simulink library "CryoDetLibCMB"  (R2016b)
settings: Solver=VariableStepAuto  StartTime=0.0  StopTime=10.0  RelTol=1e-3
undefined symbols (not defined in the file): A, B, C, D, Fadc, Fclk, PCIN, xlipgetpartsetting
libraries: xbsIndex_r4 x640, CryoDetLibCMB x81, CryoDetLib x2, simulink x1
(part 2 of 12)

== system CryoDetLibCMB/DAC subSum10_DSP48 ==
  note: Final adder stages
      | divide by 8
      | and reduce to 16 bits
      | add registers to aid timing
  valid : Inport
  In1 : Inport  Port=2
  In2 : Inport  Port=3
  In3 : Inport  Port=4
  In4 : Inport  Port=5
  In5 : Inport  Port=6
  In6 : Inport  Port=7
  In7 : Inport  Port=8
  In8 : Inport  Port=9
  In9 : Inport  Port=10
  In10 : Inport  Port=11
  In11 : Inport  Port=12
  In12 : Inport  Port=13
  In13 : Inport  Port=14
  In14 : Inport  Port=15
  In15 : Inport  Port=16
  In16 : Inport  Port=17
  ch : Inport  Port=18
  r_tone_scale_sel : Inport  Port=19
  Convert1 : xbsIndex_r4/Convert  gui_display_data_type=Fixed-point  arith_type="Signed  (2's comp)"  n_bits=18  bin_pt=17  float_type=Single  exp_bits=8  fraction_bits=24  quantization=Truncate  overflow=Wrap  en=off  latency=0  pipeline=off  dbl_ovrd=off  block_type=convert
  Convert{2..3,5..6} (4 alike) : xbsIndex_r4/Convert  gui_display_data_type=Fixed-point  arith_type="Signed  (2's comp)"  n_bits=19  bin_pt=17  float_type=Single  exp_bits=8  fraction_bits=24  quantization=Truncate  overflow=Wrap  en=off  latency=0  pipeline=off  dbl_ovrd=off  block_type=convert
  Convert4 : xbsIndex_r4/Convert  gui_display_data_type=Fixed-point  arith_type="Signed  (2's comp)"  n_bits=18  bin_pt=17  float_type=Single  exp_bits=8  fraction_bits=24  quantization=Truncate  overflow=Wrap  en=off  latency=0  pipeline=off  dbl_ovrd=off  block_type=convert
  "DSP48 Macro 3.0 " : xbsIndex_r4/DSP48 Macro 3.0   dsptype=Target XtremeDSP Slice: DSP48E2  instruction_list=(A+D)+C  AvailableInstructions=|  show_filtered=off  pipeline_options=Expert  dspimage=?  tier_1=off  tier_2=off  tier_3=off  tier_4=off  tier_5=off  tier_6=off  dreg_1=off  dreg_2=on  dreg_3=on  areg_1=off  areg_2=on  areg_3=on  areg_4=on  breg_1=off  breg_2=off  breg_3=off  breg_4=off  mreg_5=on  concatreg_3=off  concatreg_4=off  concatreg_5=off  creg_1=off  creg_2=on  creg_3=on  creg_4=on  creg_5=on  preg_6=on  cinreg_1=off  cinreg_2=off  cinreg_3=off  cinreg_4=off  cinreg_5=off  opreg_1=off  opreg_2=off  opreg_3=off  opreg_4=off  opreg_5=off  output_properties=Full_Precision  p_width=19  p_binarywidth=15  has_acout=off  has_bcout=off  has_pcout=off  has_carryout=off  has_carrycascout=off  has_ce=off  has_d_ce=off  has_a_ce=off  has_b_ce=off  has_concat_ce=off  has_c_ce=off  has_m_ce=off  has_p_ce=off  has_sel_ce=off  has_sclr=off  has_d_sclr=off  has_a_sclr=off  has_b_sclr=off  has_concat_sclr=off  has_c_sclr=off  has_m_sclr=off  has_p_sclr=off  has_sel_sclr=off  use_dsp48=on  simulation_type=fast_sim  simulation_model=sysgen:xbip_dsp48_macro_v3_0  gui_behaviour=Sysgen  instruction1='#'  ip_name=DSP48 Macro  ip_version=3.0  dsptool_ready=true  ipcore_usecache=true  ipcore_useipmodelcache=true  wrapper_available=true  port_translation_map={ 'ce' => 'en', 'sclr' => 'rst'}  ipcore_latency_function='has_combinational'  structural_sim=false  ipcore_verbose=false  ipcore_port_config={ 'carryin' => { 'arith' => 'ufix', 'binpt' => 0.00000000000, 'width' => 1.00000000000}, 'carrycascin' => { 'arith' => 'ufix', 'binpt' => 0.00000000000, 'width' => 1.00000000000}, 'carrycascout' => { 'arith' => 'ufix', 'binpt' => 0.00000000000, 'width' => 1.00000000000}, 'carryout' => { 'arith' => 'ufix', 'binpt' => 0.00000000000, 'width' => 1.00000000000}}  ipcore_xco_need_fpga_part=true  block_type=xbip_dsp48_macro_v3_0
      | #
      | (A+D)
      | (A+D)*B
      | (A+D)*B+C
      | (A+D)*B+C+C
      | (A+D)*B+C+C+CARRYIN
      | (A+D)*B+C+CARRYIN
      | (A+D)*B+C+P
      | (A+D)*B+C+P+CARRYIN
      | (A+D)*B+C+P>>17
      | (A+D)*B+C+P>>17+CARRYIN
      | (A+D)*B+C+PCIN
      | (A+D)*B+C+PCIN+CARRYIN
      | (A+D)*B+C+PCIN>>17
      | (A+D)*B+C+PCIN>>17+CARRYIN
      | (A+D)*B+C-C
      | (A+D)*B+C-P
      | (A+D)*B+C-P>>17
      | (A+D)*B+C-PCIN
      | (A+D)*B+C-PCIN>>17
      | (A+D)*B+CARRYIN
      | (A+D)*B+P
      | (A+D)*B+P+C
      | (A+D)*B+P+C+CARRYIN
      | (A+D)*B+P+CARRYIN
      | (A+D)*B+P+P
      | (A+D)*B+P+P+CARRYIN
      | (A+D)*B+P+P>>17
      | (A+D)*B+P+P>>17+CARRYIN
      | (A+D)*B+P+PCIN
      | (A+D)*B+P+PCIN+CARRYIN
      | (A+D)*B+P+PCIN>>17
      | (A+D)*B+P+PCIN>>17+CARRYIN
      | (A+D)*B+P-C
      | (A+D)*B+P-P
      | (A+D)*B+P-P>>17
      | (A+D)*B+P-PCIN
      | (A+D)*B+P-PCIN>>17
      | (A+D)*B+P>>17
      | (A+D)*B+P>>17+C
      | (A+D)*B+P>>17+C+CARRYIN
      | (A+D)*B+P>>17+CARRYIN
      | (A+D)*B+P>>17+P
      | (A+D)*B+P>>17+P+CARRYIN
      | (A+D)*B+PCIN
      | (A+D)*B+PCIN+C
      | (A+D)*B+PCIN+C+CARRYIN
      | (A+D)*B+PCIN+CARRYIN
      | (A+D)*B+PCIN+P
      | (A+D)*B+PCIN+P+CARRYIN
      | (A+D)*B+PCIN>>17
      | (A+D)*B+PCIN>>17+C
      | (A+D)*B+PCIN>>17+C+CARRYIN
      | (A+D)*B+PCIN>>17+CARRYIN
      | (A+D)*B+PCIN>>17+P
      | (A+D)*B+PCIN>>17+P+CARRYIN
      | (A+D)*B-C
      | (A+D)*B-P
      | (A+D)*B-P>>17
      | (A+D)*B-PCIN
      | (A+D)*B-PCIN>>17
      | (A+D)+C
      | (A+D)+C+C
      | (A+D)+C+C+CARRYIN
      | (A+D)+C+CARRYIN
      | (A+D)+C+P
      | (A+D)+C+P+CARRYIN
      | (A+D)+C+P>>17
      | (A+D)+C+P>>17+CARRYIN
      | (A+D)+C+PCIN
      | (A+D)+C+PCIN+CARRYIN
      | (A+D)+C+PCIN>>17
      | (A+D)+C+PCIN>>17+CARRYIN
      | (A+D)+C-C
      | (A+D)+C-P
      | (A+D)+C-P>>17
      | (A+D)+C-PCIN
      | (A+D)+C-PCIN>>17
      | (A+D)+CARRYIN
      | (A+D)+P
      | (A+D)+P+C
      | (A+D)+P+C+CARRYIN
      | (A+D)+P+CARRYIN
      | (A+D)+P+P
      | (A+D)+P+P+CARRYIN
      | (A+D)+P+P>>17
      | (A+D)+P+P>>17+CARRYIN
      | (A+D)+P+PCIN
      | (A+D)+P+PCIN+CARRYIN
      | (A+D)+P+PCIN>>17
      | (A+D)+P+PCIN>>17+CARRYIN
      | (A+D)+P-C
      | (A+D)+P-P
      | (A+D)+P-P>>17
      | (A+D)+P-PCIN
      | (A+D)+P-PCIN>>17
      | (A+D)+P>>17
      | (A+D)+P>>17+C
      | (A+D)+P>>17+C+CARRYIN
      | (A+D)+P>>17+CARRYIN
      | (A+D)+P>>17+P
      | (A+D)+P>>17+P+CARRYIN
      | (A+D)+PCIN
      | (A+D)+PCIN+C
      | (A+D)+PCIN+C+CARRYIN
      | (A+D)+PCIN+CARRYIN
      | (A+D)+PCIN+P
      | (A+D)+PCIN+P+CARRYIN
      | (A+D)+PCIN>>17
      | (A+D)+PCIN>>17+C
      | (A+D)+PCIN>>17+C+CARRYIN
      | (A+D)+PCIN>>17+CARRYIN
      | (A+D)+PCIN>>17+P
      | (A+D)+PCIN>>17+P+CARRYIN
      | (A+D)-C
      | (A+D)-P
      | (A+D)-P>>17
      | (A+D)-PCIN
      | (A+D)-PCIN>>17
      | (D+A)
      | (D+A)*B
      | (D+A)*B+C
      | (D+A)*B+C+C
      | (D+A)*B+C+C+CARRYIN
      | (D+A)*B+C+CARRYIN
      | (D+A)*B+C+P
      | (D+A)*B+C+P+CARRYIN
      | (D+A)*B+C+P>>17
      | (D+A)*B+C+P>>17+CARRYIN
      | (D+A)*B+C+PCIN
      | (D+A)*B+C+PCIN+CARRYIN
      | (D+A)*B+C+PCIN>>17
      | (D+A)*B+C+PCIN>>17+CARRYIN
      | (D+A)*B+C-C
      | (D+A)*B+C-P
      | (D+A)*B+C-P>>17
      | (D+A)*B+C-PCIN
      | (D+A)*B+C-PCIN>>17
      | (D+A)*B+CARRYIN
      | (D+A)*B+P
      | (D+A)*B+P+C
      | (D+A)*B+P+C+CARRYIN
      | (D+A)*B+P+CARRYIN
      | (D+A)*B+P+P
      | (D+A)*B+P+P+CARRYIN
      | (D+A)*B+P+P>>17
      | (D+A)*B+P+P>>17+CARRYIN
      | (D+A)*B+P+PCIN
      | (D+A)*B+P+PCIN+CARRYIN
      | (D+A)*B+P+PCIN>>17
      | (D+A)*B+P+PCIN>>17+CARRYIN
      | (D+A)*B+P-C
      | (D+A)*B+P-P
      | (D+A)*B+P-P>>17
      | (D+A)*B+P-PCIN
      | (D+A)*B+P-PCIN>>17
      | (D+A)*B+P>>17
      | (D+A)*B+P>>17+C
      | (D+A)*B+P>>17+C+CARRYIN
      | (D+A)*B+P>>17+CARRYIN
      | (D+A)*B+P>>17+P
      | (D+A)*B+P>>17+P+CARRYIN
      | (D+A)*B+PCIN
      | (D+A)*B+PCIN+C
      | (D+A)*B+PCIN+C+CARRYIN
      | (D+A)*B+PCIN+CARRYIN
      | (D+A)*B+PCIN+P
      | (D+A)*B+PCIN+P+CARRYIN
      | (D+A)*B+PCIN>>17
      | (D+A)*B+PCIN>>17+C
      | (D+A)*B+PCIN>>17+C+CARRYIN
      | (D+A)*B+PCIN>>17+CARRYIN
      | (D+A)*B+PCIN>>17+P
      | (D+A)*B+PCIN>>17+P+CARRYIN
      | (D+A)*B-C
      | (D+A)*B-P
      | (D+A)*B-P>>17
      | (D+A)*B-PCIN
      | (D+A)*B-PCIN>>17
      | (D+A)+C
      | (D+A)+C+C
      | (D+A)+C+C+CARRYIN
      | (D+A)+C+CARRYIN
      | (D+A)+C+P
      | (D+A)+C+P+CARRYIN
      | (D+A)+C+P>>17
      | (D+A)+C+P>>17+CARRYIN
      | (D+A)+C+PCIN
      | (D+A)+C+PCIN+CARRYIN
      | (D+A)+C+PCIN>>17
      | (D+A)+C+PCIN>>17+CARRYIN
      | (D+A)+C-C
      | (D+A)+C-P
      | (D+A)+C-P>>17
      | (D+A)+C-PCIN
      | (D+A)+C-PCIN>>17
      | (D+A)+CARRYIN
      | (D+A)+P
      | (D+A)+P+C
      | (D+A)+P+C+CARRYIN
      | (D+A)+P+CARRYIN
      | (D+A)+P+P
      | (D+A)+P+P+CARRYIN
      | (D+A)+P+P>>17
      | (D+A)+P+P>>17+CARRYIN
      | (D+A)+P+PCIN
      | (D+A)+P+PCIN+CARRYIN
      | (D+A)+P+PCIN>>17
      | (D+A)+P+PCIN>>17+CARRYIN
      | (D+A)+P-C
      | (D+A)+P-P
      | (D+A)+P-P>>17
      | (D+A)+P-PCIN
      | (D+A)+P-PCIN>>17
      | (D+A)+P>>17
      | (D+A)+P>>17+C
      | (D+A)+P>>17+C+CARRYIN
      | (D+A)+P>>17+CARRYIN
      | (D+A)+P>>17+P
      | (D+A)+P>>17+P+CARRYIN
      | (D+A)+PCIN
      | (D+A)+PCIN+C
      | (D+A)+PCIN+C+CARRYIN
      | (D+A)+PCIN+CARRYIN
      | (D+A)+PCIN+P
      | (D+A)+PCIN+P+CARRYIN
      | (D+A)+PCIN>>17
      | (D+A)+PCIN>>17+C
      | (D+A)+PCIN>>17+C+CARRYIN
      | (D+A)+PCIN>>17+CARRYIN
      | (D+A)+PCIN>>17+P
      | (D+A)+PCIN>>17+P+CARRYIN
      | (D+A)-C
      | (D+A)-P
      | (D+A)-P>>17
      | (D+A)-PCIN
      | (D+A)-PCIN>>17
      | (D-A)
      | (D-A)*B
      | (D-A)*B+C
      | (D-A)*B+C+C
      | (D-A)*B+C+C+CARRYIN
      | (D-A)*B+C+CARRYIN
      | (D-A)*B+C+P
      | (D-A)*B+C+P+CARRYIN
      | (D-A)*B+C+P>>17
      | (D-A)*B+C+P>>17+CARRYIN
      | (D-A)*B+C+PCIN
      | (D-A)*B+C+PCIN+CARRYIN
      | (D-A)*B+C+PCIN>>17
      | (D-A)*B+C+PCIN>>17+CARRYIN
      | (D-A)*B+C-C
      | (D-A)*B+C-P
      | (D-A)*B+C-P>>17
      | (D-A)*B+C-PCIN
      | (D-A)*B+C-PCIN>>17
      | (D-A)*B+CARRYIN
      | (D-A)*B+P
      | (D-A)*B+P+C
      | (D-A)*B+P+C+CARRYIN
      | (D-A)*B+P+CARRYIN
      | (D-A)*B+P+P
      | (D-A)*B+P+P+CARRYIN
      | (D-A)*B+P+P>>17
      | (D-A)*B+P+P>>17+CARRYIN
      | (D-A)*B+P+PCIN
      | (D-A)*B+P+PCIN+CARRYIN
      | (D-A)*B+P+PCIN>>17
      | (D-A)*B+P+PCIN>>17+CARRYIN
      | (D-A)*B+P-C
      | (D-A)*B+P-P
      | (D-A)*B+P-P>>17
      | (D-A)*B+P-PCIN
      | (D-A)*B+P-PCIN>>17
      | (D-A)*B+P>>17
      | (D-A)*B+P>>17+C
      | (D-A)*B+P>>17+C+CARRYIN
      | (D-A)*B+P>>17+CARRYIN
      | (D-A)*B+P>>17+P
      | (D-A)*B+P>>17+P+CARRYIN
      | (D-A)*B+PCIN
      | (D-A)*B+PCIN+C
      | (D-A)*B+PCIN+C+CARRYIN
      | (D-A)*B+PCIN+CARRYIN
      | (D-A)*B+PCIN+P
      | (D-A)*B+PCIN+P+CARRYIN
      | (D-A)*B+PCIN>>17
      | (D-A)*B+PCIN>>17+C
      | (D-A)*B+PCIN>>17+C+CARRYIN
      | (D-A)*B+PCIN>>17+CARRYIN
      | (D-A)*B+PCIN>>17+P
      | (D-A)*B+PCIN>>17+P+CARRYIN
      | (D-A)*B-C
      | (D-A)*B-P
      | (D-A)*B-P>>17
      | (D-A)*B-PCIN
      | (D-A)*B-PCIN>>17
      | (D-A)+C
      | (D-A)+C+C
      | (D-A)+C+C+CARRYIN
      | (D-A)+C+CARRYIN
      | (D-A)+C+P
      | (D-A)+C+P+CARRYIN
      | (D-A)+C+P>>17
      | (D-A)+C+P>>17+CARRYIN
      | (D-A)+C+PCIN
      | (D-A)+C+PCIN+CARRYIN
      | (D-A)+C+PCIN>>17
      | (D-A)+C+PCIN>>17+CARRYIN
      | (D-A)+C-C
      | (D-A)+C-P
      | (D-A)+C-P>>17
      | (D-A)+C-PCIN
      | (D-A)+C-PCIN>>17
      | (D-A)+CARRYIN
      | (D-A)+P
      | (D-A)+P+C
      | (D-A)+P+C+CARRYIN
      | (D-A)+P+CARRYIN
      | (D-A)+P+P
      | (D-A)+P+P+CARRYIN
      | (D-A)+P+P>>17
      | (D-A)+P+P>>17+CARRYIN
      | (D-A)+P+PCIN
      | (D-A)+P+PCIN+CARRYIN
      | (D-A)+P+PCIN>>17
      | (D-A)+P+PCIN>>17+CARRYIN
      | (D-A)+P-C
      | (D-A)+P-P
      | (D-A)+P-P>>17
      | (D-A)+P-PCIN
      | (D-A)+P-PCIN>>17
      | (D-A)+P>>17
      | (D-A)+P>>17+C
      | (D-A)+P>>17+C+CARRYIN
      | (D-A)+P>>17+CARRYIN
      | (D-A)+P>>17+P
      | (D-A)+P>>17+P+CARRYIN
      | (D-A)+PCIN
      | (D-A)+PCIN+C
      | (D-A)+PCIN+C+CARRYIN
      | (D-A)+PCIN+CARRYIN
      | (D-A)+PCIN+P
      | (D-A)+PCIN+P+CARRYIN
      | (D-A)+PCIN>>17
      | (D-A)+PCIN>>17+C
      | (D-A)+PCIN>>17+C+CARRYIN
      | (D-A)+PCIN>>17+CARRYIN
      | (D-A)+PCIN>>17+P
      | (D-A)+PCIN>>17+P+CARRYIN
      | (D-A)-C
      | (D-A)-P
      | (D-A)-P>>17
      | (D-A)-PCIN
      | (D-A)-PCIN>>17
      | -((A+D))
      | -((A+D)*B)
      | -((A+D)*B+C)
      | -((A+D)*B+C+CARRYIN)
      | -((A+D)*B+CARRYIN)
      | -((A+D)*B+P)
      | -((A+D)*B+P+CARRYIN)
      | -((A+D)+C)
      | -((A+D)+C+CARRYIN)
      | -((A+D)+CARRYIN)
      | -((A+D)+P)
      | -((A+D)+P+CARRYIN)
      | -((D+A))
      | -((D+A)*B)
      | -((D+A)*B+C)
      | -((D+A)*B+C+CARRYIN)
      | -((D+A)*B+CARRYIN)
      | -((D+A)*B+P)
      | -((D+A)*B+P+CARRYIN)
      | -((D+A)+C)
      | -((D+A)+C+CARRYIN)
      | -((D+A)+CARRYIN)
      | -((D+A)+P)
      | -((D+A)+P+CARRYIN)
      | -((D-A))
      | -((D-A)*B)
      | -((D-A)*B+C)
      | -((D-A)*B+C+CARRYIN)
      | -((D-A)*B+CARRYIN)
      | -((D-A)*B+P)
      | -((D-A)*B+P+CARRYIN)
      | -((D-A)+C)
      | -((D-A)+C+CARRYIN)
      | -((D-A)+CARRYIN)
      | -((D-A)+P)
      | -((D-A)+P+CARRYIN)
      | -(A)
      | -(A*B)
      | -(A*B+C)
      | -(A*B+C+CARRYIN)
      | -(A*B+CARRYIN)
      | -(A*B+P)
      | -(A*B+P+CARRYIN)
      | -(A+C)
      | -(A+C+CARRYIN)
      | -(A+CARRYIN)
      | -(A+D)
      | -(A+D)*B
      | -(A+D)*B-C
      | -(A+D)*B-C-CARRYIN
      | -(A+D)*B-CARRYIN
      | -(A+D)*B-P
      | -(A+D)*B-P-CARRYIN
      | -(A+D)-C
      | -(A+D)-C-CARRYIN
      | -(A+D)-CARRYIN
      | -(A+D)-P
      | -(A+D)-P-CARRYIN
      | -(A+P)
      | -(A+P+CARRYIN)
      | -(B*(A+D))
      | -(B*(A+D)+C)
      | -(B*(A+D)+C+CARRYIN)
      | -(B*(A+D)+CARRYIN)
      | -(B*(A+D)+P)
      | -(B*(A+D)+P+CARRYIN)
      | -(B*(D+A))
      | -(B*(D+A)+C)
      | -(B*(D+A)+C+CARRYIN)
      | -(B*(D+A)+CARRYIN)
      | -(B*(D+A)+P)
      | -(B*(D+A)+P+CARRYIN)
      | -(B*(D-A))
      | -(B*(D-A)+C)
      | -(B*(D-A)+C+CARRYIN)
      | -(B*(D-A)+CARRYIN)
      | -(B*(D-A)+P)
      | -(B*(D-A)+P+CARRYIN)
      | -(B*A)
      | -(B*A+C)
      | -(B*A+C+CARRYIN)
      | -(B*A+CARRYIN)
      | -(B*A+P)
      | -(B*A+P+CARRYIN)
      | -(B*D)
      | -(B*D+C)
      | -(B*D+C+CARRYIN)
      | -(B*D+CARRYIN)
      | -(B*D+P)
      | -(B*D+P+CARRYIN)
      | -(C)
      | -(C+(A+D))
      | -(C+(A+D)*B)
      | -(C+(A+D)*B+CARRYIN)
      | -(C+(A+D)+CARRYIN)
      | -(C+(D+A))
      | -(C+(D+A)*B)
      | -(C+(D+A)*B+CARRYIN)
      | -(C+(D+A)+CARRYIN)
      | -(C+(D-A))
      | -(C+(D-A)*B)
      | -(C+(D-A)*B+CARRYIN)
      | -(C+(D-A)+CARRYIN)
      | -(C+A)
      | -(C+A*B)
      | -(C+A*B+CARRYIN)
      | -(C+A+CARRYIN)
      | -(C+B*(A+D))
      | -(C+B*(A+D)+CARRYIN)
      | -(C+B*(D+A))
      | -(C+B*(D+A)+CARRYIN)
      | -(C+B*(D-A))
      | -(C+B*(D-A)+CARRYIN)
      | -(C+B*A)
      | -(C+B*A+CARRYIN)
      | -(C+B*D)
      | -(C+B*D+CARRYIN)
      | -(C+C)
      | -(C+C+CARRYCASCIN)
      | -(C+C+CARRYIN)
      | -(C+C+P)
      | -(C+C+P+CARRYIN)
      | -(C+CARRYCASCIN)
      | -(C+CARRYIN)
      | -(C+D)
      | -(C+D*B)
      | -(C+D*B+CARRYIN)
      | -(C+D+CARRYIN)
      | -(C+P)
      | -(C+P+C)
      | -(C+P+C+CARRYIN)
      | -(C+P+CARRYCASCIN)
      | -(C+P+CARRYIN)
      | -(C+P+P)
      | -(C+P+P+CARRYIN)
      | -(CARRYIN)
      | -(D)
      | -(D*B)
      | -(D*B+C)
      | -(D*B+C+CARRYIN)
      | -(D*B+CARRYIN)
      | -(D*B+P)
      | -(D*B+P+CARRYIN)
      | -(D+A)
      | -(D+A)*B
      | -(D+A)*B-C
      | -(D+A)*B-C-CARRYIN
      | -(D+A)*B-CARRYIN
      | -(D+A)*B-P
      | -(D+A)*B-P-CARRYIN
      | -(D+A)-C
      | -(D+A)-C-CARRYIN
      | -(D+A)-CARRYIN
      | -(D+A)-P
      | -(D+A)-P-CARRYIN
      | -(D+C)
      | -(D+C+CARRYIN)
      | -(D+CARRYIN)
      | -(D+P)
      | -(D+P+CARRYIN)
      | -(D-A)
      | -(D-A)*B
      | -(D-A)*B-C
      | -(D-A)*B-C-CARRYIN
      | -(D-A)*B-CARRYIN
      | -(D-A)*B-P
      | -(D-A)*B-P-CARRYIN
      | -(D-A)-C
      | -(D-A)-C-CARRYIN
      | -(D-A)-CARRYIN
      | -(D-A)-P
      | -(D-A)-P-CARRYIN
      | -(P)
      | -(P+(A+D))
      | -(P+(A+D)*B)
      | -(P+(A+D)*B+CARRYIN)
      | -(P+(A+D)+CARRYIN)
      | -(P+(D+A))
      | -(P+(D+A)*B)
      | -(P+(D+A)*B+CARRYIN)
      | -(P+(D+A)+CARRYIN)
      | -(P+(D-A))
      | -(P+(D-A)*B)
      | -(P+(D-A)*B+CARRYIN)
      | -(P+(D-A)+CARRYIN)
      | -(P+A)
      | -(P+A*B)
      | -(P+A*B+CARRYIN)
      | -(P+A+CARRYIN)
      | -(P+B*(A+D))
      | -(P+B*(A+D)+CARRYIN)
      | -(P+B*(D+A))
      | -(P+B*(D+A)+CARRYIN)
      | -(P+B*(D-A))
      | -(P+B*(D-A)+CARRYIN)
      | -(P+B*A)
      | -(P+B*A+CARRYIN)
      | -(P+B*D)
      | -(P+B*D+CARRYIN)
      | -(P+C)
      | -(P+C+C)
      | -(P+C+C+CARRYIN)
      | -(P+C+CARRYCASCIN)
      | -(P+C+CARRYIN)
      | -(P+C+P)
      | -(P+C+P+CARRYIN)
      | -(P+CARRYCASCIN)
      | -(P+CARRYIN)
      | -(P+D)
      | -(P+D*B)
      | -(P+D*B+CARRYIN)
      | -(P+D+CARRYIN)
      | -(P+P)
      | -(P+P+C)
      | -(P+P+C+CARRYIN)
      | -(P+P+CARRYCASCIN)
      | -(P+P+CARRYIN)
      | -A
      | -A*B
      | -A*B-C
      | -A*B-C-CARRYIN
      | -A*B-CARRYIN
      | -A*B-P
      | -A*B-P-CARRYIN
      | -A-C
      | -A-C-CARRYIN
      | -A-CARRYIN
      | -A-P
      | -A-P-CARRYIN
      | -B*(A+D)
      | -B*(A+D)-C
      | -B*(A+D)-C-CARRYIN
      | -B*(A+D)-CARRYIN
      | -B*(A+D)-P
      | -B*(A+D)-P-CARRYIN
      | -B*(D+A)
      | -B*(D+A)-C
      | -B*(D+A)-C-CARRYIN
      | -B*(D+A)-CARRYIN
      | -B*(D+A)-P
      | -B*(D+A)-P-CARRYIN
      | -B*(D-A)
      | -B*(D-A)-C
      | -B*(D-A)-C-CARRYIN
      | -B*(D-A)-CARRYIN
      | -B*(D-A)-P
      | -B*(D-A)-P-CARRYIN
      | -B*A
      | -B*A-C
      | -B*A-C-CARRYIN
      | -B*A-CARRYIN
      | -B*A-P
      | -B*A-P-CARRYIN
      | -B*D
      | -B*D-C
      | -B*D-C-CARRYIN
      | -B*D-CARRYIN
      | -B*D-P
      | -B*D-P-CARRYIN
      | -C
      | -C+(A+D)
      | -C+(A+D)*B
      | -C+(A+D)*B+C
      | -C+(A+D)*B+P
      | -C+(A+D)+C
      | -C+(A+D)+P
      | -C+(D+A)
      | -C+(D+A)*B
      | -C+(D+A)*B+C
      | -C+(D+A)*B+P
      | -C+(D+A)+C
      | -C+(D+A)+P
      | -C+(D-A)
      | -C+(D-A)*B
      | -C+(D-A)*B+C
      | -C+(D-A)*B+P
      | -C+(D-A)+C
      | -C+(D-A)+P
      | -C+A
      | -C+A*B
      | -C+A*B+C
      | -C+A*B+P
      | -C+A+C
      | -C+A+P
      | -C+B*(A+D)
      | -C+B*(A+D)+C
      | -C+B*(A+D)+P
      | -C+B*(D+A)
      | -C+B*(D+A)+C
      | -C+B*(D+A)+P
      | -C+B*(D-A)
      | -C+B*(D-A)+C
      | -C+B*(D-A)+P
      | -C+B*A
      | -C+B*A+C
      | -C+B*A+P
      | -C+B*D
      | -C+B*D+C
      | -C+B*D+P
      | -C+C
      | -C+C+(A+D)
      | -C+C+(A+D)*B
      | -C+C+(D+A)
      | -C+C+(D+A)*B
      | -C+C+(D-A)
      | -C+C+(D-A)*B
      | -C+C+A
      | -C+C+A*B
      | -C+C+B*(A+D)
      | -C+C+B*(D+A)
      | -C+C+B*(D-A)
      | -C+C+B*A
      | -C+C+B*D
      | -C+C+C
      | -C+C+C+P
      | -C+C+D
      | -C+C+D*B
      | -C+C+P
      | -C+C+P+C
      | -C+C+P+P
      | -C+D
      | -C+D*B
      | -C+D*B+C
      | -C+D*B+P
      | -C+D+C
      | -C+D+P
      | -C+P
      | -C+P+(A+D)
      | -C+P+(A+D)*B
      | -C+P+(D+A)
      | -C+P+(D+A)*B
      | -C+P+(D-A)
      | -C+P+(D-A)*B
      | -C+P+A
      | -C+P+A*B
      | -C+P+B*(A+D)
      | -C+P+B*(D+A)
      | -C+P+B*(D-A)
      | -C+P+B*A
      | -C+P+B*D
      | -C+P+C
      | -C+P+C+C
      | -C+P+C+P
      | -C+P+D
      | -C+P+D*B
      | -C+P+P
      | -C+P+P+C
      | -C-((A+D))
      | -C-((A+D)*B)
      | -C-((D+A))
      | -C-((D+A)*B)
      | -C-((D-A))
      | -C-((D-A)*B)
      | -C-(A)
      | -C-(A*B)
      | -C-(A+D)
      | -C-(A+D)*B
      | -C-(A+D)*B-CARRYIN
      | -C-(A+D)-CARRYIN
      | -C-(B*(A+D))
      | -C-(B*(D+A))
      | -C-(B*(D-A))
      | -C-(B*A)
      | -C-(B*D)
      | -C-(D)
      | -C-(D*B)
      | -C-(D+A)
      | -C-(D+A)*B
      | -C-(D+A)*B-CARRYIN
      | -C-(D+A)-CARRYIN
      | -C-(D-A)
      | -C-(D-A)*B
      | -C-(D-A)*B-CARRYIN
      | -C-(D-A)-CARRYIN
      | -C-A
      | -C-A*B
      | -C-A*B-CARRYIN
      | -C-A-CARRYIN
      | -C-B*(A+D)
      | -C-B*(A+D)-CARRYIN
      | -C-B*(D+A)
      | -C-B*(D+A)-CARRYIN
      | -C-B*(D-A)
      | -C-B*(D-A)-CARRYIN
      | -C-B*A
      | -C-B*A-CARRYIN
      | -C-B*D
      | -C-B*D-CARRYIN
      | -C-C
      | -C-C-CARRYCASCIN
      | -C-C-CARRYIN
      | -C-C-P
      | -C-C-P-CARRYIN
      | -C-CARRYCASCIN
      | -C-CARRYIN
      | -C-D
      | -C-D*B
      | -C-D*B-CARRYIN
      | -C-D-CARRYIN
      | -C-P
      | -C-P-C
      | -C-P-C-CARRYIN
      | -C-P-CARRYCASCIN
      | -C-P-CARRYIN
      | -C-P-P
      | -C-P-P-CARRYIN
      | -C-P-P>>17
      | -C-P-PCIN
      | -C-P-PCIN>>17
      | -C-P>>17
      | -C-PCIN
      | -C-PCIN>>17
      | -CARRYIN
      | -D
      | -D*B
      | -D*B-C
      | -D*B-C-CARRYIN
      | -D*B-CARRYIN
      | -D*B-P
      | -D*B-P-CARRYIN
      | -D-C
      | -D-C-CARRYIN
      | -D-CARRYIN
      | -D-P
      | -D-P-CARRYIN
      | -P
      | -P+(A+D)
      | -P+(A+D)*B
      | -P+(A+D)*B+C
      | -P+(A+D)*B+P
      | -P+(A+D)+C
      | -P+(A+D)+P
      | -P+(D+A)
      | -P+(D+A)*B
      | -P+(D+A)*B+C
      | -P+(D+A)*B+P
      | -P+(D+A)+C
      | -P+(D+A)+P
      | -P+(D-A)
      | -P+(D-A)*B
      | -P+(D-A)*B+C
      | -P+(D-A)*B+P
      | -P+(D-A)+C
      | -P+(D-A)+P
      | -P+A
      | -P+A*B
      | -P+A*B+C
      | -P+A*B+P
      | -P+A+C
      | -P+A+P
      | -P+B*(A+D)
      | -P+B*(A+D)+C
      | -P+B*(A+D)+P
      | -P+B*(D+A)
      | -P+B*(D+A)+C
      | -P+B*(D+A)+P
      | -P+B*(D-A)
      | -P+B*(D-A)+C
      | -P+B*(D-A)+P
      | -P+B*A
      | -P+B*A+C
      | -P+B*A+P
      | -P+B*D
      | -P+B*D+C
      | -P+B*D+P
      | -P+C
      | -P+C+(A+D)
      | -P+C+(A+D)*B
      | -P+C+(D+A)
      | -P+C+(D+A)*B
      | -P+C+(D-A)
      | -P+C+(D-A)*B
      | -P+C+A
      | -P+C+A*B
      | -P+C+B*(A+D)
      | -P+C+B*(D+A)
      | -P+C+B*(D-A)
      | -P+C+B*A
      | -P+C+B*D
      | -P+C+C
      | -P+C+C+P
      | -P+C+D
      | -P+C+D*B
      | -P+C+P
      | -P+C+P+C
      | -P+C+P+P
      | -P+D
      | -P+D*B
      | -P+D*B+C
      | -P+D*B+P
      | -P+D+C
      | -P+D+P
      | -P+P
      | -P+P+(A+D)
      | -P+P+(A+D)*B
      | -P+P+(D+A)
      | -P+P+(D+A)*B
      | -P+P+(D-A)
      | -P+P+(D-A)*B
      | -P+P+A
      | -P+P+A*B
      | -P+P+B*(A+D)
      | -P+P+B*(D+A)
      | -P+P+B*(D-A)
      | -P+P+B*A
      | -P+P+B*D
      | -P+P+C
      | -P+P+C+C
      | -P+P+C+P
      | -P+P+D
      | -P+P+D*B
      | -P+P+P
      | -P+P+P+C
      | -P-((A+D))
      | -P-((A+D)*B)
      | -P-((D+A))
      | -P-((D+A)*B)
      | -P-((D-A))
      | -P-((D-A)*B)
      | -P-(A)
      | -P-(A*B)
      | -P-(A+D)
      | -P-(A+D)*B
      | -P-(A+D)*B-CARRYIN
      | -P-(A+D)-CARRYIN
      | -P-(B*(A+D))
      | -P-(B*(D+A))
      | -P-(B*(D-A))
      | -P-(B*A)
      | -P-(B*D)
      | -P-(D)
      | -P-(D*B)
      | -P-(D+A)
      | -P-(D+A)*B
      | -P-(D+A)*B-CARRYIN
      | -P-(D+A)-CARRYIN
      | -P-(D-A)
      | -P-(D-A)*B
      | -P-(D-A)*B-CARRYIN
      | -P-(D-A)-CARRYIN
      | -P-A
      | -P-A*B
      | -P-A*B-CARRYIN
      | -P-A-CARRYIN
      | -P-B*(A+D)
      | -P-B*(A+D)-CARRYIN
      | -P-B*(D+A)
      | -P-B*(D+A)-CARRYIN
      | -P-B*(D-A)
      | -P-B*(D-A)-CARRYIN
      | -P-B*A
      | -P-B*A-CARRYIN
      | -P-B*D
      | -P-B*D-CARRYIN
      | -P-C
      | -P-C-C
      | -P-C-C-CARRYIN
      | -P-C-CARRYCASCIN
      | -P-C-CARRYIN
      | -P-C-P
      | -P-C-P-CARRYIN
      | -P-C-P>>17
      | -P-C-PCIN
      | -P-C-PCIN>>17
      | -P-CARRYCASCIN
      | -P-CARRYIN
      | -P-D
      | -P-D*B
      | -P-D*B-CARRYIN
      | -P-D-CARRYIN
      | -P-P
      | -P-P-C
      | -P-P-C-CARRYIN
      | -P-P-CARRYCASCIN
      | -P-P-CARRYIN
      | -P-P-P
      | -P-P-P>>17
      | -P-P-PCIN
      | -P-P-PCIN>>17
      | -P-P>>17
      | -P-PCIN
      | -P-PCIN>>17
      | -P>>17
      | -P>>17+(A+D)
      | -P>>17+(A+D)*B
      | -P>>17+(A+D)*B+C
      | -P>>17+(A+D)*B+P
      | -P>>17+(A+D)+C
      | -P>>17+(A+D)+P
      | -P>>17+(D+A)
      | -P>>17+(D+A)*B
      | -P>>17+(D+A)*B+C
      | -P>>17+(D+A)*B+P
      | -P>>17+(D+A)+C
      | -P>>17+(D+A)+P
      | -P>>17+(D-A)
      | -P>>17+(D-A)*B
      | -P>>17+(D-A)*B+C
      | -P>>17+(D-A)*B+P
      | -P>>17+(D-A)+C
      | -P>>17+(D-A)+P
      | -P>>17+A
      | -P>>17+A*B
      | -P>>17+A*B+C
      | -P>>17+A*B+P
      | -P>>17+A+C
      | -P>>17+A+P
      | -P>>17+B*(A+D)
      | -P>>17+B*(A+D)+C
      | -P>>17+B*(A+D)+P
      | -P>>17+B*(D+A)
      | -P>>17+B*(D+A)+C
      | -P>>17+B*(D+A)+P
      | -P>>17+B*(D-A)
      | -P>>17+B*(D-A)+C
      | -P>>17+B*(D-A)+P
      | -P>>17+B*A
      | -P>>17+B*A+C
      | -P>>17+B*A+P
      | -P>>17+B*D
      | -P>>17+B*D+C
      | -P>>17+B*D+P
      | -P>>17+C
      | -P>>17+C+(A+D)
      | -P>>17+C+(A+D)*B
      | -P>>17+C+(D+A)
      | -P>>17+C+(D+A)*B
      | -P>>17+C+(D-A)
      | -P>>17+C+(D-A)*B
      | -P>>17+C+A
      | -P>>17+C+A*B
      | -P>>17+C+B*(A+D)
      | -P>>17+C+B*(D+A)
      | -P>>17+C+B*(D-A)
      | -P>>17+C+B*A
      | -P>>17+C+B*D
      | -P>>17+C+C
      | -P>>17+C+C+P
      | -P>>17+C+D
      | -P>>17+C+D*B
      | -P>>17+C+P
      | -P>>17+C+P+C
      | -P>>17+C+P+P
      | -P>>17+D
      | -P>>17+D*B
      | -P>>17+D*B+C
      | -P>>17+D*B+P
      | -P>>17+D+C
      | -P>>17+D+P
      | -P>>17+P
      | -P>>17+P+(A+D)
      | -P>>17+P+(A+D)*B
      | -P>>17+P+(D+A)
      | -P>>17+P+(D+A)*B
      | -P>>17+P+(D-A)
      | -P>>17+P+(D-A)*B
      | -P>>17+P+A
      | -P>>17+P+A*B
      | -P>>17+P+B*(A+D)
      | -P>>17+P+B*(D+A)
      | -P>>17+P+B*(D-A)
      | -P>>17+P+B*A
      | -P>>17+P+B*D
      | -P>>17+P+C
      | -P>>17+P+C+C
      | -P>>17+P+C+P
      | -P>>17+P+D
      | -P>>17+P+D*B
      | -P>>17+P+P
      | -P>>17+P+P+C
      | -P>>17-((A+D))
      | -P>>17-((A+D)*B)
      | -P>>17-((D+A))
      | -P>>17-((D+A)*B)
      | -P>>17-((D-A))
      | -P>>17-((D-A)*B)
      | -P>>17-(A)
      | -P>>17-(A*B)
      | -P>>17-(B*(A+D))
      | -P>>17-(B*(D+A))
      | -P>>17-(B*(D-A))
      | -P>>17-(B*A)
      | -P>>17-(B*D)
      | -P>>17-(D)
      | -P>>17-(D*B)
      | -PCIN
      | -PCIN+(A+D)
      | -PCIN+(A+D)*B
      | -PCIN+(A+D)*B+C
      | -PCIN+(A+D)*B+P
      | -PCIN+(A+D)+C
      | -PCIN+(A+D)+P
      | -PCIN+(D+A)
      | -PCIN+(D+A)*B
      | -PCIN+(D+A)*B+C
      | -PCIN+(D+A)*B+P
      | -PCIN+(D+A)+C
      | -PCIN+(D+A)+P
      | -PCIN+(D-A)
      | -PCIN+(D-A)*B
      | -PCIN+(D-A)*B+C
      | -PCIN+(D-A)*B+P
      | -PCIN+(D-A)+C
      | -PCIN+(D-A)+P
      | -PCIN+A
      | -PCIN+A*B
      | -PCIN+A*B+C
      | -PCIN+A*B+P
      | -PCIN+A+C
      | -PCIN+A+P
      | -PCIN+B*(A+D)
      | -PCIN+B*(A+D)+C
      | -PCIN+B*(A+D)+P
      | -PCIN+B*(D+A)
      | -PCIN+B*(D+A)+C
      | -PCIN+B*(D+A)+P
      | -PCIN+B*(D-A)
      | -PCIN+B*(D-A)+C
      | -PCIN+B*(D-A)+P
      | -PCIN+B*A
      | -PCIN+B*A+C
      | -PCIN+B*A+P
      | -PCIN+B*D
      | -PCIN+B*D+C
      | -PCIN+B*D+P
      | -PCIN+C
      | -PCIN+C+(A+D)
      | -PCIN+C+(A+D)*B
      | -PCIN+C+(D+A)
      | -PCIN+C+(D+A)*B
      | -PCIN+C+(D-A)
      | -PCIN+C+(D-A)*B
      | -PCIN+C+A
      | -PCIN+C+A*B
      | -PCIN+C+B*(A+D)
      | -PCIN+C+B*(D+A)
      | -PCIN+C+B*(D-A)
      | -PCIN+C+B*A
      | -PCIN+C+B*D
      | -PCIN+C+C
      | -PCIN+C+C+P
      | -PCIN+C+D
      | -PCIN+C+D*B
      | -PCIN+C+P
      | -PCIN+C+P+C
      | -PCIN+C+P+P
      | -PCIN+D
      | -PCIN+D*B
      | -PCIN+D*B+C
      | -PCIN+D*B+P
      | -PCIN+D+C
      | -PCIN+D+P
      | -PCIN+P
      | -PCIN+P+(A+D)
      | -PCIN+P+(A+D)*B
      | -PCIN+P+(D+A)
      | -PCIN+P+(D+A)*B
      | -PCIN+P+(D-A)
      | -PCIN+P+(D-A)*B
      | -PCIN+P+A
      | -PCIN+P+A*B
      | -PCIN+P+B*(A+D)
      | -PCIN+P+B*(D+A)
      | -PCIN+P+B*(D-A)
      | -PCIN+P+B*A
      | -PCIN+P+B*D
      | -PCIN+P+C
      | -PCIN+P+C+C
      | -PCIN+P+C+P
      | -PCIN+P+D
      | -PCIN+P+D*B
      | -PCIN+P+P
      | -PCIN+P+P+C
      | -PCIN-((A+D))
      | -PCIN-((A+D)*B)
      | -PCIN-((D+A))
      | -PCIN-((D+A)*B)
      | -PCIN-((D-A))
      | -PCIN-((D-A)*B)
      | -PCIN-(A)
      | -PCIN-(A*B)
      | -PCIN-(B*(A+D))
      | -PCIN-(B*(D+A))
      | -PCIN-(B*(D-A))
      | -PCIN-(B*A)
      | -PCIN-(B*D)
      | -PCIN-(D)
      | -PCIN-(D*B)
      | -PCIN>>17
      | -PCIN>>17+(A+D)
      | -PCIN>>17+(A+D)*B
      | -PCIN>>17+(A+D)*B+C
      | -PCIN>>17+(A+D)*B+P
      | -PCIN>>17+(A+D)+C
      | -PCIN>>17+(A+D)+P
      | -PCIN>>17+(D+A)
      | -PCIN>>17+(D+A)*B
      | -PCIN>>17+(D+A)*B+C
      | -PCIN>>17+(D+A)*B+P
      | -PCIN>>17+(D+A)+C
      | -PCIN>>17+(D+A)+P
      | -PCIN>>17+(D-A)
      | -PCIN>>17+(D-A)*B
      | -PCIN>>17+(D-A)*B+C
      | -PCIN>>17+(D-A)*B+P
      | -PCIN>>17+(D-A)+C
      | -PCIN>>17+(D-A)+P
      | -PCIN>>17+A
      | -PCIN>>17+A*B
      | -PCIN>>17+A*B+C
      | -PCIN>>17+A*B+P
      | -PCIN>>17+A+C
      | -PCIN>>17+A+P
      | -PCIN>>17+B*(A+D)
      | -PCIN>>17+B*(A+D)+C
      | -PCIN>>17+B*(A+D)+P
      | -PCIN>>17+B*(D+A)
      | -PCIN>>17+B*(D+A)+C
      | -PCIN>>17+B*(D+A)+P
      | -PCIN>>17+B*(D-A)
      | -PCIN>>17+B*(D-A)+C
      | -PCIN>>17+B*(D-A)+P
      | -PCIN>>17+B*A
      | -PCIN>>17+B*A+C
      | -PCIN>>17+B*A+P
      | -PCIN>>17+B*D
      | -PCIN>>17+B*D+C
      | -PCIN>>17+B*D+P
      | -PCIN>>17+C
      | -PCIN>>17+C+(A+D)
      | -PCIN>>17+C+(A+D)*B
      | -PCIN>>17+C+(D+A)
      | -PCIN>>17+C+(D+A)*B
      | -PCIN>>17+C+(D-A)
      | -PCIN>>17+C+(D-A)*B
      | -PCIN>>17+C+A
      | -PCIN>>17+C+A*B
      | -PCIN>>17+C+B*(A+D)
      | -PCIN>>17+C+B*(D+A)
      | -PCIN>>17+C+B*(D-A)
      | -PCIN>>17+C+B*A
      | -PCIN>>17+C+B*D
      | -PCIN>>17+C+C
      | -PCIN>>17+C+C+P
      | -PCIN>>17+C+D
      | -PCIN>>17+C+D*B
      | -PCIN>>17+C+P
      | -PCIN>>17+C+P+C
      | -PCIN>>17+C+P+P
      | -PCIN>>17+D
      | -PCIN>>17+D*B
      | -PCIN>>17+D*B+C
      | -PCIN>>17+D*B+P
      | -PCIN>>17+D+C
      | -PCIN>>17+D+P
      | -PCIN>>17+P
      | -PCIN>>17+P+(A+D)
      | -PCIN>>17+P+(A+D)*B
      | -PCIN>>17+P+(D+A)
      | -PCIN>>17+P+(D+A)*B
      | -PCIN>>17+P+(D-A)
      | -PCIN>>17+P+(D-A)*B
      | -PCIN>>17+P+A
      | -PCIN>>17+P+A*B
      | -PCIN>>17+P+B*(A+D)
      | -PCIN>>17+P+B*(D+A)
      | -PCIN>>17+P+B*(D-A)
      | -PCIN>>17+P+B*A
      | -PCIN>>17+P+B*D
      | -PCIN>>17+P+C
      | -PCIN>>17+P+C+C
      | -PCIN>>17+P+C+P
      | -PCIN>>17+P+D
      | -PCIN>>17+P+D*B
      | -PCIN>>17+P+P
      | -PCIN>>17+P+P+C
      | -PCIN>>17-((A+D))
      | -PCIN>>17-((A+D)*B)
      | -PCIN>>17-((D+A))
      | -PCIN>>17-((D+A)*B)
      | -PCIN>>17-((D-A))
      | -PCIN>>17-((D-A)*B)
      | -PCIN>>17-(A)
      | -PCIN>>17-(A*B)
      | -PCIN>>17-(B*(A+D))
      | -PCIN>>17-(B*(D+A))
      | -PCIN>>17-(B*(D-A))
      | -PCIN>>17-(B*A)
      | -PCIN>>17-(B*D)
      | -PCIN>>17-(D)
      | -PCIN>>17-(D*B)
      | 0
      | A
      | A*B
      | A*B+C
      | A*B+C+C
      | A*B+C+C+CARRYIN
      | A*B+C+CARRYIN
      | A*B+C+P
      | A*B+C+P+CARRYIN
      | A*B+C+P>>17
      | A*B+C+P>>17+CARRYIN
      | A*B+C+PCIN
      | A*B+C+PCIN+CARRYIN
      | A*B+C+PCIN>>17
      | A*B+C+PCIN>>17+CARRYIN
      | A*B+C-C
      | A*B+C-P
      | A*B+C-P>>17
      | A*B+C-PCIN
      | A*B+C-PCIN>>17
      | A*B+CARRYIN
      | A*B+P
      | A*B+P+C
      | A*B+P+C+CARRYIN
      | A*B+P+CARRYIN
      | A*B+P+P
      | A*B+P+P+CARRYIN
      | A*B+P+P>>17
      | A*B+P+P>>17+CARRYIN
      | A*B+P+PCIN
      | A*B+P+PCIN+CARRYIN
      | A*B+P+PCIN>>17
      | A*B+P+PCIN>>17+CARRYIN
      | A*B+P-C
      | A*B+P-P
      | A*B+P-P>>17
      | A*B+P-PCIN
      | A*B+P-PCIN>>17
      | A*B+P>>17
      | A*B+P>>17+C
      | A*B+P>>17+C+CARRYIN
      | A*B+P>>17+CARRYIN
      | A*B+P>>17+P
      | A*B+P>>17+P+CARRYIN
      | A*B+PCIN
      | A*B+PCIN+C
      | A*B+PCIN+C+CARRYIN
      | A*B+PCIN+CARRYIN
      | A*B+PCIN+P
      | A*B+PCIN+P+CARRYIN
      | A*B+PCIN>>17
      | A*B+PCIN>>17+C
      | A*B+PCIN>>17+C+CARRYIN
      | A*B+PCIN>>17+CARRYIN
      | A*B+PCIN>>17+P
      | A*B+PCIN>>17+P+CARRYIN
      | A*B-C
      | A*B-P
      | A*B-P>>17
      | A*B-PCIN
      | A*B-PCIN>>17
      | A+C
      | A+C+C
      | A+C+C+CARRYIN
      | A+C+CARRYIN
      | A+C+P
      | A+C+P+CARRYIN
      | A+C+P>>17
      | A+C+P>>17+CARRYIN
      | A+C+PCIN
      | A+C+PCIN+CARRYIN
      | A+C+PCIN>>17
      | A+C+PCIN>>17+CARRYIN
      | A+C-C
      | A+C-P
      | A+C-P>>17
      | A+C-PCIN
      | A+C-PCIN>>17
      | A+CARRYIN
      | A+P
      | A+P+C
      | A+P+C+CARRYIN
      | A+P+CARRYIN
      | A+P+P
      | A+P+P+CARRYIN
      | A+P+P>>17
      | A+P+P>>17+CARRYIN
      | A+P+PCIN
      | A+P+PCIN+CARRYIN
      | A+P+PCIN>>17
      | A+P+PCIN>>17+CARRYIN
      | A+P-C
      | A+P-P
      | A+P-P>>17
      | A+P-PCIN
      | A+P-PCIN>>17
      | A+P>>17
      | A+P>>17+C
      | A+P>>17+C+CARRYIN
      | A+P>>17+CARRYIN
      | A+P>>17+P
      | A+P>>17+P+CARRYIN
      | A+PCIN
      | A+PCIN+C
      | A+PCIN+C+CARRYIN
      | A+PCIN+CARRYIN
      | A+PCIN+P
      | A+PCIN+P+CARRYIN
      | A+PCIN>>17
      | A+PCIN>>17+C
      | A+PCIN>>17+C+CARRYIN
      | A+PCIN>>17+CARRYIN
      | A+PCIN>>17+P
      | A+PCIN>>17+P+CARRYIN
      | A-C
      | A-P
      | A-P>>17
      | A-PCIN
      | A-PCIN>>17
      | B*(A+D)
      | B*(A+D)+C
      | B*(A+D)+C+C
      | B*(A+D)+C+C+CARRYIN
      | B*(A+D)+C+CARRYIN
      | B*(A+D)+C+P
      | B*(A+D)+C+P+CARRYIN
      | B*(A+D)+C+P>>17
      | B*(A+D)+C+P>>17+CARRYIN
      | B*(A+D)+C+PCIN
      | B*(A+D)+C+PCIN+CARRYIN
      | B*(A+D)+C+PCIN>>17
      | B*(A+D)+C+PCIN>>17+CARRYIN
      | B*(A+D)+C-C
      | B*(A+D)+C-P
      | B*(A+D)+C-P>>17
      | B*(A+D)+C-PCIN
      | B*(A+D)+C-PCIN>>17
      | B*(A+D)+CARRYIN
      | B*(A+D)+P
      | B*(A+D)+P+C
      | B*(A+D)+P+C+CARRYIN
      | B*(A+D)+P+CARRYIN
      | B*(A+D)+P+P
      | B*(A+D)+P+P+CARRYIN
      | B*(A+D)+P+P>>17
      | B*(A+D)+P+P>>17+CARRYIN
      | B*(A+D)+P+PCIN
      | B*(A+D)+P+PCIN+CARRYIN
      | B*(A+D)+P+PCIN>>17
      | B*(A+D)+P+PCIN>>17+CARRYIN
      | B*(A+D)+P-C
      | B*(A+D)+P-P
      | B*(A+D)+P-P>>17
      | B*(A+D)+P-PCIN
      | B*(A+D)+P-PCIN>>17
      | B*(A+D)+P>>17
      | B*(A+D)+P>>17+C
      | B*(A+D)+P>>17+C+CARRYIN
      | B*(A+D)+P>>17+CARRYIN
      | B*(A+D)+P>>17+P
      | B*(A+D)+P>>17+P+CARRYIN
      | B*(A+D)+PCIN
      | B*(A+D)+PCIN+C
      | B*(A+D)+PCIN+C+CARRYIN
      | B*(A+D)+PCIN+CARRYIN
      | B*(A+D)+PCIN+P
      | B*(A+D)+PCIN+P+CARRYIN
      | B*(A+D)+PCIN>>17
      | B*(A+D)+PCIN>>17+C
      | B*(A+D)+PCIN>>17+C+CARRYIN
      | B*(A+D)+PCIN>>17+CARRYIN
      | B*(A+D)+PCIN>>17+P
      | B*(A+D)+PCIN>>17+P+CARRYIN
      | B*(A+D)-C
      | B*(A+D)-P
      | B*(A+D)-P>>17
      | B*(A+D)-PCIN
      | B*(A+D)-PCIN>>17
      | B*(D+A)
      | B*(D+A)+C
      | B*(D+A)+C+C
      | B*(D+A)+C+C+CARRYIN
      | B*(D+A)+C+CARRYIN
      | B*(D+A)+C+P
      | B*(D+A)+C+P+CARRYIN
      | B*(D+A)+C+P>>17
      | B*(D+A)+C+P>>17+CARRYIN
      | B*(D+A)+C+PCIN
      | B*(D+A)+C+PCIN+CARRYIN
      | B*(D+A)+C+PCIN>>17
      | B*(D+A)+C+PCIN>>17+CARRYIN
      | B*(D+A)+C-C
      | B*(D+A)+C-P
      | B*(D+A)+C-P>>17
      | B*(D+A)+C-PCIN
      | B*(D+A)+C-PCIN>>17
      | B*(D+A)+CARRYIN
      | B*(D+A)+P
      | B*(D+A)+P+C
      | B*(D+A)+P+C+CARRYIN
      | B*(D+A)+P+CARRYIN
      | B*(D+A)+P+P
      | B*(D+A)+P+P+CARRYIN
      | B*(D+A)+P+P>>17
      | B*(D+A)+P+P>>17+CARRYIN
      | B*(D+A)+P+PCIN
      | B*(D+A)+P+PCIN+CARRYIN
      | B*(D+A)+P+PCIN>>17
      | B*(D+A)+P+PCIN>>17+CARRYIN
      | B*(D+A)+P-C
      | B*(D+A)+P-P
      | B*(D+A)+P-P>>17
      | B*(D+A)+P-PCIN
      | B*(D+A)+P-PCIN>>17
      | B*(D+A)+P>>17
      | B*(D+A)+P>>17+C
      | B*(D+A)+P>>17+C+CARRYIN
      | B*(D+A)+P>>17+CARRYIN
      | B*(D+A)+P>>17+P
      | B*(D+A)+P>>17+P+CARRYIN
      | B*(D+A)+PCIN
      | B*(D+A)+PCIN+C
      | B*(D+A)+PCIN+C+CARRYIN
      | B*(D+A)+PCIN+CARRYIN
      | B*(D+A)+PCIN+P
      | B*(D+A)+PCIN+P+CARRYIN
      | B*(D+A)+PCIN>>17
      | B*(D+A)+PCIN>>17+C
      | B*(D+A)+PCIN>>17+C+CARRYIN
      | B*(D+A)+PCIN>>17+CARRYIN
      | B*(D+A)+PCIN>>17+P
      | B*(D+A)+PCIN>>17+P+CARRYIN
      | B*(D+A)-C
      | B*(D+A)-P
      | B*(D+A)-P>>17
      | B*(D+A)-PCIN
      | B*(D+A)-PCIN>>17
      | B*(D-A)
      | B*(D-A)+C
      | B*(D-A)+C+C
      | B*(D-A)+C+C+CARRYIN
      | B*(D-A)+C+CARRYIN
      | B*(D-A)+C+P
      | B*(D-A)+C+P+CARRYIN
      | B*(D-A)+C+P>>17
      | B*(D-A)+C+P>>17+CARRYIN
      | B*(D-A)+C+PCIN
      | B*(D-A)+C+PCIN+CARRYIN
      | B*(D-A)+C+PCIN>>17
      | B*(D-A)+C+PCIN>>17+CARRYIN
      | B*(D-A)+C-C
      | B*(D-A)+C-P
      | B*(D-A)+C-P>>17
      | B*(D-A)+C-PCIN
      | B*(D-A)+C-PCIN>>17
      | B*(D-A)+CARRYIN
      | B*(D-A)+P
      | B*(D-A)+P+C
      | B*(D-A)+P+C+CARRYIN
      | B*(D-A)+P+CARRYIN
      | B*(D-A)+P+P
      | B*(D-A)+P+P+CARRYIN
      | B*(D-A)+P+P>>17
      | B*(D-A)+P+P>>17+CARRYIN
      | B*(D-A)+P+PCIN
      | B*(D-A)+P+PCIN+CARRYIN
      | B*(D-A)+P+PCIN>>17
      | B*(D-A)+P+PCIN>>17+CARRYIN
      | B*(D-A)+P-C
      | B*(D-A)+P-P
      | B*(D-A)+P-P>>17
      | B*(D-A)+P-PCIN
      | B*(D-A)+P-PCIN>>17
      | B*(D-A)+P>>17
      | B*(D-A)+P>>17+C
      | B*(D-A)+P>>17+C+CARRYIN
      | B*(D-A)+P>>17+CARRYIN
      | B*(D-A)+P>>17+P
      | B*(D-A)+P>>17+P+CARRYIN
      | B*(D-A)+PCIN
      | B*(D-A)+PCIN+C
      | B*(D-A)+PCIN+C+CARRYIN
      | B*(D-A)+PCIN+CARRYIN
      | B*(D-A)+PCIN+P
      | B*(D-A)+PCIN+P+CARRYIN
      | B*(D-A)+PCIN>>17
      | B*(D-A)+PCIN>>17+C
      | B*(D-A)+PCIN>>17+C+CARRYIN
      | B*(D-A)+PCIN>>17+CARRYIN
      | B*(D-A)+PCIN>>17+P
      | B*(D-A)+PCIN>>17+P+CARRYIN
      | B*(D-A)-C
      | B*(D-A)-P
      | B*(D-A)-P>>17
      | B*(D-A)-PCIN
      | B*(D-A)-PCIN>>17
      | B*A
      | B*A+C
      | B*A+C+C
      | B*A+C+C+CARRYIN
      | B*A+C+CARRYIN
      | B*A+C+P
      | B*A+C+P+CARRYIN
      | B*A+C+P>>17
      | B*A+C+P>>17+CARRYIN
      | B*A+C+PCIN
      | B*A+C+PCIN+CARRYIN
      | B*A+C+PCIN>>17
      | B*A+C+PCIN>>17+CARRYIN
      | B*A+C-C
      | B*A+C-P
      | B*A+C-P>>17
      | B*A+C-PCIN
      | B*A+C-PCIN>>17
      | B*A+CARRYIN
      | B*A+P
      | B*A+P+C
      | B*A+P+C+CARRYIN
      | B*A+P+CARRYIN
      | B*A+P+P
      | B*A+P+P+CARRYIN
      | B*A+P+P>>17
      | B*A+P+P>>17+CARRYIN
      | B*A+P+PCIN
      | B*A+P+PCIN+CARRYIN
      | B*A+P+PCIN>>17
      | B*A+P+PCIN>>17+CARRYIN
      | B*A+P-C
      | B*A+P-P
      | B*A+P-P>>17
      | B*A+P-PCIN
      | B*A+P-PCIN>>17
      | B*A+P>>17
      | B*A+P>>17+C
      | B*A+P>>17+C+CARRYIN
      | B*A+P>>17+CARRYIN
      | B*A+P>>17+P
      | B*A+P>>17+P+CARRYIN
      | B*A+PCIN
      | B*A+PCIN+C
      | B*A+PCIN+C+CARRYIN
      | B*A+PCIN+CARRYIN
      | B*A+PCIN+P
      | B*A+PCIN+P+CARRYIN
      | B*A+PCIN>>17
      | B*A+PCIN>>17+C
      | B*A+PCIN>>17+C+CARRYIN
      | B*A+PCIN>>17+CARRYIN
      | B*A+PCIN>>17+P
      | B*A+PCIN>>17+P+CARRYIN
      | B*A-C
      | B*A-P
      | B*A-P>>17
      | B*A-PCIN
      | B*A-PCIN>>17
      | B*D
      | B*D+C
      | B*D+C+C
      | B*D+C+C+CARRYIN
      | B*D+C+CARRYIN
      | B*D+C+P
      | B*D+C+P+CARRYIN
      | B*D+C+P>>17
      | B*D+C+P>>17+CARRYIN
      | B*D+C+PCIN
      | B*D+C+PCIN+CARRYIN
      | B*D+C+PCIN>>17
      | B*D+C+PCIN>>17+CARRYIN
      | B*D+C-C
      | B*D+C-P
      | B*D+C-P>>17
      | B*D+C-PCIN
      | B*D+C-PCIN>>17
      | B*D+CARRYIN
      | B*D+P
      | B*D+P+C
      | B*D+P+C+CARRYIN
      | B*D+P+CARRYIN
      | B*D+P+P
      | B*D+P+P+CARRYIN
      | B*D+P+P>>17
      | B*D+P+P>>17+CARRYIN
      | B*D+P+PCIN
      | B*D+P+PCIN+CARRYIN
      | B*D+P+PCIN>>17
      | B*D+P+PCIN>>17+CARRYIN
      | B*D+P-C
      | B*D+P-P
      | B*D+P-P>>17
      | B*D+P-PCIN
      | B*D+P-PCIN>>17
      | B*D+P>>17
      | B*D+P>>17+C
      | B*D+P>>17+C+CARRYIN
      | B*D+P>>17+CARRYIN
      | B*D+P>>17+P
      | B*D+P>>17+P+CARRYIN
      | B*D+PCIN
      | B*D+PCIN+C
      | B*D+PCIN+C+CARRYIN
      | B*D+PCIN+CARRYIN
      | B*D+PCIN+P
      | B*D+PCIN+P+CARRYIN
      | B*D+PCIN>>17
      | B*D+PCIN>>17+C
      | B*D+PCIN>>17+C+CARRYIN
      | B*D+PCIN>>17+CARRYIN
      | B*D+PCIN>>17+P
      | B*D+PCIN>>17+P+CARRYIN
      | B*D-C
      | B*D-P
      | B*D-P>>17
      | B*D-PCIN
      | B*D-PCIN>>17
      | C
      | C+(A+D)
      | C+(A+D)*B
      | C+(A+D)*B+C
      | C+(A+D)*B+C+CARRYIN
      | C+(A+D)*B+CARRYIN
      | C+(A+D)*B+P
      | C+(A+D)*B+P+CARRYIN
      | C+(A+D)*B+P>>17
      | C+(A+D)*B+P>>17+CARRYIN
      | C+(A+D)*B+PCIN
      | C+(A+D)*B+PCIN+CARRYIN
      | C+(A+D)*B+PCIN>>17
      | C+(A+D)*B+PCIN>>17+CARRYIN
      | C+(A+D)*B-C
      | C+(A+D)*B-P
      | C+(A+D)*B-P>>17
      | C+(A+D)*B-PCIN
      | C+(A+D)*B-PCIN>>17
      | C+(A+D)+C
      | C+(A+D)+C+CARRYIN
      | C+(A+D)+CARRYIN
      | C+(A+D)+P
      | C+(A+D)+P+CARRYIN
      | C+(A+D)+P>>17
      | C+(A+D)+P>>17+CARRYIN
      | C+(A+D)+PCIN
      | C+(A+D)+PCIN+CARRYIN
      | C+(A+D)+PCIN>>17
      | C+(A+D)+PCIN>>17+CARRYIN
      | C+(A+D)-C
      | C+(A+D)-P
      | C+(A+D)-P>>17
      | C+(A+D)-PCIN
      | C+(A+D)-PCIN>>17
      | C+(D+A)
      | C+(D+A)*B
      | C+(D+A)*B+C
      | C+(D+A)*B+C+CARRYIN
      | C+(D+A)*B+CARRYIN
      | C+(D+A)*B+P
      | C+(D+A)*B+P+CARRYIN
      | C+(D+A)*B+P>>17
      | C+(D+A)*B+P>>17+CARRYIN
      | C+(D+A)*B+PCIN
      | C+(D+A)*B+PCIN+CARRYIN
      | C+(D+A)*B+PCIN>>17
      | C+(D+A)*B+PCIN>>17+CARRYIN
      | C+(D+A)*B-C
      | C+(D+A)*B-P
      | C+(D+A)*B-P>>17
      | C+(D+A)*B-PCIN
      | C+(D+A)*B-PCIN>>17
      | C+(D+A)+C
      | C+(D+A)+C+CARRYIN
      | C+(D+A)+CARRYIN
      | C+(D+A)+P
      | C+(D+A)+P+CARRYIN
      | C+(D+A)+P>>17
      | C+(D+A)+P>>17+CARRYIN
      | C+(D+A)+PCIN
      | C+(D+A)+PCIN+CARRYIN
      | C+(D+A)+PCIN>>17
      | C+(D+A)+PCIN>>17+CARRYIN
      | C+(D+A)-C
      | C+(D+A)-P
      | C+(D+A)-P>>17
      | C+(D+A)-PCIN
      | C+(D+A)-PCIN>>17
      | C+(D-A)
      | C+(D-A)*B
      | C+(D-A)*B+C
      | C+(D-A)*B+C+CARRYIN
      | C+(D-A)*B+CARRYIN
      | C+(D-A)*B+P
      | C+(D-A)*B+P+CARRYIN
      | C+(D-A)*B+P>>17
      | C+(D-A)*B+P>>17+CARRYIN
      | C+(D-A)*B+PCIN
      | C+(D-A)*B+PCIN+CARRYIN
      | C+(D-A)*B+PCIN>>17
      | C+(D-A)*B+PCIN>>17+CARRYIN
      | C+(D-A)*B-C
      | C+(D-A)*B-P
      | C+(D-A)*B-P>>17
      | C+(D-A)*B-PCIN
      | C+(D-A)*B-PCIN>>17
      | C+(D-A)+C
      | C+(D-A)+C+CARRYIN
      | C+(D-A)+CARRYIN
      | C+(D-A)+P
      | C+(D-A)+P+CARRYIN
      | C+(D-A)+P>>17
      | C+(D-A)+P>>17+CARRYIN
      | C+(D-A)+PCIN
      | C+(D-A)+PCIN+CARRYIN
      | C+(D-A)+PCIN>>17
      | C+(D-A)+PCIN>>17+CARRYIN
      | C+(D-A)-C
      | C+(D-A)-P
      | C+(D-A)-P>>17
      | C+(D-A)-PCIN
      | C+(D-A)-PCIN>>17
      | C+A
      | C+A*B
      | C+A*B+C
      | C+A*B+C+CARRYIN
      | C+A*B+CARRYIN
      | C+A*B+P
      | C+A*B+P+CARRYIN
      | C+A*B+P>>17
      | C+A*B+P>>17+CARRYIN
      | C+A*B+PCIN
      | C+A*B+PCIN+CARRYIN
      | C+A*B+PCIN>>17
      | C+A*B+PCIN>>17+CARRYIN
      | C+A*B-C
      | C+A*B-P
      | C+A*B-P>>17
      | C+A*B-PCIN
      | C+A*B-PCIN>>17
      | C+A+C
      | C+A+C+CARRYIN
      | C+A+CARRYIN
      | C+A+P
      | C+A+P+CARRYIN
      | C+A+P>>17
      | C+A+P>>17+CARRYIN
      | C+A+PCIN
      | C+A+PCIN+CARRYIN
      | C+A+PCIN>>17
      | C+A+PCIN>>17+CARRYIN
      | C+A-C
      | C+A-P
      | C+A-P>>17
      | C+A-PCIN
      | C+A-PCIN>>17
      | C+B*(A+D)
      | C+B*(A+D)+C
      | C+B*(A+D)+C+CARRYIN
      | C+B*(A+D)+CARRYIN
      | C+B*(A+D)+P
      | C+B*(A+D)+P+CARRYIN
      | C+B*(A+D)+P>>17
      | C+B*(A+D)+P>>17+CARRYIN
      | C+B*(A+D)+PCIN
      | C+B*(A+D)+PCIN+CARRYIN
      | C+B*(A+D)+PCIN>>17
      | C+B*(A+D)+PCIN>>17+CARRYIN
      | C+B*(A+D)-C
      | C+B*(A+D)-P
      | C+B*(A+D)-P>>17
      | C+B*(A+D)-PCIN
      | C+B*(A+D)-PCIN>>17
      | C+B*(D+A)
      | C+B*(D+A)+C
      | C+B*(D+A)+C+CARRYIN
      | C+B*(D+A)+CARRYIN
      | C+B*(D+A)+P
      | C+B*(D+A)+P+CARRYIN
      | C+B*(D+A)+P>>17
      | C+B*(D+A)+P>>17+CARRYIN
      | C+B*(D+A)+PCIN
      | C+B*(D+A)+PCIN+CARRYIN
      | C+B*(D+A)+PCIN>>17
      | C+B*(D+A)+PCIN>>17+CARRYIN
      | C+B*(D+A)-C
      | C+B*(D+A)-P
      | C+B*(D+A)-P>>17
      | C+B*(D+A)-PCIN
      | C+B*(D+A)-PCIN>>17
      | C+B*(D-A)
      | C+B*(D-A)+C
      | C+B*(D-A)+C+CARRYIN
      | C+B*(D-A)+CARRYIN
      | C+B*(D-A)+P
      | C+B*(D-A)+P+CARRYIN
      | C+B*(D-A)+P>>17
      | C+B*(D-A)+P>>17+CARRYIN
      | C+B*(D-A)+PCIN
      | C+B*(D-A)+PCIN+CARRYIN
      | C+B*(D-A)+PCIN>>17
      | C+B*(D-A)+PCIN>>17+CARRYIN
      | C+B*(D-A)-C
      | C+B*(D-A)-P
      | C+B*(D-A)-P>>17
      | C+B*(D-A)-PCIN
      | C+B*(D-A)-PCIN>>17
      | C+B*A
      | C+B*A+C
      | C+B*A+C+CARRYIN
      | C+B*A+CARRYIN
      | C+B*A+P
      | C+B*A+P+CARRYIN
      | C+B*A+P>>17
      | C+B*A+P>>17+CARRYIN
      | C+B*A+PCIN
      | C+B*A+PCIN+CARRYIN
      | C+B*A+PCIN>>17
      | C+B*A+PCIN>>17+CARRYIN
      | C+B*A-C
      | C+B*A-P
      | C+B*A-P>>17
      | C+B*A-PCIN
      | C+B*A-PCIN>>17
      | C+B*D
      | C+B*D+C
      | C+B*D+C+CARRYIN
      | C+B*D+CARRYIN
      | C+B*D+P
      | C+B*D+P+CARRYIN
      | C+B*D+P>>17
      | C+B*D+P>>17+CARRYIN
      | C+B*D+PCIN
      | C+B*D+PCIN+CARRYIN
      | C+B*D+PCIN>>17
      | C+B*D+PCIN>>17+CARRYIN
      | C+B*D-C
      | C+B*D-P
      | C+B*D-P>>17
      | C+B*D-PCIN
      | C+B*D-PCIN>>17
      | C+C
      | C+C+(A+D)
      | C+C+(A+D)*B
      | C+C+(A+D)*B+CARRYIN
      | C+C+(A+D)+CARRYIN
      | C+C+(D+A)
      | C+C+(D+A)*B
      | C+C+(D+A)*B+CARRYIN
      | C+C+(D+A)+CARRYIN
      | C+C+(D-A)
      | C+C+(D-A)*B
      | C+C+(D-A)*B+CARRYIN
      | C+C+(D-A)+CARRYIN
      | C+C+A
      | C+C+A*B
      | C+C+A*B+CARRYIN
      | C+C+A+CARRYIN
      | C+C+B*(A+D)
      | C+C+B*(A+D)+CARRYIN
      | C+C+B*(D+A)
      | C+C+B*(D+A)+CARRYIN
      | C+C+B*(D-A)
      | C+C+B*(D-A)+CARRYIN
      | C+C+B*A
      | C+C+B*A+CARRYIN
      | C+C+B*D
      | C+C+B*D+CARRYIN
      | C+C+C
      | C+C+C+CARRYIN
      | C+C+C+P
      | C+C+C+P+CARRYIN
      | C+C+CARRYCASCIN
      | C+C+CARRYIN
      | C+C+D
      | C+C+D*B
      | C+C+D*B+CARRYIN
      | C+C+D+CARRYIN
      | C+C+P
      | C+C+P+C
      | C+C+P+C+CARRYIN
      | C+C+P+CARRYIN
      | C+C+P+P
      | C+C+P+P+CARRYIN
      | C+C+P+P>>17
      | C+C+P+P>>17+CARRYIN
      | C+C+P+PCIN
      | C+C+P+PCIN+CARRYIN
      | C+C+P+PCIN>>17
      | C+C+P+PCIN>>17+CARRYIN
      | C+C+P-C
      | C+C+P-P
      | C+C+P-P>>17
      | C+C+P-PCIN
      | C+C+P-PCIN>>17
      | C+C+P>>17
      | C+C+P>>17+CARRYIN
      | C+C+P>>17+P
      | C+C+P>>17+P+CARRYIN
      | C+C+PCIN
      | C+C+PCIN+CARRYIN
      | C+C+PCIN+P
      | C+C+PCIN+P+CARRYIN
      | C+C+PCIN>>17
      | C+C+PCIN>>17+CARRYIN
      | C+C+PCIN>>17+P
      | C+C+PCIN>>17+P+CARRYIN
      | C+C-C
      | C+C-P
      | C+C-P>>17
      | C+C-PCIN
      | C+C-PCIN>>17
      | C+CARRYCASCIN
      | C+CARRYIN
      | C+D
      | C+D*B
      | C+D*B+C
      | C+D*B+C+CARRYIN
      | C+D*B+CARRYIN
      | C+D*B+P
      | C+D*B+P+CARRYIN
      | C+D*B+P>>17
      | C+D*B+P>>17+CARRYIN
      | C+D*B+PCIN
      | C+D*B+PCIN+CARRYIN
      | C+D*B+PCIN>>17
      | C+D*B+PCIN>>17+CARRYIN
      | C+D*B-C
      | C+D*B-P
      | C+D*B-P>>17
      | C+D*B-PCIN
      | C+D*B-PCIN>>17
      | C+D+C
      | C+D+C+CARRYIN
      | C+D+CARRYIN
      | C+D+P
      | C+D+P+CARRYIN
      | C+D+P>>17
      | C+D+P>>17+CARRYIN
      | C+D+PCIN
      | C+D+PCIN+CARRYIN
      | C+D+PCIN>>17
      | C+D+PCIN>>17+CARRYIN
      | C+D-C
      | C+D-P
      | C+D-P>>17
      | C+D-PCIN
      | C+D-PCIN>>17
      | C+P
      | C+P+(A+D)
      | C+P+(A+D)*B
      | C+P+(A+D)*B+CARRYIN
      | C+P+(A+D)+CARRYIN
      | C+P+(D+A)
      | C+P+(D+A)*B
      | C+P+(D+A)*B+CARRYIN
      | C+P+(D+A)+CARRYIN
      | C+P+(D-A)
      | C+P+(D-A)*B
      | C+P+(D-A)*B+CARRYIN
      | C+P+(D-A)+CARRYIN
      | C+P+A
      | C+P+A*B
      | C+P+A*B+CARRYIN
      | C+P+A+CARRYIN
      | C+P+B*(A+D)
      | C+P+B*(A+D)+CARRYIN
      | C+P+B*(D+A)
      | C+P+B*(D+A)+CARRYIN
      | C+P+B*(D-A)
      | C+P+B*(D-A)+CARRYIN
      | C+P+B*A
      | C+P+B*A+CARRYIN
      | C+P+B*D
      | C+P+B*D+CARRYIN
      | C+P+C
      | C+P+C+C
      | C+P+C+C+CARRYIN
      | C+P+C+CARRYIN
      | C+P+C+P
      | C+P+C+P+CARRYIN
      | C+P+C+P>>17
      | C+P+C+P>>17+CARRYIN
      | C+P+C+PCIN
      | C+P+C+PCIN+CARRYIN
      | C+P+C+PCIN>>17
      | C+P+C+PCIN>>17+CARRYIN
      | C+P+C-C
      | C+P+C-P
      | C+P+C-P>>17
      | C+P+C-PCIN
      | C+P+C-PCIN>>17
      | C+P+CARRYCASCIN
      | C+P+CARRYIN
      | C+P+D
      | C+P+D*B
      | C+P+D*B+CARRYIN
      | C+P+D+CARRYIN
      | C+P+P
      | C+P+P+C
      | C+P+P+C+CARRYIN
      | C+P+P+CARRYIN
      | C+P+P+P
      | C+P+P+P+CARRYIN
      | C+P+P+P>>17
      | C+P+P+P>>17+CARRYIN
      | C+P+P+PCIN
      | C+P+P+PCIN+CARRYIN
      | C+P+P+PCIN>>17
      | C+P+P+PCIN>>17+CARRYIN
      | C+P+P-C
      | C+P+P-P
      | C+P+P-P>>17
      | C+P+P-PCIN
      | C+P+P-PCIN>>17
      | C+P+P>>17
      | C+P+P>>17+C
      | C+P+P>>17+C+CARRYIN
      | C+P+P>>17+CARRYIN
      | C+P+P>>17+P
      | C+P+P>>17+P+CARRYIN
      | C+P+PCIN
      | C+P+PCIN+C
      | C+P+PCIN+C+CARRYIN
      | C+P+PCIN+CARRYIN
      | C+P+PCIN+P
      | C+P+PCIN+P+CARRYIN
      | C+P+PCIN>>17
      | C+P+PCIN>>17+C
      | C+P+PCIN>>17+C+CARRYIN
      | C+P+PCIN>>17+CARRYIN
      | C+P+PCIN>>17+P
      | C+P+PCIN>>17+P+CARRYIN
      | C+P-C
      | C+P-P
      | C+P-P>>17
      | C+P-PCIN
      | C+P-PCIN>>17
      | C+P>>17
      | C+P>>17+(A+D)
      | C+P>>17+(A+D)*B
      | C+P>>17+(A+D)*B+CARRYIN
      | C+P>>17+(A+D)+CARRYIN
      | C+P>>17+(D+A)
      | C+P>>17+(D+A)*B
      | C+P>>17+(D+A)*B+CARRYIN
      | C+P>>17+(D+A)+CARRYIN
      | C+P>>17+(D-A)
      | C+P>>17+(D-A)*B
      | C+P>>17+(D-A)*B+CARRYIN
      | C+P>>17+(D-A)+CARRYIN
      | C+P>>17+A
      | C+P>>17+A*B
      | C+P>>17+A*B+CARRYIN
      | C+P>>17+A+CARRYIN
      | C+P>>17+B*(A+D)
      | C+P>>17+B*(A+D)+CARRYIN
      | C+P>>17+B*(D+A)
      | C+P>>17+B*(D+A)+CARRYIN
      | C+P>>17+B*(D-A)
      | C+P>>17+B*(D-A)+CARRYIN
      | C+P>>17+B*A
      | C+P>>17+B*A+CARRYIN
      | C+P>>17+B*D
      | C+P>>17+B*D+CARRYIN
      | C+P>>17+C
      | C+P>>17+C+CARRYIN
      | C+P>>17+C+P
      | C+P>>17+C+P+CARRYIN
      | C+P>>17+CARRYIN
      | C+P>>17+D
      | C+P>>17+D*B
      | C+P>>17+D*B+CARRYIN
      | C+P>>17+D+CARRYIN
      | C+P>>17+P
      | C+P>>17+P+C
      | C+P>>17+P+C+CARRYIN
      | C+P>>17+P+CARRYIN
      | C+P>>17+P+P
      | C+P>>17+P+P+CARRYIN
      | C+PCIN
      | C+PCIN+(A+D)
      | C+PCIN+(A+D)*B
      | C+PCIN+(A+D)*B+CARRYIN
      | C+PCIN+(A+D)+CARRYIN
      | C+PCIN+(D+A)
      | C+PCIN+(D+A)*B
      | C+PCIN+(D+A)*B+CARRYIN
      | C+PCIN+(D+A)+CARRYIN
      | C+PCIN+(D-A)
      | C+PCIN+(D-A)*B
      | C+PCIN+(D-A)*B+CARRYIN
      | C+PCIN+(D-A)+CARRYIN
      | C+PCIN+A
      | C+PCIN+A*B
      | C+PCIN+A*B+CARRYIN
      | C+PCIN+A+CARRYIN
      | C+PCIN+B*(A+D)
      | C+PCIN+B*(A+D)+CARRYIN
      | C+PCIN+B*(D+A)
      | C+PCIN+B*(D+A)+CARRYIN
      | C+PCIN+B*(D-A)
      | C+PCIN+B*(D-A)+CARRYIN
      | C+PCIN+B*A
      | C+PCIN+B*A+CARRYIN
      | C+PCIN+B*D
      | C+PCIN+B*D+CARRYIN
      | C+PCIN+C
      | C+PCIN+C+CARRYIN
      | C+PCIN+C+P
      | C+PCIN+C+P+CARRYIN
      | C+PCIN+CARRYIN
      | C+PCIN+D
      | C+PCIN+D*B
      | C+PCIN+D*B+CARRYIN
      | C+PCIN+D+CARRYIN
      | C+PCIN+P
      | C+PCIN+P+C
      | C+PCIN+P+C+CARRYIN
      | C+PCIN+P+CARRYIN
      | C+PCIN+P+P
      | C+PCIN+P+P+CARRYIN
      | C+PCIN>>17
      | C+PCIN>>17+(A+D)
      | C+PCIN>>17+(A+D)*B
      | C+PCIN>>17+(A+D)*B+CARRYIN
      | C+PCIN>>17+(A+D)+CARRYIN
      | C+PCIN>>17+(D+A)
      | C+PCIN>>17+(D+A)*B
      | C+PCIN>>17+(D+A)*B+CARRYIN
      | C+PCIN>>17+(D+A)+CARRYIN
      | C+PCIN>>17+(D-A)
      | C+PCIN>>17+(D-A)*B
      | C+PCIN>>17+(D-A)*B+CARRYIN
      | C+PCIN>>17+(D-A)+CARRYIN
      | C+PCIN>>17+A
      | C+PCIN>>17+A*B
      | C+PCIN>>17+A*B+CARRYIN
      | C+PCIN>>17+A+CARRYIN
      | C+PCIN>>17+B*(A+D)
      | C+PCIN>>17+B*(A+D)+CARRYIN
      | C+PCIN>>17+B*(D+A)
      | C+PCIN>>17+B*(D+A)+CARRYIN
      | C+PCIN>>17+B*(D-A)
      | C+PCIN>>17+B*(D-A)+CARRYIN
      | C+PCIN>>17+B*A
      | C+PCIN>>17+B*A+CARRYIN
      | C+PCIN>>17+B*D
      | C+PCIN>>17+B*D+CARRYIN
      | C+PCIN>>17+C
      | C+PCIN>>17+C+CARRYIN
      | C+PCIN>>17+C+P
      | C+PCIN>>17+C+P+CARRYIN
      | C+PCIN>>17+CARRYIN
      | C+PCIN>>17+D
      | C+PCIN>>17+D*B
      | C+PCIN>>17+D*B+CARRYIN
      | C+PCIN>>17+D+CARRYIN
      | C+PCIN>>17+P
      | C+PCIN>>17+P+C
      | C+PCIN>>17+P+C+CARRYIN
      | C+PCIN>>17+P+CARRYIN
      | C+PCIN>>17+P+P
      | C+PCIN>>17+P+P+CARRYIN
      | C-((A+D))
      | C-((A+D)*B)
      | C-((A+D)*B+C)
      | C-((A+D)*B+C+CARRYIN)
      | C-((A+D)*B+CARRYIN)
      | C-((A+D)*B+P)
      | C-((A+D)*B+P+CARRYIN)
      | C-((A+D)+C)
      | C-((A+D)+C+CARRYIN)
      | C-((A+D)+CARRYIN)
      | C-((A+D)+P)
      | C-((A+D)+P+CARRYIN)
      | C-((D+A))
      | C-((D+A)*B)
      | C-((D+A)*B+C)
      | C-((D+A)*B+C+CARRYIN)
      | C-((D+A)*B+CARRYIN)
      | C-((D+A)*B+P)
      | C-((D+A)*B+P+CARRYIN)
      | C-((D+A)+C)
      | C-((D+A)+C+CARRYIN)
      | C-((D+A)+CARRYIN)
      | C-((D+A)+P)
      | C-((D+A)+P+CARRYIN)
      | C-((D-A))
      | C-((D-A)*B)
      | C-((D-A)*B+C)
      | C-((D-A)*B+C+CARRYIN)
      | C-((D-A)*B+CARRYIN)
      | C-((D-A)*B+P)
      | C-((D-A)*B+P+CARRYIN)
      | C-((D-A)+C)
      | C-((D-A)+C+CARRYIN)
      | C-((D-A)+CARRYIN)
      | C-((D-A)+P)
      | C-((D-A)+P+CARRYIN)
      | C-(A)
      | C-(A*B)
      | C-(A*B+C)
      | C-(A*B+C+CARRYIN)
      | C-(A*B+CARRYIN)
      | C-(A*B+P)
      | C-(A*B+P+CARRYIN)
      | C-(A+C)
      | C-(A+C+CARRYIN)
      | C-(A+CARRYIN)
      | C-(A+D)
      | C-(A+D)*B
      | C-(A+D)*B-C
      | C-(A+D)*B-C-CARRYIN
      | C-(A+D)*B-CARRYIN
      | C-(A+D)*B-P
      | C-(A+D)*B-P-CARRYIN
      | C-(A+D)-C
      | C-(A+D)-C-CARRYIN
      | C-(A+D)-CARRYIN
      | C-(A+D)-P
      | C-(A+D)-P-CARRYIN
      | C-(A+P)
      | C-(A+P+CARRYIN)
      | C-(B*(A+D))
      | C-(B*(A+D)+C)
      | C-(B*(A+D)+C+CARRYIN)
      | C-(B*(A+D)+CARRYIN)
      | C-(B*(A+D)+P)
      | C-(B*(A+D)+P+CARRYIN)
      | C-(B*(D+A))
      | C-(B*(D+A)+C)
      | C-(B*(D+A)+C+CARRYIN)
      | C-(B*(D+A)+CARRYIN)
      | C-(B*(D+A)+P)
      | C-(B*(D+A)+P+CARRYIN)
      | C-(B*(D-A))
      | C-(B*(D-A)+C)
      | C-(B*(D-A)+C+CARRYIN)
      | C-(B*(D-A)+CARRYIN)
      | C-(B*(D-A)+P)
      | C-(B*(D-A)+P+CARRYIN)
      | C-(B*A)
      | C-(B*A+C)
      | C-(B*A+C+CARRYIN)
      | C-(B*A+CARRYIN)
      | C-(B*A+P)
      | C-(B*A+P+CARRYIN)
      | C-(B*D)
      | C-(B*D+C)
      | C-(B*D+C+CARRYIN)
      | C-(B*D+CARRYIN)
      | C-(B*D+P)
      | C-(B*D+P+CARRYIN)
      | C-(C)
      | C-(C+(A+D))
      | C-(C+(A+D)*B)
      | C-(C+(A+D)*B+CARRYIN)
      | C-(C+(A+D)+CARRYIN)
      | C-(C+(D+A))
      | C-(C+(D+A)*B)
      | C-(C+(D+A)*B+CARRYIN)
      | C-(C+(D+A)+CARRYIN)
      | C-(C+(D-A))
      | C-(C+(D-A)*B)
      | C-(C+(D-A)*B+CARRYIN)
      | C-(C+(D-A)+CARRYIN)
      | C-(C+A)
      | C-(C+A*B)
      | C-(C+A*B+CARRYIN)
      | C-(C+A+CARRYIN)
      | C-(C+B*(A+D))
      | C-(C+B*(A+D)+CARRYIN)
      | C-(C+B*(D+A))
      | C-(C+B*(D+A)+CARRYIN)
      | C-(C+B*(D-A))
      | C-(C+B*(D-A)+CARRYIN)
      | C-(C+B*A)
      | C-(C+B*A+CARRYIN)
      | C-(C+B*D)
      | C-(C+B*D+CARRYIN)
      | C-(C+C)
      | C-(C+C+CARRYIN)
      | C-(C+C+P)
      | C-(C+C+P+CARRYIN)
      | C-(C+CARRYCASCIN)
      | C-(C+CARRYIN)
      | C-(C+D)
      | C-(C+D*B)
      | C-(C+D*B+CARRYIN)
      | C-(C+D+CARRYIN)
      | C-(C+P)
      | C-(C+P+C)
      | C-(C+P+C+CARRYIN)
      | C-(C+P+CARRYIN)
      | C-(C+P+P)
      | C-(C+P+P+CARRYIN)
      | C-(CARRYCASCIN)
      | C-(CARRYIN)
      | C-(D)
      | C-(D*B)
      | C-(D*B+C)
      | C-(D*B+C+CARRYIN)
      | C-(D*B+CARRYIN)
      | C-(D*B+P)
      | C-(D*B+P+CARRYIN)
      | C-(D+A)
      | C-(D+A)*B
      | C-(D+A)*B-C
      | C-(D+A)*B-C-CARRYIN
      | C-(D+A)*B-CARRYIN
      | C-(D+A)*B-P
      | C-(D+A)*B-P-CARRYIN
      | C-(D+A)-C
      | C-(D+A)-C-CARRYIN
      | C-(D+A)-CARRYIN
      | C-(D+A)-P
      | C-(D+A)-P-CARRYIN
      | C-(D+C)
      | C-(D+C+CARRYIN)
      | C-(D+CARRYIN)
      | C-(D+P)
      | C-(D+P+CARRYIN)
      | C-(D-A)
      | C-(D-A)*B
      | C-(D-A)*B-C
      | C-(D-A)*B-C-CARRYIN
      | C-(D-A)*B-CARRYIN
      | C-(D-A)*B-P
      | C-(D-A)*B-P-CARRYIN
      | C-(D-A)-C
      | C-(D-A)-C-CARRYIN
      | C-(D-A)-CARRYIN
      | C-(D-A)-P
      | C-(D-A)-P-CARRYIN
      | C-(P)
      | C-(P+(A+D))
      | C-(P+(A+D)*B)
      | C-(P+(A+D)*B+CARRYIN)
      | C-(P+(A+D)+CARRYIN)
      | C-(P+(D+A))
      | C-(P+(D+A)*B)
      | C-(P+(D+A)*B+CARRYIN)
      | C-(P+(D+A)+CARRYIN)
      | C-(P+(D-A))
      | C-(P+(D-A)*B)
      | C-(P+(D-A)*B+CARRYIN)
      | C-(P+(D-A)+CARRYIN)
      | C-(P+A)
      | C-(P+A*B)
      | C-(P+A*B+CARRYIN)
      | C-(P+A+CARRYIN)
      | C-(P+B*(A+D))
      | C-(P+B*(A+D)+CARRYIN)
      | C-(P+B*(D+A))
      | C-(P+B*(D+A)+CARRYIN)
      | C-(P+B*(D-A))
      | C-(P+B*(D-A)+CARRYIN)
      | C-(P+B*A)
      | C-(P+B*A+CARRYIN)
      | C-(P+B*D)
      | C-(P+B*D+CARRYIN)
      | C-(P+C)
      | C-(P+C+C)
      | C-(P+C+C+CARRYIN)
      | C-(P+C+CARRYIN)
      | C-(P+C+P)
      | C-(P+C+P+CARRYIN)
      | C-(P+CARRYCASCIN)
      | C-(P+CARRYIN)
      | C-(P+D)
      | C-(P+D*B)
      | C-(P+D*B+CARRYIN)
      | C-(P+D+CARRYIN)
      | C-(P+P)
      | C-(P+P+C)
      | C-(P+P+C+CARRYIN)
      | C-(P+P+CARRYIN)
      | C-A
      | C-A*B
      | C-A*B-C
      | C-A*B-C-CARRYIN
      | C-A*B-CARRYIN
      | C-A*B-P
      | C-A*B-P-CARRYIN
      | C-A-C
      | C-A-C-CARRYIN
      | C-A-CARRYIN
      | C-A-P
      | C-A-P-CARRYIN
      | C-B*(A+D)
      | C-B*(A+D)-C
      | C-B*(A+D)-C-CARRYIN
      | C-B*(A+D)-CARRYIN
      | C-B*(A+D)-P
      | C-B*(A+D)-P-CARRYIN
      | C-B*(D+A)
      | C-B*(D+A)-C
      | C-B*(D+A)-C-CARRYIN
      | C-B*(D+A)-CARRYIN
      | C-B*(D+A)-P
      | C-B*(D+A)-P-CARRYIN
      | C-B*(D-A)
      | C-B*(D-A)-C
      | C-B*(D-A)-C-CARRYIN
      | C-B*(D-A)-CARRYIN
      | C-B*(D-A)-P
      | C-B*(D-A)-P-CARRYIN
      | C-B*A
      | C-B*A-C
      | C-B*A-C-CARRYIN
      | C-B*A-CARRYIN
      | C-B*A-P
      | C-B*A-P-CARRYIN
      | C-B*D
      | C-B*D-C
      | C-B*D-C-CARRYIN
      | C-B*D-CARRYIN
      | C-B*D-P
      | C-B*D-P-CARRYIN
      | C-C
      | C-C-(A+D)
      | C-C-(A+D)*B
      | C-C-(A+D)*B-CARRYIN
      | C-C-(A+D)-CARRYIN
      | C-C-(D+A)
      | C-C-(D+A)*B
      | C-C-(D+A)*B-CARRYIN
      | C-C-(D+A)-CARRYIN
      | C-C-(D-A)
      | C-C-(D-A)*B
      | C-C-(D-A)*B-CARRYIN
      | C-C-(D-A)-CARRYIN
      | C-C-A
      | C-C-A*B
      | C-C-A*B-CARRYIN
      | C-C-A-CARRYIN
      | C-C-B*(A+D)
      | C-C-B*(A+D)-CARRYIN
      | C-C-B*(D+A)
      | C-C-B*(D+A)-CARRYIN
      | C-C-B*(D-A)
      | C-C-B*(D-A)-CARRYIN
      | C-C-B*A
      | C-C-B*A-CARRYIN
      | C-C-B*D
      | C-C-B*D-CARRYIN
      | C-C-C
      | C-C-C-CARRYIN
      | C-C-C-P
      | C-C-C-P-CARRYIN
      | C-C-CARRYCASCIN
      | C-C-CARRYIN
      | C-C-D
      | C-C-D*B
      | C-C-D*B-CARRYIN
      | C-C-D-CARRYIN
      | C-C-P
      | C-C-P-C
      | C-C-P-C-CARRYIN
      | C-C-P-CARRYIN
      | C-C-P-P
      | C-C-P-P-CARRYIN
      | C-CARRYCASCIN
      | C-CARRYIN
      | C-D
      | C-D*B
      | C-D*B-C
      | C-D*B-C-CARRYIN
      | C-D*B-CARRYIN
      | C-D*B-P
      | C-D*B-P-CARRYIN
      | C-D-C
      | C-D-C-CARRYIN
      | C-D-CARRYIN
      | C-D-P
      | C-D-P-CARRYIN
      | C-P
      | C-P-(A+D)
      | C-P-(A+D)*B
      | C-P-(A+D)*B-CARRYIN
      | C-P-(A+D)-CARRYIN
      | C-P-(D+A)
      | C-P-(D+A)*B
      | C-P-(D+A)*B-CARRYIN
      | C-P-(D+A)-CARRYIN
      | C-P-(D-A)
      | C-P-(D-A)*B
      | C-P-(D-A)*B-CARRYIN
      | C-P-(D-A)-CARRYIN
      | C-P-A
      | C-P-A*B
      | C-P-A*B-CARRYIN
      | C-P-A-CARRYIN
      | C-P-B*(A+D)
      | C-P-B*(A+D)-CARRYIN
      | C-P-B*(D+A)
      | C-P-B*(D+A)-CARRYIN
      | C-P-B*(D-A)
      | C-P-B*(D-A)-CARRYIN
      | C-P-B*A
      | C-P-B*A-CARRYIN
      | C-P-B*D
      | C-P-B*D-CARRYIN
      | C-P-C
      | C-P-C-C
      | C-P-C-C-CARRYIN
      | C-P-C-CARRYIN
      | C-P-C-P
      | C-P-C-P-CARRYIN
      | C-P-CARRYCASCIN
      | C-P-CARRYIN
      | C-P-D
      | C-P-D*B
      | C-P-D*B-CARRYIN
      | C-P-D-CARRYIN
      | C-P-P
      | C-P-P-C
      | C-P-P-C-CARRYIN
      | C-P-P-CARRYIN
      | C-P>>17
      | C-PCIN
      | C-PCIN>>17
      | CARRYIN
      | D
      | D*B
      | D*B+C
      | D*B+C+C
      | D*B+C+C+CARRYIN
      | D*B+C+CARRYIN
      | D*B+C+P
      | D*B+C+P+CARRYIN
      | D*B+C+P>>17
      | D*B+C+P>>17+CARRYIN
      | D*B+C+PCIN
      | D*B+C+PCIN+CARRYIN
      | D*B+C+PCIN>>17
      | D*B+C+PCIN>>17+CARRYIN
      | D*B+C-C
      | D*B+C-P
      | D*B+C-P>>17
      | D*B+C-PCIN
      | D*B+C-PCIN>>17
      | D*B+CARRYIN
      | D*B+P
      | D*B+P+C
      | D*B+P+C+CARRYIN
      | D*B+P+CARRYIN
      | D*B+P+P
      | D*B+P+P+CARRYIN
      | D*B+P+P>>17
      | D*B+P+P>>17+CARRYIN
      | D*B+P+PCIN
      | D*B+P+PCIN+CARRYIN
      | D*B+P+PCIN>>17
      | D*B+P+PCIN>>17+CARRYIN
      | D*B+P-C
      | D*B+P-P
      | D*B+P-P>>17
      | D*B+P-PCIN
      | D*B+P-PCIN>>17
      | D*B+P>>17
      | D*B+P>>17+C
      | D*B+P>>17+C+CARRYIN
      | D*B+P>>17+CARRYIN
      | D*B+P>>17+P
      | D*B+P>>17+P+CARRYIN
      | D*B+PCIN
      | D*B+PCIN+C
      | D*B+PCIN+C+CARRYIN
      | D*B+PCIN+CARRYIN
      | D*B+PCIN+P
      | D*B+PCIN+P+CARRYIN
      | D*B+PCIN>>17
      | D*B+PCIN>>17+C
      | D*B+PCIN>>17+C+CARRYIN
      | D*B+PCIN>>17+CARRYIN
      | D*B+PCIN>>17+P
      | D*B+PCIN>>17+P+CARRYIN
      | D*B-C
      | D*B-P
      | D*B-P>>17
      | D*B-PCIN
      | D*B-PCIN>>17
      | D+C
      | D+C+C
      | D+C+C+CARRYIN
      | D+C+CARRYIN
      | D+C+P
      | D+C+P+CARRYIN
      | D+C+P>>17
      | D+C+P>>17+CARRYIN
      | D+C+PCIN
      | D+C+PCIN+CARRYIN
      | D+C+PCIN>>17
      | D+C+PCIN>>17+CARRYIN
      | D+C-C
      | D+C-P
      | D+C-P>>17
      | D+C-PCIN
      | D+C-PCIN>>17
      | D+CARRYIN
      | D+P
      | D+P+C
      | D+P+C+CARRYIN
      | D+P+CARRYIN
      | D+P+P
      | D+P+P+CARRYIN
      | D+P+P>>17
      | D+P+P>>17+CARRYIN
      | D+P+PCIN
      | D+P+PCIN+CARRYIN
      | D+P+PCIN>>17
      | D+P+PCIN>>17+CARRYIN
      | D+P-C
      | D+P-P
      | D+P-P>>17
      | D+P-PCIN
      | D+P-PCIN>>17
      | D+P>>17
      | D+P>>17+C
      | D+P>>17+C+CARRYIN
      | D+P>>17+CARRYIN
      | D+P>>17+P
      | D+P>>17+P+CARRYIN
      | D+PCIN
      | D+PCIN+C
      | D+PCIN+C+CARRYIN
      | D+PCIN+CARRYIN
      | D+PCIN+P
      | D+PCIN+P+CARRYIN
      | D+PCIN>>17
      | D+PCIN>>17+C
      | D+PCIN>>17+C+CARRYIN
      | D+PCIN>>17+CARRYIN
      | D+PCIN>>17+P
      | D+PCIN>>17+P+CARRYIN
      | D-C
      | D-P
      | D-P>>17
      | D-PCIN
      | D-PCIN>>17
      | P
      | P+(A+D)
      | P+(A+D)*B
      | P+(A+D)*B+C
      | P+(A+D)*B+C+CARRYIN
      | P+(A+D)*B+CARRYIN
      | P+(A+D)*B+P
      | P+(A+D)*B+P+CARRYIN
      | P+(A+D)*B+P>>17
      | P+(A+D)*B+P>>17+CARRYIN
      | P+(A+D)*B+PCIN
      | P+(A+D)*B+PCIN+CARRYIN
      | P+(A+D)*B+PCIN>>17
      | P+(A+D)*B+PCIN>>17+CARRYIN
      | P+(A+D)*B-C
      | P+(A+D)*B-P
      | P+(A+D)*B-P>>17
      | P+(A+D)*B-PCIN
      | P+(A+D)*B-PCIN>>17
      | P+(A+D)+C
      | P+(A+D)+C+CARRYIN
      | P+(A+D)+CARRYIN
      | P+(A+D)+P
      | P+(A+D)+P+CARRYIN
      | P+(A+D)+P>>17
      | P+(A+D)+P>>17+CARRYIN
      | P+(A+D)+PCIN
      | P+(A+D)+PCIN+CARRYIN
      | P+(A+D)+PCIN>>17
      | P+(A+D)+PCIN>>17+CARRYIN
      | P+(A+D)-C
      | P+(A+D)-P
      | P+(A+D)-P>>17
      | P+(A+D)-PCIN
      | P+(A+D)-PCIN>>17
      | P+(D+A)
      | P+(D+A)*B
      | P+(D+A)*B+C
      | P+(D+A)*B+C+CARRYIN
      | P+(D+A)*B+CARRYIN
      | P+(D+A)*B+P
      | P+(D+A)*B+P+CARRYIN
      | P+(D+A)*B+P>>17
      | P+(D+A)*B+P>>17+CARRYIN
      | P+(D+A)*B+PCIN
      | P+(D+A)*B+PCIN+CARRYIN
      | P+(D+A)*B+PCIN>>17
      | P+(D+A)*B+PCIN>>17+CARRYIN
      | P+(D+A)*B-C
      | P+(D+A)*B-P
      | P+(D+A)*B-P>>17
      | P+(D+A)*B-PCIN
      | P+(D+A)*B-PCIN>>17
      | P+(D+A)+C
      | P+(D+A)+C+CARRYIN
      | P+(D+A)+CARRYIN
      | P+(D+A)+P
      | P+(D+A)+P+CARRYIN
      | P+(D+A)+P>>17
      | P+(D+A)+P>>17+CARRYIN
      | P+(D+A)+PCIN
      | P+(D+A)+PCIN+CARRYIN
      | P+(D+A)+PCIN>>17
      | P+(D+A)+PCIN>>17+CARRYIN
      | P+(D+A)-C
      | P+(D+A)-P
      | P+(D+A)-P>>17
      | P+(D+A)-PCIN
      | P+(D+A)-PCIN>>17
      | P+(D-A)
      | P+(D-A)*B
      | P+(D-A)*B+C
      | P+(D-A)*B+C+CARRYIN
      | P+(D-A)*B+CARRYIN
      | P+(D-A)*B+P
      | P+(D-A)*B+P+CARRYIN
      | P+(D-A)*B+P>>17
      | P+(D-A)*B+P>>17+CARRYIN
      | P+(D-A)*B+PCIN
      | P+(D-A)*B+PCIN+CARRYIN
      | P+(D-A)*B+PCIN>>17
      | P+(D-A)*B+PCIN>>17+CARRYIN
      | P+(D-A)*B-C
      | P+(D-A)*B-P
      | P+(D-A)*B-P>>17
      | P+(D-A)*B-PCIN
      | P+(D-A)*B-PCIN>>17
      | P+(D-A)+C
      | P+(D-A)+C+CARRYIN
      | P+(D-A)+CARRYIN
      | P+(D-A)+P
      | P+(D-A)+P+CARRYIN
      | P+(D-A)+P>>17
      | P+(D-A)+P>>17+CARRYIN
      | P+(D-A)+PCIN
      | P+(D-A)+PCIN+CARRYIN
      | P+(D-A)+PCIN>>17
      | P+(D-A)+PCIN>>17+CARRYIN
      | P+(D-A)-C
      | P+(D-A)-P
      | P+(D-A)-P>>17
      | P+(D-A)-PCIN
      | P+(D-A)-PCIN>>17
      | P+A
      | P+A*B
      | P+A*B+C
      | P+A*B+C+CARRYIN
      | P+A*B+CARRYIN
      | P+A*B+P
      | P+A*B+P+CARRYIN
      | P+A*B+P>>17
      | P+A*B+P>>17+CARRYIN
      | P+A*B+PCIN
      | P+A*B+PCIN+CARRYIN
      | P+A*B+PCIN>>17
      | P+A*B+PCIN>>17+CARRYIN
      | P+A*B-C
      | P+A*B-P
      | P+A*B-P>>17
      | P+A*B-PCIN
      | P+A*B-PCIN>>17
      | P+A+C
      | P+A+C+CARRYIN
      | P+A+CARRYIN
      | P+A+P
      | P+A+P+CARRYIN
      | P+A+P>>17
      | P+A+P>>17+CARRYIN
      | P+A+PCIN
      | P+A+PCIN+CARRYIN
      | P+A+PCIN>>17
      | P+A+PCIN>>17+CARRYIN
      | P+A-C
      | P+A-P
      | P+A-P>>17
      | P+A-PCIN
      | P+A-PCIN>>17
      | P+B*(A+D)
      | P+B*(A+D)+C
      | P+B*(A+D)+C+CARRYIN
      | P+B*(A+D)+CARRYIN
      | P+B*(A+D)+P
      | P+B*(A+D)+P+CARRYIN
      | P+B*(A+D)+P>>17
      | P+B*(A+D)+P>>17+CARRYIN
      | P+B*(A+D)+PCIN
      | P+B*(A+D)+PCIN+CARRYIN
      | P+B*(A+D)+PCIN>>17
      | P+B*(A+D)+PCIN>>17+CARRYIN
      | P+B*(A+D)-C
      | P+B*(A+D)-P
      | P+B*(A+D)-P>>17
      | P+B*(A+D)-PCIN
      | P+B*(A+D)-PCIN>>17
      | P+B*(D+A)
      | P+B*(D+A)+C
      | P+B*(D+A)+C+CARRYIN
      | P+B*(D+A)+CARRYIN
      | P+B*(D+A)+P
      | P+B*(D+A)+P+CARRYIN
      | P+B*(D+A)+P>>17
      | P+B*(D+A)+P>>17+CARRYIN
      | P+B*(D+A)+PCIN
      | P+B*(D+A)+PCIN+CARRYIN
      | P+B*(D+A)+PCIN>>17
      | P+B*(D+A)+PCIN>>17+CARRYIN
      | P+B*(D+A)-C
      | P+B*(D+A)-P
      | P+B*(D+A)-P>>17
      | P+B*(D+A)-PCIN
      | P+B*(D+A)-PCIN>>17
      | P+B*(D-A)
      | P+B*(D-A)+C
      | P+B*(D-A)+C+CARRYIN
      | P+B*(D-A)+CARRYIN
      | P+B*(D-A)+P
      | P+B*(D-A)+P+CARRYIN
      | P+B*(D-A)+P>>17
      | P+B*(D-A)+P>>17+CARRYIN
      | P+B*(D-A)+PCIN
      | P+B*(D-A)+PCIN+CARRYIN
      | P+B*(D-A)+PCIN>>17
      | P+B*(D-A)+PCIN>>17+CARRYIN
      | P+B*(D-A)-C
      | P+B*(D-A)-P
      | P+B*(D-A)-P>>17
      | P+B*(D-A)-PCIN
      | P+B*(D-A)-PCIN>>17
      | P+B*A
      | P+B*A+C
      | P+B*A+C+CARRYIN
      | P+B*A+CARRYIN
      | P+B*A+P
      | P+B*A+P+CARRYIN
      | P+B*A+P>>17
      | P+B*A+P>>17+CARRYIN
      | P+B*A+PCIN
      | P+B*A+PCIN+CARRYIN
      | P+B*A+PCIN>>17
      | P+B*A+PCIN>>17+CARRYIN
      | P+B*A-C
      | P+B*A-P
      | P+B*A-P>>17
      | P+B*A-PCIN
      | P+B*A-PCIN>>17
      | P+B*D
      | P+B*D+C
      | P+B*D+C+CARRYIN
      | P+B*D+CARRYIN
      | P+B*D+P
      | P+B*D+P+CARRYIN
      | P+B*D+P>>17
      | P+B*D+P>>17+CARRYIN
      | P+B*D+PCIN
      | P+B*D+PCIN+CARRYIN
      | P+B*D+PCIN>>17
      | P+B*D+PCIN>>17+CARRYIN
      | P+B*D-C
      | P+B*D-P
      | P+B*D-P>>17
      | P+B*D-PCIN
      | P+B*D-PCIN>>17
      | P+C
      | P+C+(A+D)
      | P+C+(A+D)*B
      | P+C+(A+D)*B+CARRYIN
      | P+C+(A+D)+CARRYIN
      | P+C+(D+A)
      | P+C+(D+A)*B
      | P+C+(D+A)*B+CARRYIN
      | P+C+(D+A)+CARRYIN
      | P+C+(D-A)
      | P+C+(D-A)*B
      | P+C+(D-A)*B+CARRYIN
      | P+C+(D-A)+CARRYIN
      | P+C+A
      | P+C+A*B
      | P+C+A*B+CARRYIN
      | P+C+A+CARRYIN
      | P+C+B*(A+D)
      | P+C+B*(A+D)+CARRYIN
      | P+C+B*(D+A)
      | P+C+B*(D+A)+CARRYIN
      | P+C+B*(D-A)
      | P+C+B*(D-A)+CARRYIN
      | P+C+B*A
      | P+C+B*A+CARRYIN
      | P+C+B*D
      | P+C+B*D+CARRYIN
      | P+C+C
      | P+C+C+C
      | P+C+C+C+CARRYIN
      | P+C+C+CARRYIN
      | P+C+C+P
      | P+C+C+P+CARRYIN
      | P+C+C+P>>17
      | P+C+C+P>>17+CARRYIN
      | P+C+C+PCIN
      | P+C+C+PCIN+CARRYIN
      | P+C+C+PCIN>>17
      | P+C+C+PCIN>>17+CARRYIN
      | P+C+C-C
      | P+C+C-P
      | P+C+C-P>>17
      | P+C+C-PCIN
      | P+C+C-PCIN>>17
      | P+C+CARRYCASCIN
      | P+C+CARRYIN
      | P+C+D
      | P+C+D*B
      | P+C+D*B+CARRYIN
      | P+C+D+CARRYIN
      | P+C+P
      | P+C+P+C
      | P+C+P+C+CARRYIN
      | P+C+P+CARRYIN
      | P+C+P+P
      | P+C+P+P+CARRYIN
      | P+C+P+P>>17
      | P+C+P+P>>17+CARRYIN
      | P+C+P+PCIN
      | P+C+P+PCIN+CARRYIN
      | P+C+P+PCIN>>17
      | P+C+P+PCIN>>17+CARRYIN
      | P+C+P-C
      | P+C+P-P
      | P+C+P-P>>17
      | P+C+P-PCIN
      | P+C+P-PCIN>>17
      | P+C+P>>17
      | P+C+P>>17+C
      | P+C+P>>17+C+CARRYIN
      | P+C+P>>17+CARRYIN
      | P+C+P>>17+P
      | P+C+P>>17+P+CARRYIN
      | P+C+PCIN
      | P+C+PCIN+C
      | P+C+PCIN+C+CARRYIN
      | P+C+PCIN+CARRYIN
      | P+C+PCIN+P
      | P+C+PCIN+P+CARRYIN
      | P+C+PCIN>>17
      | P+C+PCIN>>17+C
      | P+C+PCIN>>17+C+CARRYIN
      | P+C+PCIN>>17+CARRYIN
      | P+C+PCIN>>17+P
      | P+C+PCIN>>17+P+CARRYIN
      | P+C-C
      | P+C-P
      | P+C-P>>17
      | P+C-PCIN
      | P+C-PCIN>>17
      | P+CARRYCASCIN
      | P+CARRYIN
      | P+D
      | P+D*B
      | P+D*B+C
      | P+D*B+C+CARRYIN
      | P+D*B+CARRYIN
      | P+D*B+P
      | P+D*B+P+CARRYIN
      | P+D*B+P>>17
      | P+D*B+P>>17+CARRYIN
      | P+D*B+PCIN
      | P+D*B+PCIN+CARRYIN
      | P+D*B+PCIN>>17
      | P+D*B+PCIN>>17+CARRYIN
      | P+D*B-C
      | P+D*B-P
      | P+D*B-P>>17
      | P+D*B-PCIN
      | P+D*B-PCIN>>17
      | P+D+C
      | P+D+C+CARRYIN
      | P+D+CARRYIN
      | P+D+P
      | P+D+P+CARRYIN
      | P+D+P>>17
      | P+D+P>>17+CARRYIN
      | P+D+PCIN
      | P+D+PCIN+CARRYIN
      | P+D+PCIN>>17
      | P+D+PCIN>>17+CARRYIN
      | P+D-C
      | P+D-P
      | P+D-P>>17
      | P+D-PCIN
      | P+D-PCIN>>17
      | P+P
      | P+P+(A+D)
      | P+P+(A+D)*B
      | P+P+(A+D)*B+CARRYIN
      | P+P+(A+D)+CARRYIN
      | P+P+(D+A)
      | P+P+(D+A)*B
      | P+P+(D+A)*B+CARRYIN
      | P+P+(D+A)+CARRYIN
      | P+P+(D-A)
      | P+P+(D-A)*B
      | P+P+(D-A)*B+CARRYIN
      | P+P+(D-A)+CARRYIN
      | P+P+A
      | P+P+A*B
      | P+P+A*B+CARRYIN
      | P+P+A+CARRYIN
      | P+P+B*(A+D)
      | P+P+B*(A+D)+CARRYIN
      | P+P+B*(D+A)
      | P+P+B*(D+A)+CARRYIN
      | P+P+B*(D-A)
      | P+P+B*(D-A)+CARRYIN
      | P+P+B*A
      | P+P+B*A+CARRYIN
      | P+P+B*D
      | P+P+B*D+CARRYIN
      | P+P+C
      | P+P+C+C
      | P+P+C+C+CARRYIN
      | P+P+C+CARRYIN
      | P+P+C+P
      | P+P+C+P+CARRYIN
      | P+P+C+P>>17
      | P+P+C+P>>17+CARRYIN
      | P+P+C+PCIN
      | P+P+C+PCIN+CARRYIN
      | P+P+C+PCIN>>17
      | P+P+C+PCIN>>17+CARRYIN
      | P+P+C-C
      | P+P+C-P
      | P+P+C-P>>17
      | P+P+C-PCIN
      | P+P+C-PCIN>>17
      | P+P+CARRYCASCIN
      | P+P+CARRYIN
      | P+P+D
      | P+P+D*B
      | P+P+D*B+CARRYIN
      | P+P+D+CARRYIN
      | P+P+P
      | P+P+P+C
      | P+P+P+C+CARRYIN
      | P+P+P+CARRYIN
      | P+P+P>>17
      | P+P+P>>17+C
      | P+P+P>>17+C+CARRYIN
      | P+P+P>>17+CARRYIN
      | P+P+PCIN
      | P+P+PCIN+C
      | P+P+PCIN+C+CARRYIN
      | P+P+PCIN+CARRYIN
      | P+P+PCIN>>17
      | P+P+PCIN>>17+C
      | P+P+PCIN>>17+C+CARRYIN
      | P+P+PCIN>>17+CARRYIN
      | P+P-C
      | P+P-P
      | P+P-P>>17
      | P+P-PCIN
      | P+P-PCIN>>17
      | P+P>>17
      | P+P>>17+(A+D)
      | P+P>>17+(A+D)*B
      | P+P>>17+(A+D)*B+CARRYIN
      | P+P>>17+(A+D)+CARRYIN
      | P+P>>17+(D+A)
      | P+P>>17+(D+A)*B
      | P+P>>17+(D+A)*B+CARRYIN
      | P+P>>17+(D+A)+CARRYIN
      | P+P>>17+(D-A)
      | P+P>>17+(D-A)*B
      | P+P>>17+(D-A)*B+CARRYIN
      | P+P>>17+(D-A)+CARRYIN
      | P+P>>17+A
      | P+P>>17+A*B
      | P+P>>17+A*B+CARRYIN
      | P+P>>17+A+CARRYIN
      | P+P>>17+B*(A+D)
      | P+P>>17+B*(A+D)+CARRYIN
      | P+P>>17+B*(D+A)
      | P+P>>17+B*(D+A)+CARRYIN
      | P+P>>17+B*(D-A)
      | P+P>>17+B*(D-A)+CARRYIN
      | P+P>>17+B*A
      | P+P>>17+B*A+CARRYIN
      | P+P>>17+B*D
      | P+P>>17+B*D+CARRYIN
      | P+P>>17+C
      | P+P>>17+C+C
      | P+P>>17+C+C+CARRYIN
      | P+P>>17+C+CARRYIN
      | P+P>>17+C+P
      | P+P>>17+C+P+CARRYIN
      | P+P>>17+CARRYIN
      | P+P>>17+D
      | P+P>>17+D*B
      | P+P>>17+D*B+CARRYIN
      | P+P>>17+D+CARRYIN
      | P+P>>17+P
      | P+P>>17+P+C
      | P+P>>17+P+C+CARRYIN
      | P+P>>17+P+CARRYIN
      | P+PCIN
      | P+PCIN+(A+D)
      | P+PCIN+(A+D)*B
      | P+PCIN+(A+D)*B+CARRYIN
      | P+PCIN+(A+D)+CARRYIN
      | P+PCIN+(D+A)
      | P+PCIN+(D+A)*B
      | P+PCIN+(D+A)*B+CARRYIN
      | P+PCIN+(D+A)+CARRYIN
      | P+PCIN+(D-A)
      | P+PCIN+(D-A)*B
      | P+PCIN+(D-A)*B+CARRYIN
      | P+PCIN+(D-A)+CARRYIN
      | P+PCIN+A
      | P+PCIN+A*B
      | P+PCIN+A*B+CARRYIN
      | P+PCIN+A+CARRYIN
      | P+PCIN+B*(A+D)
      | P+PCIN+B*(A+D)+CARRYIN
      | P+PCIN+B*(D+A)
      | P+PCIN+B*(D+A)+CARRYIN
      | P+PCIN+B*(D-A)
      | P+PCIN+B*(D-A)+CARRYIN
      | P+PCIN+B*A
      | P+PCIN+B*A+CARRYIN
      | P+PCIN+B*D
      | P+PCIN+B*D+CARRYIN
      | P+PCIN+C
      | P+PCIN+C+C
      | P+PCIN+C+C+CARRYIN
      | P+PCIN+C+CARRYIN
      | P+PCIN+C+P
      | P+PCIN+C+P+CARRYIN
      | P+PCIN+CARRYIN
      | P+PCIN+D
      | P+PCIN+D*B
      | P+PCIN+D*B+CARRYIN
      | P+PCIN+D+CARRYIN
      | P+PCIN+P
      | P+PCIN+P+C
      | P+PCIN+P+C+CARRYIN
      | P+PCIN+P+CARRYIN
      | P+PCIN>>17
      | P+PCIN>>17+(A+D)
      | P+PCIN>>17+(A+D)*B
      | P+PCIN>>17+(A+D)*B+CARRYIN
      | P+PCIN>>17+(A+D)+CARRYIN
      | P+PCIN>>17+(D+A)
      | P+PCIN>>17+(D+A)*B
      | P+PCIN>>17+(D+A)*B+CARRYIN
      | P+PCIN>>17+(D+A)+CARRYIN
      | P+PCIN>>17+(D-A)
      | P+PCIN>>17+(D-A)*B
      | P+PCIN>>17+(D-A)*B+CARRYIN
      | P+PCIN>>17+(D-A)+CARRYIN
      | P+PCIN>>17+A
      | P+PCIN>>17+A*B
      | P+PCIN>>17+A*B+CARRYIN
      | P+PCIN>>17+A+CARRYIN
      | P+PCIN>>17+B*(A+D)
      | P+PCIN>>17+B*(A+D)+CARRYIN
      | P+PCIN>>17+B*(D+A)
      | P+PCIN>>17+B*(D+A)+CARRYIN
      | P+PCIN>>17+B*(D-A)
      | P+PCIN>>17+B*(D-A)+CARRYIN
      | P+PCIN>>17+B*A
      | P+PCIN>>17+B*A+CARRYIN
      | P+PCIN>>17+B*D
      | P+PCIN>>17+B*D+CARRYIN
      | P+PCIN>>17+C
      | P+PCIN>>17+C+C
      | P+PCIN>>17+C+C+CARRYIN
      | P+PCIN>>17+C+CARRYIN
      | P+PCIN>>17+C+P
      | P+PCIN>>17+C+P+CARRYIN
      | P+PCIN>>17+CARRYIN
      | P+PCIN>>17+D
      | P+PCIN>>17+D*B
      | P+PCIN>>17+D*B+CARRYIN
      | P+PCIN>>17+D+CARRYIN
      | P+PCIN>>17+P
      | P+PCIN>>17+P+C
      | P+PCIN>>17+P+C+CARRYIN
      | P+PCIN>>17+P+CARRYIN
      | P-((A+D))
      | P-((A+D)*B)
      | P-((A+D)*B+C)
      | P-((A+D)*B+C+CARRYIN)
      | P-((A+D)*B+CARRYIN)
      | P-((A+D)*B+P)
      | P-((A+D)*B+P+CARRYIN)
      | P-((A+D)+C)
      | P-((A+D)+C+CARRYIN)
      | P-((A+D)+CARRYIN)
      | P-((A+D)+P)
      | P-((A+D)+P+CARRYIN)
      | P-((D+A))
      | P-((D+A)*B)
      | P-((D+A)*B+C)
      | P-((D+A)*B+C+CARRYIN)
      | P-((D+A)*B+CARRYIN)
      | P-((D+A)*B+P)
      | P-((D+A)*B+P+CARRYIN)
      | P-((D+A)+C)
      | P-((D+A)+C+CARRYIN)
      | P-((D+A)+CARRYIN)
      | P-((D+A)+P)
      | P-((D+A)+P+CARRYIN)
      | P-((D-A))
      | P-((D-A)*B)
      | P-((D-A)*B+C)
      | P-((D-A)*B+C+CARRYIN)
      | P-((D-A)*B+CARRYIN)
      | P-((D-A)*B+P)
      | P-((D-A)*B+P+CARRYIN)
      | P-((D-A)+C)
      | P-((D-A)+C+CARRYIN)
      | P-((D-A)+CARRYIN)
      | P-((D-A)+P)
      | P-((D-A)+P+CARRYIN)
      | P-(A)
      | P-(A*B)
      | P-(A*B+C)
      | P-(A*B+C+CARRYIN)
      | P-(A*B+CARRYIN)
      | P-(A*B+P)
      | P-(A*B+P+CARRYIN)
      | P-(A+C)
      | P-(A+C+CARRYIN)
      | P-(A+CARRYIN)
      | P-(A+D)
      | P-(A+D)*B
      | P-(A+D)*B-C
      | P-(A+D)*B-C-CARRYIN
      | P-(A+D)*B-CARRYIN
      | P-(A+D)*B-P
      | P-(A+D)*B-P-CARRYIN
      | P-(A+D)-C
      | P-(A+D)-C-CARRYIN
      | P-(A+D)-CARRYIN
      | P-(A+D)-P
      | P-(A+D)-P-CARRYIN
      | P-(A+P)
      | P-(A+P+CARRYIN)
      | P-(B*(A+D))
      | P-(B*(A+D)+C)
      | P-(B*(A+D)+C+CARRYIN)
      | P-(B*(A+D)+CARRYIN)
      | P-(B*(A+D)+P)
      | P-(B*(A+D)+P+CARRYIN)
      | P-(B*(D+A))
      | P-(B*(D+A)+C)
      | P-(B*(D+A)+C+CARRYIN)
      | P-(B*(D+A)+CARRYIN)
      | P-(B*(D+A)+P)
      | P-(B*(D+A)+P+CARRYIN)
      | P-(B*(D-A))
      | P-(B*(D-A)+C)
      | P-(B*(D-A)+C+CARRYIN)
      | P-(B*(D-A)+CARRYIN)
      | P-(B*(D-A)+P)
      | P-(B*(D-A)+P+CARRYIN)
      | P-(B*A)
      | P-(B*A+C)
      | P-(B*A+C+CARRYIN)
      | P-(B*A+CARRYIN)
      | P-(B*A+P)
      | P-(B*A+P+CARRYIN)
      | P-(B*D)
      | P-(B*D+C)
      | P-(B*D+C+CARRYIN)
      | P-(B*D+CARRYIN)
      | P-(B*D+P)
      | P-(B*D+P+CARRYIN)
      | P-(C)
      | P-(C+(A+D))
      | P-(C+(A+D)*B)
      | P-(C+(A+D)*B+CARRYIN)
      | P-(C+(A+D)+CARRYIN)
      | P-(C+(D+A))
      | P-(C+(D+A)*B)
      | P-(C+(D+A)*B+CARRYIN)
      | P-(C+(D+A)+CARRYIN)
      | P-(C+(D-A))
      | P-(C+(D-A)*B)
      | P-(C+(D-A)*B+CARRYIN)
      | P-(C+(D-A)+CARRYIN)
      | P-(C+A)
      | P-(C+A*B)
      | P-(C+A*B+CARRYIN)
      | P-(C+A+CARRYIN)
      | P-(C+B*(A+D))
      | P-(C+B*(A+D)+CARRYIN)
      | P-(C+B*(D+A))
      | P-(C+B*(D+A)+CARRYIN)
      | P-(C+B*(D-A))
      | P-(C+B*(D-A)+CARRYIN)
      | P-(C+B*A)
      | P-(C+B*A+CARRYIN)
      | P-(C+B*D)
      | P-(C+B*D+CARRYIN)
      | P-(C+C)
      | P-(C+C+CARRYIN)
      | P-(C+C+P)
      | P-(C+C+P+CARRYIN)
      | P-(C+CARRYCASCIN)
      | P-(C+CARRYIN)
      | P-(C+D)
      | P-(C+D*B)
      | P-(C+D*B+CARRYIN)
      | P-(C+D+CARRYIN)
      | P-(C+P)
      | P-(C+P+C)
      | P-(C+P+C+CARRYIN)
      | P-(C+P+CARRYIN)
      | P-(C+P+P)
      | P-(C+P+P+CARRYIN)
      | P-(CARRYCASCIN)
      | P-(CARRYIN)
      | P-(D)
      | P-(D*B)
      | P-(D*B+C)
      | P-(D*B+C+CARRYIN)
      | P-(D*B+CARRYIN)
      | P-(D*B+P)
      | P-(D*B+P+CARRYIN)
      | P-(D+A)
      | P-(D+A)*B
      | P-(D+A)*B-C
      | P-(D+A)*B-C-CARRYIN
      | P-(D+A)*B-CARRYIN
      | P-(D+A)*B-P
      | P-(D+A)*B-P-CARRYIN
      | P-(D+A)-C
      | P-(D+A)-C-CARRYIN
      | P-(D+A)-CARRYIN
      | P-(D+A)-P
      | P-(D+A)-P-CARRYIN
      | P-(D+C)
      | P-(D+C+CARRYIN)
      | P-(D+CARRYIN)
      | P-(D+P)
      | P-(D+P+CARRYIN)
      | P-(D-A)
      | P-(D-A)*B
      | P-(D-A)*B-C
      | P-(D-A)*B-C-CARRYIN
      | P-(D-A)*B-CARRYIN
      | P-(D-A)*B-P
      | P-(D-A)*B-P-CARRYIN
      | P-(D-A)-C
      | P-(D-A)-C-CARRYIN
      | P-(D-A)-CARRYIN
      | P-(D-A)-P
      | P-(D-A)-P-CARRYIN
      | P-(P)
      | P-(P+(A+D))
      | P-(P+(A+D)*B)
      | P-(P+(A+D)*B+CARRYIN)
      | P-(P+(A+D)+CARRYIN)
      | P-(P+(D+A))
      | P-(P+(D+A)*B)
      | P-(P+(D+A)*B+CARRYIN)
      | P-(P+(D+A)+CARRYIN)
      | P-(P+(D-A))
      | P-(P+(D-A)*B)
      | P-(P+(D-A)*B+CARRYIN)
      | P-(P+(D-A)+CARRYIN)
      | P-(P+A)
      | P-(P+A*B)
      | P-(P+A*B+CARRYIN)
      | P-(P+A+CARRYIN)
      | P-(P+B*(A+D))
      | P-(P+B*(A+D)+CARRYIN)
      | P-(P+B*(D+A))
      | P-(P+B*(D+A)+CARRYIN)
      | P-(P+B*(D-A))
      | P-(P+B*(D-A)+CARRYIN)
      | P-(P+B*A)
      | P-(P+B*A+CARRYIN)
      | P-(P+B*D)
      | P-(P+B*D+CARRYIN)
      | P-(P+C)
      | P-(P+C+C)
      | P-(P+C+C+CARRYIN)
      | P-(P+C+CARRYIN)
      | P-(P+C+P)
      | P-(P+C+P+CARRYIN)
      | P-(P+CARRYCASCIN)
      | P-(P+CARRYIN)
      | P-(P+D)
      | P-(P+D*B)
      | P-(P+D*B+CARRYIN)
      | P-(P+D+CARRYIN)
      | P-(P+P)
      | P-(P+P+C)
      | P-(P+P+C+CARRYIN)
      | P-(P+P+CARRYIN)
      | P-A
      | P-A*B
      | P-A*B-C
      | P-A*B-C-CARRYIN
      | P-A*B-CARRYIN
      | P-A*B-P
      | P-A*B-P-CARRYIN
      | P-A-C
      | P-A-C-CARRYIN
      | P-A-CARRYIN
      | P-A-P
      | P-A-P-CARRYIN
      | P-B*(A+D)
      | P-B*(A+D)-C
      | P-B*(A+D)-C-CARRYIN
      | P-B*(A+D)-CARRYIN
      | P-B*(A+D)-P
      | P-B*(A+D)-P-CARRYIN
      | P-B*(D+A)
      | P-B*(D+A)-C
      | P-B*(D+A)-C-CARRYIN
      | P-B*(D+A)-CARRYIN
      | P-B*(D+A)-P
      | P-B*(D+A)-P-CARRYIN
      | P-B*(D-A)
      | P-B*(D-A)-C
      | P-B*(D-A)-C-CARRYIN
      | P-B*(D-A)-CARRYIN
      | P-B*(D-A)-P
      | P-B*(D-A)-P-CARRYIN
      | P-B*A
      | P-B*A-C
      | P-B*A-C-CARRYIN
      | P-B*A-CARRYIN
      | P-B*A-P
      | P-B*A-P-CARRYIN
      | P-B*D
      | P-B*D-C
      | P-B*D-C-CARRYIN
      | P-B*D-CARRYIN
      | P-B*D-P
      | P-B*D-P-CARRYIN
      | P-C
      | P-C-(A+D)
      | P-C-(A+D)*B
      | P-C-(A+D)*B-CARRYIN
      | P-C-(A+D)-CARRYIN
      | P-C-(D+A)
      | P-C-(D+A)*B
      | P-C-(D+A)*B-CARRYIN
      | P-C-(D+A)-CARRYIN
      | P-C-(D-A)
      | P-C-(D-A)*B
      | P-C-(D-A)*B-CARRYIN
      | P-C-(D-A)-CARRYIN
      | P-C-A
      | P-C-A*B
      | P-C-A*B-CARRYIN
      | P-C-A-CARRYIN
      | P-C-B*(A+D)
      | P-C-B*(A+D)-CARRYIN
      | P-C-B*(D+A)
      | P-C-B*(D+A)-CARRYIN
      | P-C-B*(D-A)
      | P-C-B*(D-A)-CARRYIN
      | P-C-B*A
      | P-C-B*A-CARRYIN
      | P-C-B*D
      | P-C-B*D-CARRYIN
      | P-C-C
      | P-C-C-CARRYIN
      | P-C-C-P
      | P-C-C-P-CARRYIN
      | P-C-CARRYCASCIN
      | P-C-CARRYIN
      | P-C-D
      | P-C-D*B
      | P-C-D*B-CARRYIN
      | P-C-D-CARRYIN
      | P-C-P
      | P-C-P-C
      | P-C-P-C-CARRYIN
      | P-C-P-CARRYIN
      | P-C-P-P
      | P-C-P-P-CARRYIN
      | P-CARRYCASCIN
      | P-CARRYIN
      | P-D
      | P-D*B
      | P-D*B-C
      | P-D*B-C-CARRYIN
      | P-D*B-CARRYIN
      | P-D*B-P
      | P-D*B-P-CARRYIN
      | P-D-C
      | P-D-C-CARRYIN
      | P-D-CARRYIN
      | P-D-P
      | P-D-P-CARRYIN
      | P-P
      | P-P-(A+D)
      | P-P-(A+D)*B
      | P-P-(A+D)*B-CARRYIN
      | P-P-(A+D)-CARRYIN
      | P-P-(D+A)
      | P-P-(D+A)*B
      | P-P-(D+A)*B-CARRYIN
      | P-P-(D+A)-CARRYIN
      | P-P-(D-A)
      | P-P-(D-A)*B
      | P-P-(D-A)*B-CARRYIN
      | P-P-(D-A)-CARRYIN
      | P-P-A
      | P-P-A*B
      | P-P-A*B-CARRYIN
      | P-P-A-CARRYIN
      | P-P-B*(A+D)
      | P-P-B*(A+D)-CARRYIN
      | P-P-B*(D+A)
      | P-P-B*(D+A)-CARRYIN
      | P-P-B*(D-A)
      | P-P-B*(D-A)-CARRYIN
      | P-P-B*A
      | P-P-B*A-CARRYIN
      | P-P-B*D
      | P-P-B*D-CARRYIN
      | P-P-C
      | P-P-C-C
      | P-P-C-C-CARRYIN
      | P-P-C-CARRYIN
      | P-P-C-P
      | P-P-C-P-CARRYIN
      | P-P-CARRYCASCIN
      | P-P-CARRYIN
      | P-P-D
      | P-P-D*B
      | P-P-D*B-CARRYIN
      | P-P-D-CARRYIN
      | P-P-P
      | P-P-P-C
      | P-P-P-C-CARRYIN
      | P-P-P-CARRYIN
      | P-P>>17
      | P-PCIN
      | P-PCIN>>17
      | P>>17
      | P>>17+(A+D)
      | P>>17+(A+D)*B
      | P>>17+(A+D)*B+C
      | P>>17+(A+D)*B+C+CARRYIN
      | P>>17+(A+D)*B+CARRYIN
      | P>>17+(A+D)*B+P
      | P>>17+(A+D)*B+P+CARRYIN
      | P>>17+(A+D)+C
      | P>>17+(A+D)+C+CARRYIN
      | P>>17+(A+D)+CARRYIN
      | P>>17+(A+D)+P
      | P>>17+(A+D)+P+CARRYIN
      | P>>17+(D+A)
      | P>>17+(D+A)*B
      | P>>17+(D+A)*B+C
      | P>>17+(D+A)*B+C+CARRYIN
      | P>>17+(D+A)*B+CARRYIN
      | P>>17+(D+A)*B+P
      | P>>17+(D+A)*B+P+CARRYIN
      | P>>17+(D+A)+C
      | P>>17+(D+A)+C+CARRYIN
      | P>>17+(D+A)+CARRYIN
      | P>>17+(D+A)+P
      | P>>17+(D+A)+P+CARRYIN
      | P>>17+(D-A)
      | P>>17+(D-A)*B
      | P>>17+(D-A)*B+C
      | P>>17+(D-A)*B+C+CARRYIN
      | P>>17+(D-A)*B+CARRYIN
      | P>>17+(D-A)*B+P
      | P>>17+(D-A)*B+P+CARRYIN
      | P>>17+(D-A)+C
      | P>>17+(D-A)+C+CARRYIN
      | P>>17+(D-A)+CARRYIN
      | P>>17+(D-A)+P
      | P>>17+(D-A)+P+CARRYIN
      | P>>17+A
      | P>>17+A*B
      | P>>17+A*B+C
      | P>>17+A*B+C+CARRYIN
      | P>>17+A*B+CARRYIN
      | P>>17+A*B+P
      | P>>17+A*B+P+CARRYIN
      | P>>17+A+C
      | P>>17+A+C+CARRYIN
      | P>>17+A+CARRYIN
      | P>>17+A+P
      | P>>17+A+P+CARRYIN
      | P>>17+B*(A+D)
      | P>>17+B*(A+D)+C
      | P>>17+B*(A+D)+C+CARRYIN
      | P>>17+B*(A+D)+CARRYIN
      | P>>17+B*(A+D)+P
      | P>>17+B*(A+D)+P+CARRYIN
      | P>>17+B*(D+A)
      | P>>17+B*(D+A)+C
      | P>>17+B*(D+A)+C+CARRYIN
      | P>>17+B*(D+A)+CARRYIN
      | P>>17+B*(D+A)+P
      | P>>17+B*(D+A)+P+CARRYIN
      | P>>17+B*(D-A)
      | P>>17+B*(D-A)+C
      | P>>17+B*(D-A)+C+CARRYIN
      | P>>17+B*(D-A)+CARRYIN
      | P>>17+B*(D-A)+P
      | P>>17+B*(D-A)+P+CARRYIN
      | P>>17+B*A
      | P>>17+B*A+C
      | P>>17+B*A+C+CARRYIN
      | P>>17+B*A+CARRYIN
      | P>>17+B*A+P
      | P>>17+B*A+P+CARRYIN
      | P>>17+B*D
      | P>>17+B*D+C
      | P>>17+B*D+C+CARRYIN
      | P>>17+B*D+CARRYIN
      | P>>17+B*D+P
      | P>>17+B*D+P+CARRYIN
      | P>>17+C
      | P>>17+C+(A+D)
      | P>>17+C+(A+D)*B
      | P>>17+C+(A+D)*B+CARRYIN
      | P>>17+C+(A+D)+CARRYIN
      | P>>17+C+(D+A)
      | P>>17+C+(D+A)*B
      | P>>17+C+(D+A)*B+CARRYIN
      | P>>17+C+(D+A)+CARRYIN
      | P>>17+C+(D-A)
      | P>>17+C+(D-A)*B
      | P>>17+C+(D-A)*B+CARRYIN
      | P>>17+C+(D-A)+CARRYIN
      | P>>17+C+A
      | P>>17+C+A*B
      | P>>17+C+A*B+CARRYIN
      | P>>17+C+A+CARRYIN
      | P>>17+C+B*(A+D)
      | P>>17+C+B*(A+D)+CARRYIN
      | P>>17+C+B*(D+A)
      | P>>17+C+B*(D+A)+CARRYIN
      | P>>17+C+B*(D-A)
      | P>>17+C+B*(D-A)+CARRYIN
      | P>>17+C+B*A
      | P>>17+C+B*A+CARRYIN
      | P>>17+C+B*D
      | P>>17+C+B*D+CARRYIN
      | P>>17+C+C
      | P>>17+C+C+CARRYIN
      | P>>17+C+C+P
      | P>>17+C+C+P+CARRYIN
      | P>>17+C+CARRYIN
      | P>>17+C+D
      | P>>17+C+D*B
      | P>>17+C+D*B+CARRYIN
      | P>>17+C+D+CARRYIN
      | P>>17+C+P
      | P>>17+C+P+C
      | P>>17+C+P+C+CARRYIN
      | P>>17+C+P+CARRYIN
      | P>>17+C+P+P
      | P>>17+C+P+P+CARRYIN
      | P>>17+CARRYIN
      | P>>17+D
      | P>>17+D*B
      | P>>17+D*B+C
      | P>>17+D*B+C+CARRYIN
      | P>>17+D*B+CARRYIN
      | P>>17+D*B+P
      | P>>17+D*B+P+CARRYIN
      | P>>17+D+C
      | P>>17+D+C+CARRYIN
      | P>>17+D+CARRYIN
      | P>>17+D+P
      | P>>17+D+P+CARRYIN
      | P>>17+P
      | P>>17+P+(A+D)
      | P>>17+P+(A+D)*B
      | P>>17+P+(A+D)*B+CARRYIN
      | P>>17+P+(A+D)+CARRYIN
      | P>>17+P+(D+A)
      | P>>17+P+(D+A)*B
      | P>>17+P+(D+A)*B+CARRYIN
      | P>>17+P+(D+A)+CARRYIN
      | P>>17+P+(D-A)
      | P>>17+P+(D-A)*B
      | P>>17+P+(D-A)*B+CARRYIN
      | P>>17+P+(D-A)+CARRYIN
      | P>>17+P+A
      | P>>17+P+A*B
      | P>>17+P+A*B+CARRYIN
      | P>>17+P+A+CARRYIN
      | P>>17+P+B*(A+D)
      | P>>17+P+B*(A+D)+CARRYIN
      | P>>17+P+B*(D+A)
      | P>>17+P+B*(D+A)+CARRYIN
      | P>>17+P+B*(D-A)
      | P>>17+P+B*(D-A)+CARRYIN
      | P>>17+P+B*A
      | P>>17+P+B*A+CARRYIN
      | P>>17+P+B*D
      | P>>17+P+B*D+CARRYIN
      | P>>17+P+C
      | P>>17+P+C+C
      | P>>17+P+C+C+CARRYIN
      | P>>17+P+C+CARRYIN
      | P>>17+P+C+P
      | P>>17+P+C+P+CARRYIN
      | P>>17+P+CARRYIN
      | P>>17+P+D
      | P>>17+P+D*B
      | P>>17+P+D*B+CARRYIN
      | P>>17+P+D+CARRYIN
      | P>>17+P+P
      | P>>17+P+P+C
      | P>>17+P+P+C+CARRYIN
      | P>>17+P+P+CARRYIN
      | P>>17-((A+D))
      | P>>17-((A+D)*B)
      | P>>17-((A+D)*B+C)
      | P>>17-((A+D)*B+C+CARRYIN)
      | P>>17-((A+D)*B+CARRYIN)
      | P>>17-((A+D)*B+P)
      | P>>17-((A+D)*B+P+CARRYIN)
      | P>>17-((A+D)+C)
      | P>>17-((A+D)+C+CARRYIN)
      | P>>17-((A+D)+CARRYIN)
      | P>>17-((A+D)+P)
      | P>>17-((A+D)+P+CARRYIN)
      | P>>17-((D+A))
      | P>>17-((D+A)*B)
      | P>>17-((D+A)*B+C)
      | P>>17-((D+A)*B+C+CARRYIN)
      | P>>17-((D+A)*B+CARRYIN)
      | P>>17-((D+A)*B+P)
      | P>>17-((D+A)*B+P+CARRYIN)
      | P>>17-((D+A)+C)
      | P>>17-((D+A)+C+CARRYIN)
      | P>>17-((D+A)+CARRYIN)
      | P>>17-((D+A)+P)
      | P>>17-((D+A)+P+CARRYIN)
      | P>>17-((D-A))
      | P>>17-((D-A)*B)
      | P>>17-((D-A)*B+C)
      | P>>17-((D-A)*B+C+CARRYIN)
      | P>>17-((D-A)*B+CARRYIN)
      | P>>17-((D-A)*B+P)
      | P>>17-((D-A)*B+P+CARRYIN)
      | P>>17-((D-A)+C)
      | P>>17-((D-A)+C+CARRYIN)
      | P>>17-((D-A)+CARRYIN)
      | P>>17-((D-A)+P)
      | P>>17-((D-A)+P+CARRYIN)
      | P>>17-(A)
      | P>>17-(A*B)
      | P>>17-(A*B+C)
      | P>>17-(A*B+C+CARRYIN)
      | P>>17-(A*B+CARRYIN)
      | P>>17-(A*B+P)
      | P>>17-(A*B+P+CARRYIN)
      | P>>17-(A+C)
      | P>>17-(A+C+CARRYIN)
      | P>>17-(A+CARRYIN)
      | P>>17-(A+D)
      | P>>17-(A+D)*B
      | P>>17-(A+D)*B-C
      | P>>17-(A+D)*B-C-CARRYIN
      | P>>17-(A+D)*B-CARRYIN
      | P>>17-(A+D)*B-P
      | P>>17-(A+D)*B-P-CARRYIN
      | P>>17-(A+D)-C
      | P>>17-(A+D)-C-CARRYIN
      | P>>17-(A+D)-CARRYIN
      | P>>17-(A+D)-P
      | P>>17-(A+D)-P-CARRYIN
      | P>>17-(A+P)
      | P>>17-(A+P+CARRYIN)
      | P>>17-(B*(A+D))
      | P>>17-(B*(A+D)+C)
      | P>>17-(B*(A+D)+C+CARRYIN)
      | P>>17-(B*(A+D)+CARRYIN)
      | P>>17-(B*(A+D)+P)
      | P>>17-(B*(A+D)+P+CARRYIN)
      | P>>17-(B*(D+A))
      | P>>17-(B*(D+A)+C)
      | P>>17-(B*(D+A)+C+CARRYIN)
      | P>>17-(B*(D+A)+CARRYIN)
      | P>>17-(B*(D+A)+P)
      | P>>17-(B*(D+A)+P+CARRYIN)
      | P>>17-(B*(D-A))
      | P>>17-(B*(D-A)+C)
      | P>>17-(B*(D-A)+C+CARRYIN)
      | P>>17-(B*(D-A)+CARRYIN)
      | P>>17-(B*(D-A)+P)
      | P>>17-(B*(D-A)+P+CARRYIN)
      | P>>17-(B*A)
      | P>>17-(B*A+C)
      | P>>17-(B*A+C+CARRYIN)
      | P>>17-(B*A+CARRYIN)
      | P>>17-(B*A+P)
      | P>>17-(B*A+P+CARRYIN)
      | P>>17-(B*D)
      | P>>17-(B*D+C)
      | P>>17-(B*D+C+CARRYIN)
      | P>>17-(B*D+CARRYIN)
      | P>>17-(B*D+P)
      | P>>17-(B*D+P+CARRYIN)
      | P>>17-(C)
      | P>>17-(C+(A+D))
      | P>>17-(C+(A+D)*B)
      | P>>17-(C+(A+D)*B+CARRYIN)
      | P>>17-(C+(A+D)+CARRYIN)
      | P>>17-(C+(D+A))
      | P>>17-(C+(D+A)*B)
      | P>>17-(C+(D+A)*B+CARRYIN)
      | P>>17-(C+(D+A)+CARRYIN)
      | P>>17-(C+(D-A))
      | P>>17-(C+(D-A)*B)
      | P>>17-(C+(D-A)*B+CARRYIN)
      | P>>17-(C+(D-A)+CARRYIN)
      | P>>17-(C+A)
      | P>>17-(C+A*B)
      | P>>17-(C+A*B+CARRYIN)
      | P>>17-(C+A+CARRYIN)
      | P>>17-(C+B*(A+D))
      | P>>17-(C+B*(A+D)+CARRYIN)
      | P>>17-(C+B*(D+A))
      | P>>17-(C+B*(D+A)+CARRYIN)
      | P>>17-(C+B*(D-A))
      | P>>17-(C+B*(D-A)+CARRYIN)
      | P>>17-(C+B*A)
      | P>>17-(C+B*A+CARRYIN)
      | P>>17-(C+B*D)
      | P>>17-(C+B*D+CARRYIN)
      | P>>17-(C+C)
      | P>>17-(C+C+CARRYIN)
      | P>>17-(C+C+P)
      | P>>17-(C+C+P+CARRYIN)
      | P>>17-(C+CARRYIN)
      | P>>17-(C+D)
      | P>>17-(C+D*B)
      | P>>17-(C+D*B+CARRYIN)
      | P>>17-(C+D+CARRYIN)
      | P>>17-(C+P)
      | P>>17-(C+P+C)
      | P>>17-(C+P+C+CARRYIN)
      | P>>17-(C+P+CARRYIN)
      | P>>17-(C+P+P)
      | P>>17-(C+P+P+CARRYIN)
      | P>>17-(CARRYIN)
      | P>>17-(D)
      | P>>17-(D*B)
      | P>>17-(D*B+C)
      | P>>17-(D*B+C+CARRYIN)
      | P>>17-(D*B+CARRYIN)
      | P>>17-(D*B+P)
      | P>>17-(D*B+P+CARRYIN)
      | P>>17-(D+A)
      | P>>17-(D+A)*B
      | P>>17-(D+A)*B-C
      | P>>17-(D+A)*B-C-CARRYIN
      | P>>17-(D+A)*B-CARRYIN
      | P>>17-(D+A)*B-P
      | P>>17-(D+A)*B-P-CARRYIN
      | P>>17-(D+A)-C
      | P>>17-(D+A)-C-CARRYIN
      | P>>17-(D+A)-CARRYIN
      | P>>17-(D+A)-P
      | P>>17-(D+A)-P-CARRYIN
      | P>>17-(D+C)
      | P>>17-(D+C+CARRYIN)
      | P>>17-(D+CARRYIN)
      | P>>17-(D+P)
      | P>>17-(D+P+CARRYIN)
      | P>>17-(D-A)
      | P>>17-(D-A)*B
      | P>>17-(D-A)*B-C
      | P>>17-(D-A)*B-C-CARRYIN
      | P>>17-(D-A)*B-CARRYIN
      | P>>17-(D-A)*B-P
      | P>>17-(D-A)*B-P-CARRYIN
      | P>>17-(D-A)-C
      | P>>17-(D-A)-C-CARRYIN
      | P>>17-(D-A)-CARRYIN
      | P>>17-(D-A)-P
      | P>>17-(D-A)-P-CARRYIN
      | P>>17-(P)
      | P>>17-(P+(A+D))
      | P>>17-(P+(A+D)*B)
      | P>>17-(P+(A+D)*B+CARRYIN)
      | P>>17-(P+(A+D)+CARRYIN)
      | P>>17-(P+(D+A))
      | P>>17-(P+(D+A)*B)
      | P>>17-(P+(D+A)*B+CARRYIN)
      | P>>17-(P+(D+A)+CARRYIN)
      | P>>17-(P+(D-A))
      | P>>17-(P+(D-A)*B)
      | P>>17-(P+(D-A)*B+CARRYIN)
      | P>>17-(P+(D-A)+CARRYIN)
      | P>>17-(P+A)
      | P>>17-(P+A*B)
      | P>>17-(P+A*B+CARRYIN)
      | P>>17-(P+A+CARRYIN)
      | P>>17-(P+B*(A+D))
      | P>>17-(P+B*(A+D)+CARRYIN)
      | P>>17-(P+B*(D+A))
      | P>>17-(P+B*(D+A)+CARRYIN)
      | P>>17-(P+B*(D-A))
      | P>>17-(P+B*(D-A)+CARRYIN)
      | P>>17-(P+B*A)
      | P>>17-(P+B*A+CARRYIN)
      | P>>17-(P+B*D)
      | P>>17-(P+B*D+CARRYIN)
      | P>>17-(P+C)
      | P>>17-(P+C+C)
      | P>>17-(P+C+C+CARRYIN)
      | P>>17-(P+C+CARRYIN)
      | P>>17-(P+C+P)
      | P>>17-(P+C+P+CARRYIN)
      | P>>17-(P+CARRYIN)
      | P>>17-(P+D)
      | P>>17-(P+D*B)
      | P>>17-(P+D*B+CARRYIN)
      | P>>17-(P+D+CARRYIN)
      | P>>17-(P+P)
      | P>>17-(P+P+C)
      | P>>17-(P+P+C+CARRYIN)
      | P>>17-(P+P+CARRYIN)
      | P>>17-A
      | P>>17-A*B
      | P>>17-A*B-C
      | P>>17-A*B-C-CARRYIN
      | P>>17-A*B-CARRYIN
      | P>>17-A*B-P
      | P>>17-A*B-P-CARRYIN
      | P>>17-A-C
      | P>>17-A-C-CARRYIN
      | P>>17-A-CARRYIN
      | P>>17-A-P
      | P>>17-A-P-CARRYIN
      | P>>17-B*(A+D)
      | P>>17-B*(A+D)-C
      | P>>17-B*(A+D)-C-CARRYIN
      | P>>17-B*(A+D)-CARRYIN
      | P>>17-B*(A+D)-P
      | P>>17-B*(A+D)-P-CARRYIN
      | P>>17-B*(D+A)
      | P>>17-B*(D+A)-C
      | P>>17-B*(D+A)-C-CARRYIN
      | P>>17-B*(D+A)-CARRYIN
      | P>>17-B*(D+A)-P
      | P>>17-B*(D+A)-P-CARRYIN
      | P>>17-B*(D-A)
      | P>>17-B*(D-A)-C
      | P>>17-B*(D-A)-C-CARRYIN
      | P>>17-B*(D-A)-CARRYIN
      | P>>17-B*(D-A)-P
      | P>>17-B*(D-A)-P-CARRYIN
      | P>>17-B*A
      | P>>17-B*A-C
      | P>>17-B*A-C-CARRYIN
      | P>>17-B*A-CARRYIN
      | P>>17-B*A-P
      | P>>17-B*A-P-CARRYIN
      | P>>17-B*D
      | P>>17-B*D-C
      | P>>17-B*D-C-CARRYIN
      | P>>17-B*D-CARRYIN
      | P>>17-B*D-P
      | P>>17-B*D-P-CARRYIN
      | P>>17-C
      | P>>17-C-(A+D)
      | P>>17-C-(A+D)*B
      | P>>17-C-(A+D)*B-CARRYIN
      | P>>17-C-(A+D)-CARRYIN
      | P>>17-C-(D+A)
      | P>>17-C-(D+A)*B
      | P>>17-C-(D+A)*B-CARRYIN
      | P>>17-C-(D+A)-CARRYIN
      | P>>17-C-(D-A)
      | P>>17-C-(D-A)*B
      | P>>17-C-(D-A)*B-CARRYIN
      | P>>17-C-(D-A)-CARRYIN
      | P>>17-C-A
      | P>>17-C-A*B
      | P>>17-C-A*B-CARRYIN
      | P>>17-C-A-CARRYIN
      | P>>17-C-B*(A+D)
      | P>>17-C-B*(A+D)-CARRYIN
      | P>>17-C-B*(D+A)
      | P>>17-C-B*(D+A)-CARRYIN
      | P>>17-C-B*(D-A)
      | P>>17-C-B*(D-A)-CARRYIN
      | P>>17-C-B*A
      | P>>17-C-B*A-CARRYIN
      | P>>17-C-B*D
      | P>>17-C-B*D-CARRYIN
      | P>>17-C-C
      | P>>17-C-C-CARRYIN
      | P>>17-C-C-P
      | P>>17-C-C-P-CARRYIN
      | P>>17-C-CARRYIN
      | P>>17-C-D
      | P>>17-C-D*B
      | P>>17-C-D*B-CARRYIN
      | P>>17-C-D-CARRYIN
      | P>>17-C-P
      | P>>17-C-P-C
      | P>>17-C-P-C-CARRYIN
      | P>>17-C-P-CARRYIN
      | P>>17-C-P-P
      | P>>17-C-P-P-CARRYIN
      | P>>17-CARRYIN
      | P>>17-D
      | P>>17-D*B
      | P>>17-D*B-C
      | P>>17-D*B-C-CARRYIN
      | P>>17-D*B-CARRYIN
      | P>>17-D*B-P
      | P>>17-D*B-P-CARRYIN
      | P>>17-D-C
      | P>>17-D-C-CARRYIN
      | P>>17-D-CARRYIN
      | P>>17-D-P
      | P>>17-D-P-CARRYIN
      | P>>17-P
      | P>>17-P-(A+D)
      | P>>17-P-(A+D)*B
      | P>>17-P-(A+D)*B-CARRYIN
      | P>>17-P-(A+D)-CARRYIN
      | P>>17-P-(D+A)
      | P>>17-P-(D+A)*B
      | P>>17-P-(D+A)*B-CARRYIN
      | P>>17-P-(D+A)-CARRYIN
      | P>>17-P-(D-A)
      | P>>17-P-(D-A)*B
      | P>>17-P-(D-A)*B-CARRYIN
      | P>>17-P-(D-A)-CARRYIN
      | P>>17-P-A
      | P>>17-P-A*B
      | P>>17-P-A*B-CARRYIN
      | P>>17-P-A-CARRYIN
      | P>>17-P-B*(A+D)
      | P>>17-P-B*(A+D)-CARRYIN
      | P>>17-P-B*(D+A)
      | P>>17-P-B*(D+A)-CARRYIN
      | P>>17-P-B*(D-A)
      | P>>17-P-B*(D-A)-CARRYIN
      | P>>17-P-B*A
      | P>>17-P-B*A-CARRYIN
      | P>>17-P-B*D
      | P>>17-P-B*D-CARRYIN
      | P>>17-P-C
      | P>>17-P-C-C
      | P>>17-P-C-C-CARRYIN
      | P>>17-P-C-CARRYIN
      | P>>17-P-C-P
      | P>>17-P-C-P-CARRYIN
      | P>>17-P-CARRYIN
      | P>>17-P-D
      | P>>17-P-D*B
      | P>>17-P-D*B-CARRYIN
      | P>>17-P-D-CARRYIN
      | P>>17-P-P
      | P>>17-P-P-C
      | P>>17-P-P-C-CARRYIN
      | P>>17-P-P-CARRYIN
      | PCIN
      | PCIN+(A+D)
      | PCIN+(A+D)*B
      | PCIN+(A+D)*B+C
      | PCIN+(A+D)*B+C+CARRYIN
      | PCIN+(A+D)*B+CARRYIN
      | PCIN+(A+D)*B+P
      | PCIN+(A+D)*B+P+CARRYIN
      | PCIN+(A+D)+C
      | PCIN+(A+D)+C+CARRYIN
      | PCIN+(A+D)+CARRYIN
      | PCIN+(A+D)+P
      | PCIN+(A+D)+P+CARRYIN
      | PCIN+(D+A)
      | PCIN+(D+A)*B
      | PCIN+(D+A)*B+C
      | PCIN+(D+A)*B+C+CARRYIN
      | PCIN+(D+A)*B+CARRYIN
      | PCIN+(D+A)*B+P
      | PCIN+(D+A)*B+P+CARRYIN
      | PCIN+(D+A)+C
      | PCIN+(D+A)+C+CARRYIN
      | PCIN+(D+A)+CARRYIN
      | PCIN+(D+A)+P
      | PCIN+(D+A)+P+CARRYIN
      | PCIN+(D-A)
      | PCIN+(D-A)*B
      | PCIN+(D-A)*B+C
      | PCIN+(D-A)*B+C+CARRYIN
      | PCIN+(D-A)*B+CARRYIN
      | PCIN+(D-A)*B+P
      | PCIN+(D-A)*B+P+CARRYIN
      | PCIN+(D-A)+C
      | PCIN+(D-A)+C+CARRYIN
      | PCIN+(D-A)+CARRYIN
      | PCIN+(D-A)+P
      | PCIN+(D-A)+P+CARRYIN
      | PCIN+A
      | PCIN+A*B
      | PCIN+A*B+C
      | PCIN+A*B+C+CARRYIN
      | PCIN+A*B+CARRYIN
      | PCIN+A*B+P
      | PCIN+A*B+P+CARRYIN
      | PCIN+A+C
      | PCIN+A+C+CARRYIN
      | PCIN+A+CARRYIN
      | PCIN+A+P
      | PCIN+A+P+CARRYIN
      | PCIN+B*(A+D)
      | PCIN+B*(A+D)+C
      | PCIN+B*(A+D)+C+CARRYIN
      | PCIN+B*(A+D)+CARRYIN
      | PCIN+B*(A+D)+P
      | PCIN+B*(A+D)+P+CARRYIN
      | PCIN+B*(D+A)
      | PCIN+B*(D+A)+C
      | PCIN+B*(D+A)+C+CARRYIN
      | PCIN+B*(D+A)+CARRYIN
      | PCIN+B*(D+A)+P
      | PCIN+B*(D+A)+P+CARRYIN
      | PCIN+B*(D-A)
      | PCIN+B*(D-A)+C
      | PCIN+B*(D-A)+C+CARRYIN
      | PCIN+B*(D-A)+CARRYIN
      | PCIN+B*(D-A)+P
      | PCIN+B*(D-A)+P+CARRYIN
      | PCIN+B*A
      | PCIN+B*A+C
      | PCIN+B*A+C+CARRYIN
      | PCIN+B*A+CARRYIN
      | PCIN+B*A+P
      | PCIN+B*A+P+CARRYIN
      | PCIN+B*D
      | PCIN+B*D+C
      | PCIN+B*D+C+CARRYIN
      | PCIN+B*D+CARRYIN
      | PCIN+B*D+P
      | PCIN+B*D+P+CARRYIN
      | PCIN+C
      | PCIN+C+(A+D)
      | PCIN+C+(A+D)*B
      | PCIN+C+(A+D)*B+CARRYIN
      | PCIN+C+(A+D)+CARRYIN
      | PCIN+C+(D+A)
      | PCIN+C+(D+A)*B
      | PCIN+C+(D+A)*B+CARRYIN
      | PCIN+C+(D+A)+CARRYIN
      | PCIN+C+(D-A)
      | PCIN+C+(D-A)*B
      | PCIN+C+(D-A)*B+CARRYIN
      | PCIN+C+(D-A)+CARRYIN
      | PCIN+C+A
      | PCIN+C+A*B
      | PCIN+C+A*B+CARRYIN
      | PCIN+C+A+CARRYIN
      | PCIN+C+B*(A+D)
      | PCIN+C+B*(A+D)+CARRYIN
      | PCIN+C+B*(D+A)
      | PCIN+C+B*(D+A)+CARRYIN
      | PCIN+C+B*(D-A)
      | PCIN+C+B*(D-A)+CARRYIN
      | PCIN+C+B*A
      | PCIN+C+B*A+CARRYIN
      | PCIN+C+B*D
      | PCIN+C+B*D+CARRYIN
      | PCIN+C+C
      | PCIN+C+C+CARRYIN
      | PCIN+C+C+P
      | PCIN+C+C+P+CARRYIN
      | PCIN+C+CARRYIN
      | PCIN+C+D
      | PCIN+C+D*B
      | PCIN+C+D*B+CARRYIN
      | PCIN+C+D+CARRYIN
      | PCIN+C+P
      | PCIN+C+P+C
      | PCIN+C+P+C+CARRYIN
      | PCIN+C+P+CARRYIN
      | PCIN+C+P+P
      | PCIN+C+P+P+CARRYIN
      | PCIN+CARRYIN
      | PCIN+D
      | PCIN+D*B
      | PCIN+D*B+C
      | PCIN+D*B+C+CARRYIN
      | PCIN+D*B+CARRYIN
      | PCIN+D*B+P
      | PCIN+D*B+P+CARRYIN
      | PCIN+D+C
      | PCIN+D+C+CARRYIN
      | PCIN+D+CARRYIN
      | PCIN+D+P
      | PCIN+D+P+CARRYIN
      | PCIN+P
      | PCIN+P+(A+D)
      | PCIN+P+(A+D)*B
      | PCIN+P+(A+D)*B+CARRYIN
      | PCIN+P+(A+D)+CARRYIN
      | PCIN+P+(D+A)
      | PCIN+P+(D+A)*B
      | PCIN+P+(D+A)*B+CARRYIN
      | PCIN+P+(D+A)+CARRYIN
      | PCIN+P+(D-A)
      | PCIN+P+(D-A)*B
      | PCIN+P+(D-A)*B+CARRYIN
      | PCIN+P+(D-A)+CARRYIN
      | PCIN+P+A
      | PCIN+P+A*B
      | PCIN+P+A*B+CARRYIN
      | PCIN+P+A+CARRYIN
      | PCIN+P+B*(A+D)
      | PCIN+P+B*(A+D)+CARRYIN
      | PCIN+P+B*(D+A)
      | PCIN+P+B*(D+A)+CARRYIN
      | PCIN+P+B*(D-A)
      | PCIN+P+B*(D-A)+CARRYIN
      | PCIN+P+B*A
      | PCIN+P+B*A+CARRYIN
      | PCIN+P+B*D
      | PCIN+P+B*D+CARRYIN
      | PCIN+P+C
      | PCIN+P+C+C
      | PCIN+P+C+C+CARRYIN
      | PCIN+P+C+CARRYIN
      | PCIN+P+C+P
      | PCIN+P+C+P+CARRYIN
      | PCIN+P+CARRYIN
      | PCIN+P+D
      | PCIN+P+D*B
      | PCIN+P+D*B+CARRYIN
      | PCIN+P+D+CARRYIN
      | PCIN+P+P
      | PCIN+P+P+C
      | PCIN+P+P+C+CARRYIN
      | PCIN+P+P+CARRYIN
      | PCIN-((A+D))
      | PCIN-((A+D)*B)
      | PCIN-((A+D)*B+C)
      | PCIN-((A+D)*B+C+CARRYIN)
      | PCIN-((A+D)*B+CARRYIN)
      | PCIN-((A+D)*B+P)
      | PCIN-((A+D)*B+P+CARRYIN)
      | PCIN-((A+D)+C)
      | PCIN-((A+D)+C+CARRYIN)
      | PCIN-((A+D)+CARRYIN)
      | PCIN-((A+D)+P)
      | PCIN-((A+D)+P+CARRYIN)
      | PCIN-((D+A))
      | PCIN-((D+A)*B)
      | PCIN-((D+A)*B+C)
      | PCIN-((D+A)*B+C+CARRYIN)
      | PCIN-((D+A)*B+CARRYIN)
      | PCIN-((D+A)*B+P)
      | PCIN-((D+A)*B+P+CARRYIN)
      | PCIN-((D+A)+C)
      | PCIN-((D+A)+C+CARRYIN)
      | PCIN-((D+A)+CARRYIN)
      | PCIN-((D+A)+P)
      | PCIN-((D+A)+P+CARRYIN)
      | PCIN-((D-A))
      | PCIN-((D-A)*B)
      | PCIN-((D-A)*B+C)
      | PCIN-((D-A)*B+C+CARRYIN)
      | PCIN-((D-A)*B+CARRYIN)
      | PCIN-((D-A)*B+P)
      | PCIN-((D-A)*B+P+CARRYIN)
      | PCIN-((D-A)+C)
      | PCIN-((D-A)+C+CARRYIN)
      | PCIN-((D-A)+CARRYIN)
      | PCIN-((D-A)+P)
      | PCIN-((D-A)+P+CARRYIN)
      | PCIN-(A)
      | PCIN-(A*B)
      | PCIN-(A*B+C)
      | PCIN-(A*B+C+CARRYIN)
      | PCIN-(A*B+CARRYIN)
      | PCIN-(A*B+P)
      | PCIN-(A*B+P+CARRYIN)
      | PCIN-(A+C)
      | PCIN-(A+C+CARRYIN)
      | PCIN-(A+CARRYIN)
      | PCIN-(A+D)
      | PCIN-(A+D)*B
      | PCIN-(A+D)*B-C
      | PCIN-(A+D)*B-C-CARRYIN
      | PCIN-(A+D)*B-CARRYIN
      | PCIN-(A+D)*B-P
      | PCIN-(A+D)*B-P-CARRYIN
      | PCIN-(A+D)-C
      | PCIN-(A+D)-C-CARRYIN
      | PCIN-(A+D)-CARRYIN
      | PCIN-(A+D)-P
      | PCIN-(A+D)-P-CARRYIN
      | PCIN-(A+P)
      | PCIN-(A+P+CARRYIN)
      | PCIN-(B*(A+D))
      | PCIN-(B*(A+D)+C)
      | PCIN-(B*(A+D)+C+CARRYIN)
      | PCIN-(B*(A+D)+CARRYIN)
      | PCIN-(B*(A+D)+P)
      | PCIN-(B*(A+D)+P+CARRYIN)
      | PCIN-(B*(D+A))
      | PCIN-(B*(D+A)+C)
      | PCIN-(B*(D+A)+C+CARRYIN)
      | PCIN-(B*(D+A)+CARRYIN)
      | PCIN-(B*(D+A)+P)
      | PCIN-(B*(D+A)+P+CARRYIN)
      | PCIN-(B*(D-A))
      | PCIN-(B*(D-A)+C)
      | PCIN-(B*(D-A)+C+CARRYIN)
      | PCIN-(B*(D-A)+CARRYIN)
      | PCIN-(B*(D-A)+P)
      | PCIN-(B*(D-A)+P+CARRYIN)
      | PCIN-(B*A)
      | PCIN-(B*A+C)
      | PCIN-(B*A+C+CARRYIN)
      | PCIN-(B*A+CARRYIN)
      | PCIN-(B*A+P)
      | PCIN-(B*A+P+CARRYIN)
      | PCIN-(B*D)
      | PCIN-(B*D+C)
      | PCIN-(B*D+C+CARRYIN)
      | PCIN-(B*D+CARRYIN)
      | PCIN-(B*D+P)
      | PCIN-(B*D+P+CARRYIN)
      | PCIN-(C)
      | PCIN-(C+(A+D))
      | PCIN-(C+(A+D)*B)
      | PCIN-(C+(A+D)*B+CARRYIN)
      | PCIN-(C+(A+D)+CARRYIN)
      | PCIN-(C+(D+A))
      | PCIN-(C+(D+A)*B)
      | PCIN-(C+(D+A)*B+CARRYIN)
      | PCIN-(C+(D+A)+CARRYIN)
      | PCIN-(C+(D-A))
      | PCIN-(C+(D-A)*B)
      | PCIN-(C+(D-A)*B+CARRYIN)
      | PCIN-(C+(D-A)+CARRYIN)
      | PCIN-(C+A)
      | PCIN-(C+A*B)
      | PCIN-(C+A*B+CARRYIN)
      | PCIN-(C+A+CARRYIN)
      | PCIN-(C+B*(A+D))
      | PCIN-(C+B*(A+D)+CARRYIN)
      | PCIN-(C+B*(D+A))
      | PCIN-(C+B*(D+A)+CARRYIN)
      | PCIN-(C+B*(D-A))
      | PCIN-(C+B*(D-A)+CARRYIN)
      | PCIN-(C+B*A)
      | PCIN-(C+B*A+CARRYIN)
      | PCIN-(C+B*D)
      | PCIN-(C+B*D+CARRYIN)
      | PCIN-(C+C)
      | PCIN-(C+C+CARRYIN)
      | PCIN-(C+C+P)
      | PCIN-(C+C+P+CARRYIN)
      | PCIN-(C+CARRYIN)
      | PCIN-(C+D)
      | PCIN-(C+D*B)
      | PCIN-(C+D*B+CARRYIN)
      | PCIN-(C+D+CARRYIN)
      | PCIN-(C+P)
      | PCIN-(C+P+C)
      | PCIN-(C+P+C+CARRYIN)
      | PCIN-(C+P+CARRYIN)
      | PCIN-(C+P+P)
      | PCIN-(C+P+P+CARRYIN)
      | PCIN-(CARRYIN)
      | PCIN-(D)
      | PCIN-(D*B)
      | PCIN-(D*B+C)
      | PCIN-(D*B+C+CARRYIN)
      | PCIN-(D*B+CARRYIN)
      | PCIN-(D*B+P)
      | PCIN-(D*B+P+CARRYIN)
      | PCIN-(D+A)
      | PCIN-(D+A)*B
      | PCIN-(D+A)*B-C
      | PCIN-(D+A)*B-C-CARRYIN
      | PCIN-(D+A)*B-CARRYIN
      | PCIN-(D+A)*B-P
      | PCIN-(D+A)*B-P-CARRYIN
      | PCIN-(D+A)-C
      | PCIN-(D+A)-C-CARRYIN
      | PCIN-(D+A)-CARRYIN
      | PCIN-(D+A)-P
      | PCIN-(D+A)-P-CARRYIN
      | PCIN-(D+C)
      | PCIN-(D+C+CARRYIN)
      | PCIN-(D+CARRYIN)
      | PCIN-(D+P)
      | PCIN-(D+P+CARRYIN)
      | PCIN-(D-A)
      | PCIN-(D-A)*B
      | PCIN-(D-A)*B-C
      | PCIN-(D-A)*B-C-CARRYIN
      | PCIN-(D-A)*B-CARRYIN
      | PCIN-(D-A)*B-P
      | PCIN-(D-A)*B-P-CARRYIN
      | PCIN-(D-A)-C
      | PCIN-(D-A)-C-CARRYIN
      | PCIN-(D-A)-CARRYIN
      | PCIN-(D-A)-P
      | PCIN-(D-A)-P-CARRYIN
      | PCIN-(P)
      | PCIN-(P+(A+D))
      | PCIN-(P+(A+D)*B)
      | PCIN-(P+(A+D)*B+CARRYIN)
      | PCIN-(P+(A+D)+CARRYIN)
      | PCIN-(P+(D+A))
      | PCIN-(P+(D+A)*B)
      | PCIN-(P+(D+A)*B+CARRYIN)
      | PCIN-(P+(D+A)+CARRYIN)
      | PCIN-(P+(D-A))
      | PCIN-(P+(D-A)*B)
      | PCIN-(P+(D-A)*B+CARRYIN)
      | PCIN-(P+(D-A)+CARRYIN)
      | PCIN-(P+A)
      | PCIN-(P+A*B)
      | PCIN-(P+A*B+CARRYIN)
      | PCIN-(P+A+CARRYIN)
      | PCIN-(P+B*(A+D))
      | PCIN-(P+B*(A+D)+CARRYIN)
      | PCIN-(P+B*(D+A))
      | PCIN-(P+B*(D+A)+CARRYIN)
      | PCIN-(P+B*(D-A))
      | PCIN-(P+B*(D-A)+CARRYIN)
      | PCIN-(P+B*A)
      | PCIN-(P+B*A+CARRYIN)
      | PCIN-(P+B*D)
      | PCIN-(P+B*D+CARRYIN)
      | PCIN-(P+C)
      | PCIN-(P+C+C)
      | PCIN-(P+C+C+CARRYIN)
      | PCIN-(P+C+CARRYIN)
      | PCIN-(P+C+P)
      | PCIN-(P+C+P+CARRYIN)
      | PCIN-(P+CARRYIN)
      | PCIN-(P+D)
      | PCIN-(P+D*B)
      | PCIN-(P+D*B+CARRYIN)
      | PCIN-(P+D+CARRYIN)
      | PCIN-(P+P)
      | PCIN-(P+P+C)
      | PCIN-(P+P+C+CARRYIN)
      | PCIN-(P+P+CARRYIN)
      | PCIN-A
      | PCIN-A*B
      | PCIN-A*B-C
      | PCIN-A*B-C-CARRYIN
      | PCIN-A*B-CARRYIN
      | PCIN-A*B-P
      | PCIN-A*B-P-CARRYIN
      | PCIN-A-C
      | PCIN-A-C-CARRYIN
      | PCIN-A-CARRYIN
      | PCIN-A-P
      | PCIN-A-P-CARRYIN
      | PCIN-B*(A+D)
      | PCIN-B*(A+D)-C
      | PCIN-B*(A+D)-C-CARRYIN
      | PCIN-B*(A+D)-CARRYIN
      | PCIN-B*(A+D)-P
      | PCIN-B*(A+D)-P-CARRYIN
      | PCIN-B*(D+A)
      | PCIN-B*(D+A)-C
      | PCIN-B*(D+A)-C-CARRYIN
      | PCIN-B*(D+A)-CARRYIN
      | PCIN-B*(D+A)-P
      | PCIN-B*(D+A)-P-CARRYIN
      | PCIN-B*(D-A)
      | PCIN-B*(D-A)-C
      | PCIN-B*(D-A)-C-CARRYIN
      | PCIN-B*(D-A)-CARRYIN
      | PCIN-B*(D-A)-P
      | PCIN-B*(D-A)-P-CARRYIN
      | PCIN-B*A
      | PCIN-B*A-C
      | PCIN-B*A-C-CARRYIN
      | PCIN-B*A-CARRYIN
      | PCIN-B*A-P
      | PCIN-B*A-P-CARRYIN
      | PCIN-B*D
      | PCIN-B*D-C
      | PCIN-B*D-C-CARRYIN
      | PCIN-B*D-CARRYIN
      | PCIN-B*D-P
      | PCIN-B*D-P-CARRYIN
      | PCIN-C
      | PCIN-C-(A+D)
      | PCIN-C-(A+D)*B
      | PCIN-C-(A+D)*B-CARRYIN
      | PCIN-C-(A+D)-CARRYIN
      | PCIN-C-(D+A)
      | PCIN-C-(D+A)*B
      | PCIN-C-(D+A)*B-CARRYIN
      | PCIN-C-(D+A)-CARRYIN
      | PCIN-C-(D-A)
      | PCIN-C-(D-A)*B
      | PCIN-C-(D-A)*B-CARRYIN
      | PCIN-C-(D-A)-CARRYIN
      | PCIN-C-A
      | PCIN-C-A*B
      | PCIN-C-A*B-CARRYIN
      | PCIN-C-A-CARRYIN
      | PCIN-C-B*(A+D)
      | PCIN-C-B*(A+D)-CARRYIN
      | PCIN-C-B*(D+A)
      | PCIN-C-B*(D+A)-CARRYIN
      | PCIN-C-B*(D-A)
      | PCIN-C-B*(D-A)-CARRYIN
      | PCIN-C-B*A
      | PCIN-C-B*A-CARRYIN
      | PCIN-C-B*D
      | PCIN-C-B*D-CARRYIN
      | PCIN-C-C
      | PCIN-C-C-CARRYIN
      | PCIN-C-C-P
      | PCIN-C-C-P-CARRYIN
      | PCIN-C-CARRYIN
      | PCIN-C-D
      | PCIN-C-D*B
      | PCIN-C-D*B-CARRYIN
      | PCIN-C-D-CARRYIN
      | PCIN-C-P
      | PCIN-C-P-C
      | PCIN-C-P-C-CARRYIN
      | PCIN-C-P-CARRYIN
      | PCIN-C-P-P
      | PCIN-C-P-P-CARRYIN
      | PCIN-CARRYIN
      | PCIN-D
      | PCIN-D*B
      | PCIN-D*B-C
      | PCIN-D*B-C-CARRYIN
      | PCIN-D*B-CARRYIN
      | PCIN-D*B-P
      | PCIN-D*B-P-CARRYIN
      | PCIN-D-C
      | PCIN-D-C-CARRYIN
      | PCIN-D-CARRYIN
      | PCIN-D-P
      | PCIN-D-P-CARRYIN
      | PCIN-P
      | PCIN-P-(A+D)
      | PCIN-P-(A+D)*B
      | PCIN-P-(A+D)*B-CARRYIN
      | PCIN-P-(A+D)-CARRYIN
      | PCIN-P-(D+A)
      | PCIN-P-(D+A)*B
      | PCIN-P-(D+A)*B-CARRYIN
      | PCIN-P-(D+A)-CARRYIN
      | PCIN-P-(D-A)
      | PCIN-P-(D-A)*B
      | PCIN-P-(D-A)*B-CARRYIN
      | PCIN-P-(D-A)-CARRYIN
      | PCIN-P-A
      | PCIN-P-A*B
      | PCIN-P-A*B-CARRYIN
      | PCIN-P-A-CARRYIN
      | PCIN-P-B*(A+D)
      | PCIN-P-B*(A+D)-CARRYIN
      | PCIN-P-B*(D+A)
      | PCIN-P-B*(D+A)-CARRYIN
      | PCIN-P-B*(D-A)
      | PCIN-P-B*(D-A)-CARRYIN
      | PCIN-P-B*A
      | PCIN-P-B*A-CARRYIN
      | PCIN-P-B*D
      | PCIN-P-B*D-CARRYIN
      | PCIN-P-C
      | PCIN-P-C-C
      | PCIN-P-C-C-CARRYIN
      | PCIN-P-C-CARRYIN
      | PCIN-P-C-P
      | PCIN-P-C-P-CARRYIN
      | PCIN-P-CARRYIN
      | PCIN-P-D
      | PCIN-P-D*B
      | PCIN-P-D*B-CARRYIN
      | PCIN-P-D-CARRYIN
      | PCIN-P-P
      | PCIN-P-P-C
      | PCIN-P-P-C-CARRYIN
      | PCIN-P-P-CARRYIN
      | PCIN>>17
      | PCIN>>17+(A+D)
      | PCIN>>17+(A+D)*B
      | PCIN>>17+(A+D)*B+C
      | PCIN>>17+(A+D)*B+C+CARRYIN
      | PCIN>>17+(A+D)*B+CARRYIN
      | PCIN>>17+(A+D)*B+P
      | PCIN>>17+(A+D)*B+P+CARRYIN
      | PCIN>>17+(A+D)+C
      | PCIN>>17+(A+D)+C+CARRYIN
      | PCIN>>17+(A+D)+CARRYIN
      | PCIN>>17+(A+D)+P
      | PCIN>>17+(A+D)+P+CARRYIN
      | PCIN>>17+(D+A)
      | PCIN>>17+(D+A)*B
      | PCIN>>17+(D+A)*B+C
      | PCIN>>17+(D+A)*B+C+CARRYIN
      | PCIN>>17+(D+A)*B+CARRYIN
      | PCIN>>17+(D+A)*B+P
      | PCIN>>17+(D+A)*B+P+CARRYIN
      | PCIN>>17+(D+A)+C
      | PCIN>>17+(D+A)+C+CARRYIN
      | PCIN>>17+(D+A)+CARRYIN
      | PCIN>>17+(D+A)+P
      | PCIN>>17+(D+A)+P+CARRYIN
      | PCIN>>17+(D-A)
      | PCIN>>17+(D-A)*B
      | PCIN>>17+(D-A)*B+C
      | PCIN>>17+(D-A)*B+C+CARRYIN
      | PCIN>>17+(D-A)*B+CARRYIN
      | PCIN>>17+(D-A)*B+P
      | PCIN>>17+(D-A)*B+P+CARRYIN
      | PCIN>>17+(D-A)+C
      | PCIN>>17+(D-A)+C+CARRYIN
      | PCIN>>17+(D-A)+CARRYIN
      | PCIN>>17+(D-A)+P
      | PCIN>>17+(D-A)+P+CARRYIN
      | PCIN>>17+A
      | PCIN>>17+A*B
      | PCIN>>17+A*B+C
      | PCIN>>17+A*B+C+CARRYIN
      | PCIN>>17+A*B+CARRYIN
      | PCIN>>17+A*B+P
      | PCIN>>17+A*B+P+CARRYIN
      | PCIN>>17+A+C
      | PCIN>>17+A+C+CARRYIN
      | PCIN>>17+A+CARRYIN
      | PCIN>>17+A+P
      | PCIN>>17+A+P+CARRYIN
      | PCIN>>17+B*(A+D)
      | PCIN>>17+B*(A+D)+C
      | PCIN>>17+B*(A+D)+C+CARRYIN
      | PCIN>>17+B*(A+D)+CARRYIN
      | PCIN>>17+B*(A+D)+P
      | PCIN>>17+B*(A+D)+P+CARRYIN
      | PCIN>>17+B*(D+A)
      | PCIN>>17+B*(D+A)+C
      | PCIN>>17+B*(D+A)+C+CARRYIN
      | PCIN>>17+B*(D+A)+CARRYIN
      | PCIN>>17+B*(D+A)+P
      | PCIN>>17+B*(D+A)+P+CARRYIN
      | PCIN>>17+B*(D-A)
      | PCIN>>17+B*(D-A)+C
      | PCIN>>17+B*(D-A)+C+CARRYIN
      | PCIN>>17+B*(D-A)+CARRYIN
      | PCIN>>17+B*(D-A)+P
      | PCIN>>17+B*(D-A)+P+CARRYIN
      | PCIN>>17+B*A
      | PCIN>>17+B*A+C
      | PCIN>>17+B*A+C+CARRYIN
      | PCIN>>17+B*A+CARRYIN
      | PCIN>>17+B*A+P
      | PCIN>>17+B*A+P+CARRYIN
      | PCIN>>17+B*D
      | PCIN>>17+B*D+C
      | PCIN>>17+B*D+C+CARRYIN
      | PCIN>>17+B*D+CARRYIN
      | PCIN>>17+B*D+P
      | PCIN>>17+B*D+P+CARRYIN
      | PCIN>>17+C
      | PCIN>>17+C+(A+D)
      | PCIN>>17+C+(A+D)*B
      | PCIN>>17+C+(A+D)*B+CARRYIN
      | PCIN>>17+C+(A+D)+CARRYIN
      | PCIN>>17+C+(D+A)
      | PCIN>>17+C+(D+A)*B
      | PCIN>>17+C+(D+A)*B+CARRYIN
      | PCIN>>17+C+(D+A)+CARRYIN
      | PCIN>>17+C+(D-A)
      | PCIN>>17+C+(D-A)*B
      | PCIN>>17+C+(D-A)*B+CARRYIN
      | PCIN>>17+C+(D-A)+CARRYIN
      | PCIN>>17+C+A
      | PCIN>>17+C+A*B
      | PCIN>>17+C+A*B+CARRYIN
      | PCIN>>17+C+A+CARRYIN
      | PCIN>>17+C+B*(A+D)
      | PCIN>>17+C+B*(A+D)+CARRYIN
      | PCIN>>17+C+B*(D+A)
      | PCIN>>17+C+B*(D+A)+CARRYIN
      | PCIN>>17+C+B*(D-A)
      | PCIN>>17+C+B*(D-A)+CARRYIN
      | PCIN>>17+C+B*A
      | PCIN>>17+C+B*A+CARRYIN
      | PCIN>>17+C+B*D
      | PCIN>>17+C+B*D+CARRYIN
      | PCIN>>17+C+C
      | PCIN>>17+C+C+CARRYIN
      | PCIN>>17+C+C+P
      | PCIN>>17+C+C+P+CARRYIN
      | PCIN>>17+C+CARRYIN
      | PCIN>>17+C+D
      | PCIN>>17+C+D*B
      | PCIN>>17+C+D*B+CARRYIN
      | PCIN>>17+C+D+CARRYIN
      | PCIN>>17+C+P
      | PCIN>>17+C+P+C
      | PCIN>>17+C+P+C+CARRYIN
      | PCIN>>17+C+P+CARRYIN
      | PCIN>>17+C+P+P
      | PCIN>>17+C+P+P+CARRYIN
      | PCIN>>17+CARRYIN
      | PCIN>>17+D
      | PCIN>>17+D*B
      | PCIN>>17+D*B+C
      | PCIN>>17+D*B+C+CARRYIN
      | PCIN>>17+D*B+CARRYIN
      | PCIN>>17+D*B+P
      | PCIN>>17+D*B+P+CARRYIN
      | PCIN>>17+D+C
      | PCIN>>17+D+C+CARRYIN
      | PCIN>>17+D+CARRYIN
      | PCIN>>17+D+P
      | PCIN>>17+D+P+CARRYIN
      | PCIN>>17+P
      | PCIN>>17+P+(A+D)
      | PCIN>>17+P+(A+D)*B
      | PCIN>>17+P+(A+D)*B+CARRYIN
      | PCIN>>17+P+(A+D)+CARRYIN
      | PCIN>>17+P+(D+A)
      | PCIN>>17+P+(D+A)*B
      | PCIN>>17+P+(D+A)*B+CARRYIN
      | PCIN>>17+P+(D+A)+CARRYIN
      | PCIN>>17+P+(D-A)
      | PCIN>>17+P+(D-A)*B
      | PCIN>>17+P+(D-A)*B+CARRYIN
      | PCIN>>17+P+(D-A)+CARRYIN
      | PCIN>>17+P+A
      | PCIN>>17+P+A*B
      | PCIN>>17+P+A*B+CARRYIN
      | PCIN>>17+P+A+CARRYIN
      | PCIN>>17+P+B*(A+D)
      | PCIN>>17+P+B*(A+D)+CARRYIN
      | PCIN>>17+P+B*(D+A)
      | PCIN>>17+P+B*(D+A)+CARRYIN
      | PCIN>>17+P+B*(D-A)
      | PCIN>>17+P+B*(D-A)+CARRYIN
      | PCIN>>17+P+B*A
      | PCIN>>17+P+B*A+CARRYIN
      | PCIN>>17+P+B*D
      | PCIN>>17+P+B*D+CARRYIN
      | PCIN>>17+P+C
      | PCIN>>17+P+C+C
      | PCIN>>17+P+C+C+CARRYIN
      | PCIN>>17+P+C+CARRYIN
      | PCIN>>17+P+C+P
      | PCIN>>17+P+C+P+CARRYIN
      | PCIN>>17+P+CARRYIN
      | PCIN>>17+P+D
      | PCIN>>17+P+D*B
      | PCIN>>17+P+D*B+CARRYIN
      | PCIN>>17+P+D+CARRYIN
      | PCIN>>17+P+P
      | PCIN>>17+P+P+C
      | PCIN>>17+P+P+C+CARRYIN
      | PCIN>>17+P+P+CARRYIN
      | PCIN>>17-((A+D))
      | PCIN>>17-((A+D)*B)
      | PCIN>>17-((A+D)*B+C)
      | PCIN>>17-((A+D)*B+C+CARRYIN)
      | PCIN>>17-((A+D)*B+CARRYIN)
      | PCIN>>17-((A+D)*B+P)
      | PCIN>>17-((A+D)*B+P+CARRYIN)
      | PCIN>>17-((A+D)+C)
      | PCIN>>17-((A+D)+C+CARRYIN)
      | PCIN>>17-((A+D)+CARRYIN)
      | PCIN>>17-((A+D)+P)
      | PCIN>>17-((A+D)+P+CARRYIN)
      | PCIN>>17-((D+A))
      | PCIN>>17-((D+A)*B)
      | PCIN>>17-((D+A)*B+C)
      | PCIN>>17-((D+A)*B+C+CARRYIN)
      | PCIN>>17-((D+A)*B+CARRYIN)
      | PCIN>>17-((D+A)*B+P)
      | PCIN>>17-((D+A)*B+P+CARRYIN)
      | PCIN>>17-((D+A)+C)
      | PCIN>>17-((D+A)+C+CARRYIN)
      | PCIN>>17-((D+A)+CARRYIN)
      | PCIN>>17-((D+A)+P)
      | PCIN>>17-((D+A)+P+CARRYIN)
      | PCIN>>17-((D-A))
      | PCIN>>17-((D-A)*B)
      | PCIN>>17-((D-A)*B+C)
      | PCIN>>17-((D-A)*B+C+CARRYIN)
      | PCIN>>17-((D-A)*B+CARRYIN)
      | PCIN>>17-((D-A)*B+P)
      | PCIN>>17-((D-A)*B+P+CARRYIN)
      | PCIN>>17-((D-A)+C)
      | PCIN>>17-((D-A)+C+CARRYIN)
      | PCIN>>17-((D-A)+CARRYIN)
      | PCIN>>17-((D-A)+P)
      | PCIN>>17-((D-A)+P+CARRYIN)
      | PCIN>>17-(A)
      | PCIN>>17-(A*B)
      | PCIN>>17-(A*B+C)
      | PCIN>>17-(A*B+C+CARRYIN)
      | PCIN>>17-(A*B+CARRYIN)
      | PCIN>>17-(A*B+P)
      | PCIN>>17-(A*B+P+CARRYIN)
      | PCIN>>17-(A+C)
      | PCIN>>17-(A+C+CARRYIN)
      | PCIN>>17-(A+CARRYIN)
      | PCIN>>17-(A+D)
      | PCIN>>17-(A+D)*B
      | PCIN>>17-(A+D)*B-C
      | PCIN>>17-(A+D)*B-C-CARRYIN
      | PCIN>>17-(A+D)*B-CARRYIN
      | PCIN>>17-(A+D)*B-P
      | PCIN>>17-(A+D)*B-P-CARRYIN
      | PCIN>>17-(A+D)-C
      | PCIN>>17-(A+D)-C-CARRYIN
      | PCIN>>17-(A+D)-CARRYIN
      | PCIN>>17-(A+D)-P
      | PCIN>>17-(A+D)-P-CARRYIN
      | PCIN>>17-(A+P)
      | PCIN>>17-(A+P+CARRYIN)
      | PCIN>>17-(B*(A+D))
      | PCIN>>17-(B*(A+D)+C)
      | PCIN>>17-(B*(A+D)+C+CARRYIN)
      | PCIN>>17-(B*(A+D)+CARRYIN)
      | PCIN>>17-(B*(A+D)+P)
      | PCIN>>17-(B*(A+D)+P+CARRYIN)
      | PCIN>>17-(B*(D+A))
      | PCIN>>17-(B*(D+A)+C)
      | PCIN>>17-(B*(D+A)+C+CARRYIN)
      | PCIN>>17-(B*(D+A)+CARRYIN)
      | PCIN>>17-(B*(D+A)+P)
      | PCIN>>17-(B*(D+A)+P+CARRYIN)
      | PCIN>>17-(B*(D-A))
      | PCIN>>17-(B*(D-A)+C)
      | PCIN>>17-(B*(D-A)+C+CARRYIN)
      | PCIN>>17-(B*(D-A)+CARRYIN)
      | PCIN>>17-(B*(D-A)+P)
      | PCIN>>17-(B*(D-A)+P+CARRYIN)
      | PCIN>>17-(B*A)
      | PCIN>>17-(B*A+C)
      | PCIN>>17-(B*A+C+CARRYIN)
      | PCIN>>17-(B*A+CARRYIN)
      | PCIN>>17-(B*A+P)
      | PCIN>>17-(B*A+P+CARRYIN)
      | PCIN>>17-(B*D)
      | PCIN>>17-(B*D+C)
      | PCIN>>17-(B*D+C+CARRYIN)
      | PCIN>>17-(B*D+CARRYIN)
      | PCIN>>17-(B*D+P)
      | PCIN>>17-(B*D+P+CARRYIN)
      | PCIN>>17-(C)
      | PCIN>>17-(C+(A+D))
      | PCIN>>17-(C+(A+D)*B)
      | PCIN>>17-(C+(A+D)*B+CARRYIN)
      | PCIN>>17-(C+(A+D)+CARRYIN)
      | PCIN>>17-(C+(D+A))
      | PCIN>>17-(C+(D+A)*B)
      | PCIN>>17-(C+(D+A)*B+CARRYIN)
      | PCIN>>17-(C+(D+A)+CARRYIN)
      | PCIN>>17-(C+(D-A))
      | PCIN>>17-(C+(D-A)*B)
      | PCIN>>17-(C+(D-A)*B+CARRYIN)
      | PCIN>>17-(C+(D-A)+CARRYIN)
      | PCIN>>17-(C+A)
      | PCIN>>17-(C+A*B)
      | PCIN>>17-(C+A*B+CARRYIN)
      | PCIN>>17-(C+A+CARRYIN)
      | PCIN>>17-(C+B*(A+D))
      | PCIN>>17-(C+B*(A+D)+CARRYIN)
      | PCIN>>17-(C+B*(D+A))
      | PCIN>>17-(C+B*(D+A)+CARRYIN)
      | PCIN>>17-(C+B*(D-A))
      | PCIN>>17-(C+B*(D-A)+CARRYIN)
      | PCIN>>17-(C+B*A)
      | PCIN>>17-(C+B*A+CARRYIN)
      | PCIN>>17-(C+B*D)
      | PCIN>>17-(C+B*D+CARRYIN)
      | PCIN>>17-(C+C)
      | PCIN>>17-(C+C+CARRYIN)
      | PCIN>>17-(C+C+P)
      | PCIN>>17-(C+C+P+CARRYIN)
      | PCIN>>17-(C+CARRYIN)
      | PCIN>>17-(C+D)
      | PCIN>>17-(C+D*B)
      | PCIN>>17-(C+D*B+CARRYIN)
      | PCIN>>17-(C+D+CARRYIN)
      | PCIN>>17-(C+P)
      | PCIN>>17-(C+P+C)
      | PCIN>>17-(C+P+C+CARRYIN)
      | PCIN>>17-(C+P+CARRYIN)
      | PCIN>>17-(C+P+P)
      | PCIN>>17-(C+P+P+CARRYIN)
      | PCIN>>17-(CARRYIN)
      | PCIN>>17-(D)
      | PCIN>>17-(D*B)
      | PCIN>>17-(D*B+C)
      | PCIN>>17-(D*B+C+CARRYIN)
      | PCIN>>17-(D*B+CARRYIN)
      | PCIN>>17-(D*B+P)
      | PCIN>>17-(D*B+P+CARRYIN)
      | PCIN>>17-(D+A)
      | PCIN>>17-(D+A)*B
      | PCIN>>17-(D+A)*B-C
      | PCIN>>17-(D+A)*B-C-CARRYIN
      | PCIN>>17-(D+A)*B-CARRYIN
      | PCIN>>17-(D+A)*B-P
      | PCIN>>17-(D+A)*B-P-CARRYIN
      | PCIN>>17-(D+A)-C
      | PCIN>>17-(D+A)-C-CARRYIN
      | PCIN>>17-(D+A)-CARRYIN
      | PCIN>>17-(D+A)-P
      | PCIN>>17-(D+A)-P-CARRYIN
      | PCIN>>17-(D+C)
      | PCIN>>17-(D+C+CARRYIN)
      | PCIN>>17-(D+CARRYIN)
      | PCIN>>17-(D+P)
      | PCIN>>17-(D+P+CARRYIN)
      | PCIN>>17-(D-A)
      | PCIN>>17-(D-A)*B
      | PCIN>>17-(D-A)*B-C
      | PCIN>>17-(D-A)*B-C-CARRYIN
      | PCIN>>17-(D-A)*B-CARRYIN
      | PCIN>>17-(D-A)*B-P
      | PCIN>>17-(D-A)*B-P-CARRYIN
      | PCIN>>17-(D-A)-C
      | PCIN>>17-(D-A)-C-CARRYIN
      | PCIN>>17-(D-A)-CARRYIN
      | PCIN>>17-(D-A)-P
      | PCIN>>17-(D-A)-P-CARRYIN
      | PCIN>>17-(P)
      | PCIN>>17-(P+(A+D))
      | PCIN>>17-(P+(A+D)*B)
      | PCIN>>17-(P+(A+D)*B+CARRYIN)
      | PCIN>>17-(P+(A+D)+CARRYIN)
      | PCIN>>17-(P+(D+A))
      | PCIN>>17-(P+(D+A)*B)
      | PCIN>>17-(P+(D+A)*B+CARRYIN)
      | PCIN>>17-(P+(D+A)+CARRYIN)
      | PCIN>>17-(P+(D-A))
      | PCIN>>17-(P+(D-A)*B)
      | PCIN>>17-(P+(D-A)*B+CARRYIN)
      | PCIN>>17-(P+(D-A)+CARRYIN)
      | PCIN>>17-(P+A)
      | PCIN>>17-(P+A*B)
      | PCIN>>17-(P+A*B+CARRYIN)
      | PCIN>>17-(P+A+CARRYIN)
      | PCIN>>17-(P+B*(A+D))
      | PCIN>>17-(P+B*(A+D)+CARRYIN)
      | PCIN>>17-(P+B*(D+A))
      | PCIN>>17-(P+B*(D+A)+CARRYIN)
      | PCIN>>17-(P+B*(D-A))
      | PCIN>>17-(P+B*(D-A)+CARRYIN)
      | PCIN>>17-(P+B*A)
      | PCIN>>17-(P+B*A+CARRYIN)
      | PCIN>>17-(P+B*D)
      | PCIN>>17-(P+B*D+CARRYIN)
      | PCIN>>17-(P+C)
      | PCIN>>17-(P+C+C)
      | PCIN>>17-(P+C+C+CARRYIN)
      | PCIN>>17-(P+C+CARRYIN)
      | PCIN>>17-(P+C+P)
      | PCIN>>17-(P+C+P+CARRYIN)
      | PCIN>>17-(P+CARRYIN)
      | PCIN>>17-(P+D)
      | PCIN>>17-(P+D*B)
      | PCIN>>17-(P+D*B+CARRYIN)
      | PCIN>>17-(P+D+CARRYIN)
      | PCIN>>17-(P+P)
      | PCIN>>17-(P+P+C)
      | PCIN>>17-(P+P+C+CARRYIN)
      | PCIN>>17-(P+P+CARRYIN)
      | PCIN>>17-A
      | PCIN>>17-A*B
      | PCIN>>17-A*B-C
      | PCIN>>17-A*B-C-CARRYIN
      | PCIN>>17-A*B-CARRYIN
      | PCIN>>17-A*B-P
      | PCIN>>17-A*B-P-CARRYIN
      | PCIN>>17-A-C
      | PCIN>>17-A-C-CARRYIN
      | PCIN>>17-A-CARRYIN
      | PCIN>>17-A-P
      | PCIN>>17-A-P-CARRYIN
      | PCIN>>17-B*(A+D)
      | PCIN>>17-B*(A+D)-C
      | PCIN>>17-B*(A+D)-C-CARRYIN
      | PCIN>>17-B*(A+D)-CARRYIN
      | PCIN>>17-B*(A+D)-P
      | PCIN>>17-B*(A+D)-P-CARRYIN
      | PCIN>>17-B*(D+A)
      | PCIN>>17-B*(D+A)-C
      | PCIN>>17-B*(D+A)-C-CARRYIN
      | PCIN>>17-B*(D+A)-CARRYIN
      | PCIN>>17-B*(D+A)-P
      | PCIN>>17-B*(D+A)-P-CARRYIN
      | PCIN>>17-B*(D-A)
      | PCIN>>17-B*(D-A)-C
      | PCIN>>17-B*(D-A)-C-CARRYIN
      | PCIN>>17-B*(D-A)-CARRYIN
      | PCIN>>17-B*(D-A)-P
      | PCIN>>17-B*(D-A)-P-CARRYIN
      | PCIN>>17-B*A
      | PCIN>>17-B*A-C
      | PCIN>>17-B*A-C-CARRYIN
      | PCIN>>17-B*A-CARRYIN
      | PCIN>>17-B*A-P
      | PCIN>>17-B*A-P-CARRYIN
      | PCIN>>17-B*D
      | PCIN>>17-B*D-C
      | PCIN>>17-B*D-C-CARRYIN
      | PCIN>>17-B*D-CARRYIN
      | PCIN>>17-B*D-P
      | PCIN>>17-B*D-P-CARRYIN
      | PCIN>>17-C
      | PCIN>>17-C-(A+D)
      | PCIN>>17-C-(A+D)*B
      | PCIN>>17-C-(A+D)*B-CARRYIN
      | PCIN>>17-C-(A+D)-CARRYIN
      | PCIN>>17-C-(D+A)
      | PCIN>>17-C-(D+A)*B
      | PCIN>>17-C-(D+A)*B-CARRYIN
      | PCIN>>17-C-(D+A)-CARRYIN
      | PCIN>>17-C-(D-A)
      | PCIN>>17-C-(D-A)*B
      | PCIN>>17-C-(D-A)*B-CARRYIN
      | PCIN>>17-C-(D-A)-CARRYIN
      | PCIN>>17-C-A
      | PCIN>>17-C-A*B
      | PCIN>>17-C-A*B-CARRYIN
      | PCIN>>17-C-A-CARRYIN
      | PCIN>>17-C-B*(A+D)
      | PCIN>>17-C-B*(A+D)-CARRYIN
      | PCIN>>17-C-B*(D+A)
      | PCIN>>17-C-B*(D+A)-CARRYIN
      | PCIN>>17-C-B*(D-A)
      | PCIN>>17-C-B*(D-A)-CARRYIN
      | PCIN>>17-C-B*A
      | PCIN>>17-C-B*A-CARRYIN
      | PCIN>>17-C-B*D
      | PCIN>>17-C-B*D-CARRYIN
      | PCIN>>17-C-C
      | PCIN>>17-C-C-CARRYIN
      | PCIN>>17-C-C-P
      | PCIN>>17-C-C-P-CARRYIN
      | PCIN>>17-C-CARRYIN
      | PCIN>>17-C-D
      | PCIN>>17-C-D*B
      | PCIN>>17-C-D*B-CARRYIN
      | PCIN>>17-C-D-CARRYIN
      | PCIN>>17-C-P
      | PCIN>>17-C-P-C
      | PCIN>>17-C-P-C-CARRYIN
      | PCIN>>17-C-P-CARRYIN
      | PCIN>>17-C-P-P
      | PCIN>>17-C-P-P-CARRYIN
      | PCIN>>17-CARRYIN
      | PCIN>>17-D
      | PCIN>>17-D*B
      | PCIN>>17-D*B-C
      | PCIN>>17-D*B-C-CARRYIN
      | PCIN>>17-D*B-CARRYIN
      | PCIN>>17-D*B-P
      | PCIN>>17-D*B-P-CARRYIN
      | PCIN>>17-D-C
      | PCIN>>17-D-C-CARRYIN
      | PCIN>>17-D-CARRYIN
      | PCIN>>17-D-P
      | PCIN>>17-D-P-CARRYIN
      | PCIN>>17-P
      | PCIN>>17-P-(A+D)
      | PCIN>>17-P-(A+D)*B
      | PCIN>>17-P-(A+D)*B-CARRYIN
      | PCIN>>17-P-(A+D)-CARRYIN
      | PCIN>>17-P-(D+A)
      | PCIN>>17-P-(D+A)*B
      | PCIN>>17-P-(D+A)*B-CARRYIN
      | PCIN>>17-P-(D+A)-CARRYIN
      | PCIN>>17-P-(D-A)
      | PCIN>>17-P-(D-A)*B
      | PCIN>>17-P-(D-A)*B-CARRYIN
      | PCIN>>17-P-(D-A)-CARRYIN
      | PCIN>>17-P-A
      | PCIN>>17-P-A*B
      | PCIN>>17-P-A*B-CARRYIN
      | PCIN>>17-P-A-CARRYIN
      | PCIN>>17-P-B*(A+D)
      | PCIN>>17-P-B*(A+D)-CARRYIN
      | PCIN>>17-P-B*(D+A)
      | PCIN>>17-P-B*(D+A)-CARRYIN
      | PCIN>>17-P-B*(D-A)
      | PCIN>>17-P-B*(D-A)-CARRYIN
      | PCIN>>17-P-B*A
      | PCIN>>17-P-B*A-CARRYIN
      | PCIN>>17-P-B*D
      | PCIN>>17-P-B*D-CARRYIN
      | PCIN>>17-P-C
      | PCIN>>17-P-C-C
      | PCIN>>17-P-C-C-CARRYIN
      | PCIN>>17-P-C-CARRYIN
      | PCIN>>17-P-C-P
      | PCIN>>17-P-C-P-CARRYIN
      | PCIN>>17-P-CARRYIN
      | PCIN>>17-P-D
      | PCIN>>17-P-D*B
      | PCIN>>17-P-D*B-CARRYIN
      | PCIN>>17-P-D-CARRYIN
      | PCIN>>17-P-P
      | PCIN>>17-P-P-C
      | PCIN>>17-P-P-C-CARRYIN
      | PCIN>>17-P-P-CARRYIN
      | RNDMACC((A+D)*B+C+P)
      | RNDMACC((A+D)*B+P)
      | RNDMACC((A+D)*B+P+C)
      | RNDMACC((A+D)*B+P+P)
      | RNDMACC((D+A)*B+C+P)
      | RNDMACC((D+A)*B+P)
      | RNDMACC((D+A)*B+P+C)
      | RNDMACC((D+A)*B+P+P)
      | RNDMACC((D-A)*B+C+P)
      | RNDMACC((D-A)*B+P)
      | RNDMACC((D-A)*B+P+C)
      | RNDMACC((D-A)*B+P+P)
      | RNDMACC(A*B+C+P)
      | RNDMACC(A*B+P)
      | RNDMACC(A*B+P+C)
      | RNDMACC(A*B+P+P)
      | RNDMACC(B*(A+D)+C+P)
      | RNDMACC(B*(A+D)+P)
      | RNDMACC(B*(A+D)+P+C)
      | RNDMACC(B*(A+D)+P+P)
      | RNDMACC(B*(D+A)+C+P)
      | RNDMACC(B*(D+A)+P)
      | RNDMACC(B*(D+A)+P+C)
      | RNDMACC(B*(D+A)+P+P)
      | RNDMACC(B*(D-A)+C+P)
      | RNDMACC(B*(D-A)+P)
      | RNDMACC(B*(D-A)+P+C)
      | RNDMACC(B*(D-A)+P+P)
      | RNDMACC(B*A+C+P)
      | RNDMACC(B*A+P)
      | RNDMACC(B*A+P+C)
      | RNDMACC(B*A+P+P)
      | RNDMACC(B*D+C+P)
      | RNDMACC(B*D+P)
      | RNDMACC(B*D+P+C)
      | RNDMACC(B*D+P+P)
      | RNDMACC(D*B+C+P)
      | RNDMACC(D*B+P)
      | RNDMACC(D*B+P+C)
      | RNDMACC(D*B+P+P)
      | RNDSIMPLE((A+D))
      | RNDSIMPLE((A+D)*B)
      | RNDSIMPLE((A+D)*B+C)
      | RNDSIMPLE((A+D)*B+C+CARRYIN)
      | RNDSIMPLE((A+D)*B+CARRYIN)
      | RNDSIMPLE((A+D)*B+P)
      | RNDSIMPLE((A+D)*B+P+CARRYIN)
      | RNDSIMPLE((A+D)*B+P>>17)
      | RNDSIMPLE((A+D)*B+P>>17+CARRYIN)
      | RNDSIMPLE((A+D)*B+PCIN)
      | RNDSIMPLE((A+D)*B+PCIN+CARRYIN)
      | RNDSIMPLE((A+D)*B+PCIN>>17)
      | RNDSIMPLE((A+D)*B+PCIN>>17+CARRYIN)
      | RNDSIMPLE((A+D)+C)
      | RNDSIMPLE((A+D)+C+CARRYIN)
      | RNDSIMPLE((A+D)+CARRYIN)
      | RNDSIMPLE((A+D)+P)
      | RNDSIMPLE((A+D)+P+CARRYIN)
      | RNDSIMPLE((A+D)+P>>17)
      | RNDSIMPLE((A+D)+P>>17+CARRYIN)
      | RNDSIMPLE((A+D)+PCIN)
      | RNDSIMPLE((A+D)+PCIN+CARRYIN)
      | RNDSIMPLE((A+D)+PCIN>>17)
      | RNDSIMPLE((A+D)+PCIN>>17+CARRYIN)
      | RNDSIMPLE((D+A))
      | RNDSIMPLE((D+A)*B)
      | RNDSIMPLE((D+A)*B+C)
      | RNDSIMPLE((D+A)*B+C+CARRYIN)
      | RNDSIMPLE((D+A)*B+CARRYIN)
      | RNDSIMPLE((D+A)*B+P)
      | RNDSIMPLE((D+A)*B+P+CARRYIN)
      | RNDSIMPLE((D+A)*B+P>>17)
      | RNDSIMPLE((D+A)*B+P>>17+CARRYIN)
      | RNDSIMPLE((D+A)*B+PCIN)
      | RNDSIMPLE((D+A)*B+PCIN+CARRYIN)
      | RNDSIMPLE((D+A)*B+PCIN>>17)
      | RNDSIMPLE((D+A)*B+PCIN>>17+CARRYIN)
      | RNDSIMPLE((D+A)+C)
      | RNDSIMPLE((D+A)+C+CARRYIN)
      | RNDSIMPLE((D+A)+CARRYIN)
      | RNDSIMPLE((D+A)+P)
      | RNDSIMPLE((D+A)+P+CARRYIN)
      | RNDSIMPLE((D+A)+P>>17)
      | RNDSIMPLE((D+A)+P>>17+CARRYIN)
      | RNDSIMPLE((D+A)+PCIN)
      | RNDSIMPLE((D+A)+PCIN+CARRYIN)
      | RNDSIMPLE((D+A)+PCIN>>17)
      | RNDSIMPLE((D+A)+PCIN>>17+CARRYIN)
      | RNDSIMPLE((D-A))
      | RNDSIMPLE((D-A)*B)
      | RNDSIMPLE((D-A)*B+C)
      | RNDSIMPLE((D-A)*B+C+CARRYIN)
      | RNDSIMPLE((D-A)*B+CARRYIN)
      | RNDSIMPLE((D-A)*B+P)
      | RNDSIMPLE((D-A)*B+P+CARRYIN)
      | RNDSIMPLE((D-A)*B+P>>17)
      | RNDSIMPLE((D-A)*B+P>>17+CARRYIN)
      | RNDSIMPLE((D-A)*B+PCIN)
      | RNDSIMPLE((D-A)*B+PCIN+CARRYIN)
      | RNDSIMPLE((D-A)*B+PCIN>>17)
      | RNDSIMPLE((D-A)*B+PCIN>>17+CARRYIN)
      | RNDSIMPLE((D-A)+C)
      | RNDSIMPLE((D-A)+C+CARRYIN)
      | RNDSIMPLE((D-A)+CARRYIN)
      | RNDSIMPLE((D-A)+P)
      | RNDSIMPLE((D-A)+P+CARRYIN)
      | RNDSIMPLE((D-A)+P>>17)
      | RNDSIMPLE((D-A)+P>>17+CARRYIN)
      | RNDSIMPLE((D-A)+PCIN)
      | RNDSIMPLE((D-A)+PCIN+CARRYIN)
      | RNDSIMPLE((D-A)+PCIN>>17)
      | RNDSIMPLE((D-A)+PCIN>>17+CARRYIN)
      | RNDSIMPLE(A)
      | RNDSIMPLE(A*B)
      | RNDSIMPLE(A*B+C)
      | RNDSIMPLE(A*B+C+CARRYIN)
      | RNDSIMPLE(A*B+CARRYIN)
      | RNDSIMPLE(A*B+P)
      | RNDSIMPLE(A*B+P+CARRYIN)
      | RNDSIMPLE(A*B+P>>17)
      | RNDSIMPLE(A*B+P>>17+CARRYIN)
      | RNDSIMPLE(A*B+PCIN)
      | RNDSIMPLE(A*B+PCIN+CARRYIN)
      | RNDSIMPLE(A*B+PCIN>>17)
      | RNDSIMPLE(A*B+PCIN>>17+CARRYIN)
      | RNDSIMPLE(A+C)
      | RNDSIMPLE(A+C+CARRYIN)
      | RNDSIMPLE(A+CARRYIN)
      | RNDSIMPLE(A+P)
      | RNDSIMPLE(A+P+CARRYIN)
      | RNDSIMPLE(A+P>>17)
      | RNDSIMPLE(A+P>>17+CARRYIN)
      | RNDSIMPLE(A+PCIN)
      | RNDSIMPLE(A+PCIN+CARRYIN)
      | RNDSIMPLE(A+PCIN>>17)
      | RNDSIMPLE(A+PCIN>>17+CARRYIN)
      | RNDSIMPLE(B*(A+D))
      | RNDSIMPLE(B*(A+D)+C)
      | RNDSIMPLE(B*(A+D)+C+CARRYIN)
      | RNDSIMPLE(B*(A+D)+CARRYIN)
      | RNDSIMPLE(B*(A+D)+P)
      | RNDSIMPLE(B*(A+D)+P+CARRYIN)
      | RNDSIMPLE(B*(A+D)+P>>17)
      | RNDSIMPLE(B*(A+D)+P>>17+CARRYIN)
      | RNDSIMPLE(B*(A+D)+PCIN)
      | RNDSIMPLE(B*(A+D)+PCIN+CARRYIN)
      | RNDSIMPLE(B*(A+D)+PCIN>>17)
      | RNDSIMPLE(B*(A+D)+PCIN>>17+CARRYIN)
      | RNDSIMPLE(B*(D+A))
      | RNDSIMPLE(B*(D+A)+C)
      | RNDSIMPLE(B*(D+A)+C+CARRYIN)
      | RNDSIMPLE(B*(D+A)+CARRYIN)
      | RNDSIMPLE(B*(D+A)+P)
      | RNDSIMPLE(B*(D+A)+P+CARRYIN)
      | RNDSIMPLE(B*(D+A)+P>>17)
      | RNDSIMPLE(B*(D+A)+P>>17+CARRYIN)
      | RNDSIMPLE(B*(D+A)+PCIN)
      | RNDSIMPLE(B*(D+A)+PCIN+CARRYIN)
      | RNDSIMPLE(B*(D+A)+PCIN>>17)
      | RNDSIMPLE(B*(D+A)+PCIN>>17+CARRYIN)
      | RNDSIMPLE(B*(D-A))
      | RNDSIMPLE(B*(D-A)+C)
      | RNDSIMPLE(B*(D-A)+C+CARRYIN)
      | RNDSIMPLE(B*(D-A)+CARRYIN)
      | RNDSIMPLE(B*(D-A)+P)
      | RNDSIMPLE(B*(D-A)+P+CARRYIN)
      | RNDSIMPLE(B*(D-A)+P>>17)
      | RNDSIMPLE(B*(D-A)+P>>17+CARRYIN)
      | RNDSIMPLE(B*(D-A)+PCIN)
      | RNDSIMPLE(B*(D-A)+PCIN+CARRYIN)
      | RNDSIMPLE(B*(D-A)+PCIN>>17)
      | RNDSIMPLE(B*(D-A)+PCIN>>17+CARRYIN)
      | RNDSIMPLE(B*A)
      | RNDSIMPLE(B*A+C)
      | RNDSIMPLE(B*A+C+CARRYIN)
      | RNDSIMPLE(B*A+CARRYIN)
      | RNDSIMPLE(B*A+P)
      | RNDSIMPLE(B*A+P+CARRYIN)
      | RNDSIMPLE(B*A+P>>17)
      | RNDSIMPLE(B*A+P>>17+CARRYIN)
      | RNDSIMPLE(B*A+PCIN)
      | RNDSIMPLE(B*A+PCIN+CARRYIN)
      | RNDSIMPLE(B*A+PCIN>>17)
      | RNDSIMPLE(B*A+PCIN>>17+CARRYIN)
      | RNDSIMPLE(B*D)
      | RNDSIMPLE(B*D+C)
      | RNDSIMPLE(B*D+C+CARRYIN)
      | RNDSIMPLE(B*D+CARRYIN)
      | RNDSIMPLE(B*D+P)
      | RNDSIMPLE(B*D+P+CARRYIN)
      | RNDSIMPLE(B*D+P>>17)
      | RNDSIMPLE(B*D+P>>17+CARRYIN)
      | RNDSIMPLE(B*D+PCIN)
      | RNDSIMPLE(B*D+PCIN+CARRYIN)
      | RNDSIMPLE(B*D+PCIN>>17)
      | RNDSIMPLE(B*D+PCIN>>17+CARRYIN)
      | RNDSIMPLE(C)
      | RNDSIMPLE(C+(A+D))
      | RNDSIMPLE(C+(A+D)*B)
      | RNDSIMPLE(C+(A+D)*B+CARRYIN)
      | RNDSIMPLE(C+(A+D)+CARRYIN)
      | RNDSIMPLE(C+(D+A))
      | RNDSIMPLE(C+(D+A)*B)
      | RNDSIMPLE(C+(D+A)*B+CARRYIN)
      | RNDSIMPLE(C+(D+A)+CARRYIN)
      | RNDSIMPLE(C+(D-A))
      | RNDSIMPLE(C+(D-A)*B)
      | RNDSIMPLE(C+(D-A)*B+CARRYIN)
      | RNDSIMPLE(C+(D-A)+CARRYIN)
      | RNDSIMPLE(C+A)
      | RNDSIMPLE(C+A*B)
      | RNDSIMPLE(C+A*B+CARRYIN)
      | RNDSIMPLE(C+A+CARRYIN)
      | RNDSIMPLE(C+B*(A+D))
      | RNDSIMPLE(C+B*(A+D)+CARRYIN)
      | RNDSIMPLE(C+B*(D+A))
      | RNDSIMPLE(C+B*(D+A)+CARRYIN)
      | RNDSIMPLE(C+B*(D-A))
      | RNDSIMPLE(C+B*(D-A)+CARRYIN)
      | RNDSIMPLE(C+B*A)
      | RNDSIMPLE(C+B*A+CARRYIN)
      | RNDSIMPLE(C+B*D)
      | RNDSIMPLE(C+B*D+CARRYIN)
      | RNDSIMPLE(C+C)
      | RNDSIMPLE(C+C+CARRYIN)
      | RNDSIMPLE(C+CARRYCASCIN)
      | RNDSIMPLE(C+CARRYIN)
      | RNDSIMPLE(C+D)
      | RNDSIMPLE(C+D*B)
      | RNDSIMPLE(C+D*B+CARRYIN)
      | RNDSIMPLE(C+D+CARRYIN)
      | RNDSIMPLE(C+P)
      | RNDSIMPLE(C+P+C)
      | RNDSIMPLE(C+P+C+CARRYIN)
      | RNDSIMPLE(C+P+CARRYIN)
      | RNDSIMPLE(CARRYIN)
      | RNDSIMPLE(D)
      | RNDSIMPLE(D*B)
      | RNDSIMPLE(D*B+C)
      | RNDSIMPLE(D*B+C+CARRYIN)
      | RNDSIMPLE(D*B+CARRYIN)
      | RNDSIMPLE(D*B+P)
      | RNDSIMPLE(D*B+P+CARRYIN)
      | RNDSIMPLE(D*B+P>>17)
      | RNDSIMPLE(D*B+P>>17+CARRYIN)
      | RNDSIMPLE(D*B+PCIN)
      | RNDSIMPLE(D*B+PCIN+CARRYIN)
      | RNDSIMPLE(D*B+PCIN>>17)
      | RNDSIMPLE(D*B+PCIN>>17+CARRYIN)
      | RNDSIMPLE(D+C)
      | RNDSIMPLE(D+C+CARRYIN)
      | RNDSIMPLE(D+CARRYIN)
      | RNDSIMPLE(D+P)
      | RNDSIMPLE(D+P+CARRYIN)
      | RNDSIMPLE(D+P>>17)
      | RNDSIMPLE(D+P>>17+CARRYIN)
      | RNDSIMPLE(D+PCIN)
      | RNDSIMPLE(D+PCIN+CARRYIN)
      | RNDSIMPLE(D+PCIN>>17)
      | RNDSIMPLE(D+PCIN>>17+CARRYIN)
      | RNDSIMPLE(P)
      | RNDSIMPLE(P+(A+D))
      | RNDSIMPLE(P+(A+D)*B)
      | RNDSIMPLE(P+(A+D)*B+CARRYIN)
      | RNDSIMPLE(P+(A+D)+CARRYIN)
      | RNDSIMPLE(P+(D+A))
      | RNDSIMPLE(P+(D+A)*B)
      | RNDSIMPLE(P+(D+A)*B+CARRYIN)
      | RNDSIMPLE(P+(D+A)+CARRYIN)
      | RNDSIMPLE(P+(D-A))
      | RNDSIMPLE(P+(D-A)*B)
      | RNDSIMPLE(P+(D-A)*B+CARRYIN)
      | RNDSIMPLE(P+(D-A)+CARRYIN)
      | RNDSIMPLE(P+A)
      | RNDSIMPLE(P+A*B)
      | RNDSIMPLE(P+A*B+CARRYIN)
      | RNDSIMPLE(P+A+CARRYIN)
      | RNDSIMPLE(P+B*(A+D))
      | RNDSIMPLE(P+B*(A+D)+CARRYIN)
      | RNDSIMPLE(P+B*(D+A))
      | RNDSIMPLE(P+B*(D+A)+CARRYIN)
      | RNDSIMPLE(P+B*(D-A))
      | RNDSIMPLE(P+B*(D-A)+CARRYIN)
      | RNDSIMPLE(P+B*A)
      | RNDSIMPLE(P+B*A+CARRYIN)
      | RNDSIMPLE(P+B*D)
      | RNDSIMPLE(P+B*D+CARRYIN)
      | RNDSIMPLE(P+C)
      | RNDSIMPLE(P+C+CARRYIN)
      | RNDSIMPLE(P+CARRYCASCIN)
      | RNDSIMPLE(P+CARRYIN)
      | RNDSIMPLE(P+D)
      | RNDSIMPLE(P+D*B)
      | RNDSIMPLE(P+D*B+CARRYIN)
      | RNDSIMPLE(P+D+CARRYIN)
      | RNDSIMPLE(P+P)
      | RNDSIMPLE(P+P+C)
      | RNDSIMPLE(P+P+C+CARRYIN)
      | RNDSIMPLE(P+P+CARRYIN)
      | RNDSIMPLE(P>>17)
      | RNDSIMPLE(P>>17+(A+D))
      | RNDSIMPLE(P>>17+(A+D)*B)
      | RNDSIMPLE(P>>17+(A+D)*B+CARRYIN)
      | RNDSIMPLE(P>>17+(A+D)+CARRYIN)
      | RNDSIMPLE(P>>17+(D+A))
      | RNDSIMPLE(P>>17+(D+A)*B)
      | RNDSIMPLE(P>>17+(D+A)*B+CARRYIN)
      | RNDSIMPLE(P>>17+(D+A)+CARRYIN)
      | RNDSIMPLE(P>>17+(D-A))
      | RNDSIMPLE(P>>17+(D-A)*B)
      | RNDSIMPLE(P>>17+(D-A)*B+CARRYIN)
      | RNDSIMPLE(P>>17+(D-A)+CARRYIN)
      | RNDSIMPLE(P>>17+A)
      | RNDSIMPLE(P>>17+A*B)
      | RNDSIMPLE(P>>17+A*B+CARRYIN)
      | RNDSIMPLE(P>>17+A+CARRYIN)
      | RNDSIMPLE(P>>17+B*(A+D))
      | RNDSIMPLE(P>>17+B*(A+D)+CARRYIN)
      | RNDSIMPLE(P>>17+B*(D+A))
      | RNDSIMPLE(P>>17+B*(D+A)+CARRYIN)
      | RNDSIMPLE(P>>17+B*(D-A))
      | RNDSIMPLE(P>>17+B*(D-A)+CARRYIN)
      | RNDSIMPLE(P>>17+B*A)
      | RNDSIMPLE(P>>17+B*A+CARRYIN)
      | RNDSIMPLE(P>>17+B*D)
      | RNDSIMPLE(P>>17+B*D+CARRYIN)
      | RNDSIMPLE(P>>17+C)
      | RNDSIMPLE(P>>17+C+CARRYIN)
      | RNDSIMPLE(P>>17+CARRYIN)
      | RNDSIMPLE(P>>17+D)
      | RNDSIMPLE(P>>17+D*B)
      | RNDSIMPLE(P>>17+D*B+CARRYIN)
      | RNDSIMPLE(P>>17+D+CARRYIN)
      | RNDSIMPLE(P>>17+P)
      | RNDSIMPLE(P>>17+P+C)
      | RNDSIMPLE(P>>17+P+C+CARRYIN)
      | RNDSIMPLE(P>>17+P+CARRYIN)
      | RNDSIMPLE(PCIN)
      | RNDSIMPLE(PCIN+(A+D))
      | RNDSIMPLE(PCIN+(A+D)*B)
      | RNDSIMPLE(PCIN+(A+D)*B+CARRYIN)
      | RNDSIMPLE(PCIN+(A+D)+CARRYIN)
      | RNDSIMPLE(PCIN+(D+A))
      | RNDSIMPLE(PCIN+(D+A)*B)
      | RNDSIMPLE(PCIN+(D+A)*B+CARRYIN)
      | RNDSIMPLE(PCIN+(D+A)+CARRYIN)
      | RNDSIMPLE(PCIN+(D-A))
      | RNDSIMPLE(PCIN+(D-A)*B)
      | RNDSIMPLE(PCIN+(D-A)*B+CARRYIN)
      | RNDSIMPLE(PCIN+(D-A)+CARRYIN)
      | RNDSIMPLE(PCIN+A)
      | RNDSIMPLE(PCIN+A*B)
      | RNDSIMPLE(PCIN+A*B+CARRYIN)
      | RNDSIMPLE(PCIN+A+CARRYIN)
      | RNDSIMPLE(PCIN+B*(A+D))
      | RNDSIMPLE(PCIN+B*(A+D)+CARRYIN)
      | RNDSIMPLE(PCIN+B*(D+A))
      | RNDSIMPLE(PCIN+B*(D+A)+CARRYIN)
      | RNDSIMPLE(PCIN+B*(D-A))
      | RNDSIMPLE(PCIN+B*(D-A)+CARRYIN)
      | RNDSIMPLE(PCIN+B*A)
      | RNDSIMPLE(PCIN+B*A+CARRYIN)
      | RNDSIMPLE(PCIN+B*D)
      | RNDSIMPLE(PCIN+B*D+CARRYIN)
      | RNDSIMPLE(PCIN+C)
      | RNDSIMPLE(PCIN+C+CARRYIN)
      | RNDSIMPLE(PCIN+CARRYIN)
      | RNDSIMPLE(PCIN+D)
      | RNDSIMPLE(PCIN+D*B)
      | RNDSIMPLE(PCIN+D*B+CARRYIN)
      | RNDSIMPLE(PCIN+D+CARRYIN)
      | RNDSIMPLE(PCIN+P)
      | RNDSIMPLE(PCIN+P+C)
      | RNDSIMPLE(PCIN+P+C+CARRYIN)
      | RNDSIMPLE(PCIN+P+CARRYIN)
      | RNDSIMPLE(PCIN>>17)
      | RNDSIMPLE(PCIN>>17+(A+D))
      | RNDSIMPLE(PCIN>>17+(A+D)*B)
      | RNDSIMPLE(PCIN>>17+(A+D)*B+CARRYIN)
      | RNDSIMPLE(PCIN>>17+(A+D)+CARRYIN)
      | RNDSIMPLE(PCIN>>17+(D+A))
      | RNDSIMPLE(PCIN>>17+(D+A)*B)
      | RNDSIMPLE(PCIN>>17+(D+A)*B+CARRYIN)
      | RNDSIMPLE(PCIN>>17+(D+A)+CARRYIN)
      | RNDSIMPLE(PCIN>>17+(D-A))
      | RNDSIMPLE(PCIN>>17+(D-A)*B)
      | RNDSIMPLE(PCIN>>17+(D-A)*B+CARRYIN)
      | RNDSIMPLE(PCIN>>17+(D-A)+CARRYIN)
      | RNDSIMPLE(PCIN>>17+A)
      | RNDSIMPLE(PCIN>>17+A*B)
      | RNDSIMPLE(PCIN>>17+A*B+CARRYIN)
      | RNDSIMPLE(PCIN>>17+A+CARRYIN)
      | RNDSIMPLE(PCIN>>17+B*(A+D))
      | RNDSIMPLE(PCIN>>17+B*(A+D)+CARRYIN)
      | RNDSIMPLE(PCIN>>17+B*(D+A))
      | RNDSIMPLE(PCIN>>17+B*(D+A)+CARRYIN)
      | RNDSIMPLE(PCIN>>17+B*(D-A))
      | RNDSIMPLE(PCIN>>17+B*(D-A)+CARRYIN)
      | RNDSIMPLE(PCIN>>17+B*A)
      | RNDSIMPLE(PCIN>>17+B*A+CARRYIN)
      | RNDSIMPLE(PCIN>>17+B*D)
      | RNDSIMPLE(PCIN>>17+B*D+CARRYIN)
      | RNDSIMPLE(PCIN>>17+C)
      | RNDSIMPLE(PCIN>>17+C+CARRYIN)
      | RNDSIMPLE(PCIN>>17+CARRYIN)
      | RNDSIMPLE(PCIN>>17+D)
      | RNDSIMPLE(PCIN>>17+D*B)
      | RNDSIMPLE(PCIN>>17+D*B+CARRYIN)
      | RNDSIMPLE(PCIN>>17+D+CARRYIN)
      | RNDSIMPLE(PCIN>>17+P)
      | RNDSIMPLE(PCIN>>17+P+C)
      | RNDSIMPLE(PCIN>>17+P+C+CARRYIN)
      | RNDSIMPLE(PCIN>>17+P+CARRYIN)
      | RNDSYM((A+D))
      | RNDSYM((A+D)*B)
      | RNDSYM((D+A))
      | RNDSYM((D+A)*B)
      | RNDSYM((D-A))
      | RNDSYM((D-A)*B)
      | RNDSYM(A)
      | RNDSYM(A*B)
      | RNDSYM(B*(A+D))
      | RNDSYM(B*(D+A))
      | RNDSYM(B*(D-A))
      | RNDSYM(B*A)
      | RNDSYM(B*D)
      | RNDSYM(D)
      | RNDSYM(D*B)
      | RNDSYM(P)
      | RNDSYM(PCIN)
      settings: infoedit=<html>Valid operands: CONCAT, P, C, PCIN, P>>17, PCIN>>17, CARRYIN, CARRYCASCIN, ACIN, A, BCIN,B<br><br>Valid operators: +, -, *, ()<br><br>Valid functions: RNDSIMPLE, RNDSYM<br><br>Instructions are case insensitive and tolerate spaces.</html>
